simulink model "cubli_XYZ_extensive_simulations"  (R2016a)
(part 4 of 9)

  1/2).*t.*theta)).*(q02.*sin((1/2).*(1+(-1).*t).*theta)+q12.*sin((1/2).* ...
  t.*theta))+csc((1/2).*theta).^2.*(q03.*sin((1/2).*(1+(-1).*t).*theta)+ ...
  q13.*sin((1/2).*t.*theta)).*(q04.*sin((1/2).*(1+(-1).*t).*theta)+q14.* ...
  sin((1/2).*t.*theta)))+(-4).*(2.*((-1/2).*q02.*theta.*cos((1/2).*(1+(-1) ...
  .*t).*theta)+(1/2).*q12.*theta.*cos((1/2).*t.*theta)).*csc((1/2).*theta) ...
  .^2.*(q02.*sin((1/2).*(1+(-1).*t).*theta)+q12.*sin((1/2).*t.*theta))+2.* ...
  ((-1/2).*q03.*theta.*cos((1/2).*(1+(-1).*t).*theta)+(1/2).*q13.*theta.* ...
  cos((1/2).*t.*theta)).*csc((1/2).*theta).^2.*(q03.*sin((1/2).*(1+(-1).* ...
  t).*theta)+q13.*sin((1/2).*t.*theta))).*(1+(-2).*(csc((1/2).*theta).^2.* ...
  (q02.*sin((1/2).*(1+(-1).*t).*theta)+q12.*sin((1/2).*t.*theta)).^2+csc(( ...
  1/2).*theta).^2.*(q03.*sin((1/2).*(1+(-1).*t).*theta)+q13.*sin((1/2).* ...
  t.*theta)).^2))).*(4.*((-1).*csc((1/2).*theta).^2.*(q01.*sin((1/2).*(1+( ...
  -1).*t).*theta)+q11.*sin((1/2).*t.*theta)).*(q02.*sin((1/2).*(1+(-1).*t) ...
  .*theta)+q12.*sin((1/2).*t.*theta))+csc((1/2).*theta).^2.*(q03.*sin(( ...
  1/2).*(1+(-1).*t).*theta)+q13.*sin((1/2).*t.*theta)).*(q04.*sin((1/2).*( ...
  1+(-1).*t).*theta)+q14.*sin((1/2).*t.*theta))).^2+(1+(-2).*(csc((1/2).* ...
  theta).^2.*(q02.*sin((1/2).*(1+(-1).*t).*theta)+q12.*sin((1/2).*t.* ...
  theta)).^2+csc((1/2).*theta).^2.*(q03.*sin((1/2).*(1+(-1).*t).*theta)+ ...
  q13.*sin((1/2).*t.*theta)).^2)).^2).^(-1/2).*(4.*(csc((1/2).*theta).^2.* ...
  (q01.*sin((1/2).*(1+(-1).*t).*theta)+q11.*sin((1/2).*t.*theta)).*(q03.* ...
  sin((1/2).*(1+(-1).*t).*theta)+q13.*sin((1/2).*t.*theta))+csc((1/2).* ...
  theta).^2.*(q02.*sin((1/2).*(1+(-1).*t).*theta)+q12.*sin((1/2).*t.* ...
  theta)).*(q04.*sin((1/2).*(1+(-1).*t).*theta)+q14.*sin((1/2).*t.*theta)) ...
  ).^2+4.*((-1).*csc((1/2).*theta).^2.*(q01.*sin((1/2).*(1+(-1).*t).* ...
  theta)+q11.*sin((1/2).*t.*theta)).*(q02.*sin((1/2).*(1+(-1).*t).*theta)+ ...
  q12.*sin((1/2).*t.*theta))+csc((1/2).*theta).^2.*(q03.*sin((1/2).*(1+( ...
  -1).*t).*theta)+q13.*sin((1/2).*t.*theta)).*(q04.*sin((1/2).*(1+(-1).*t) ...
  .*theta)+q14.*sin((1/2).*t.*theta))).^2+(1+(-2).*(csc((1/2).*theta).^2.* ...
  (q02.*sin((1/2).*(1+(-1).*t).*theta)+q12.*sin((1/2).*t.*theta)).^2+csc(( ...
  1/2).*theta).^2.*(q03.*sin((1/2).*(1+(-1).*t).*theta)+q13.*sin((1/2).* ...
  t.*theta)).^2)).^2).^(-1/2)+(csc((1/2).*theta).^2.*(q02.*sin((1/2).*(1+( ...
  -1).*t).*theta)+q12.*sin((1/2).*t.*theta)).*(q03.*sin((1/2).*(1+(-1).*t) ...
  .*theta)+q13.*sin((1/2).*t.*theta))+(-1).*csc((1/2).*theta).^2.*(q01.* ...
  sin((1/2).*(1+(-1).*t).*theta)+q11.*sin((1/2).*t.*theta)).*(q04.*sin(( ...
  1/2).*(1+(-1).*t).*theta)+q14.*sin((1/2).*t.*theta))).*(8.*((-1).*(( ...
  -1/2).*q02.*theta.*cos((1/2).*(1+(-1).*t).*theta)+(1/2).*q12.*theta.* ...
  cos((1/2).*t.*theta)).*csc((1/2).*theta).^2.*(q01.*sin((1/2).*(1+(-1).* ...
  t).*theta)+q11.*sin((1/2).*t.*theta))+(-1).*((-1/2).*q01.*theta.*cos(( ...
  1/2).*(1+(-1).*t).*theta)+(1/2).*q11.*theta.*cos((1/2).*t.*theta)).*csc( ...
  (1/2).*theta).^2.*(q02.*sin((1/2).*(1+(-1).*t).*theta)+q12.*sin((1/2).* ...
  t.*theta))+((-1/2).*q04.*theta.*cos((1/2).*(1+(-1).*t).*theta)+(1/2).* ...
  q14.*theta.*cos((1/2).*t.*theta)).*csc((1/2).*theta).^2.*(q03.*sin((1/2) ...
  .*(1+(-1).*t).*theta)+q13.*sin((1/2).*t.*theta))+((-1/2).*q03.*theta.* ...
  cos((1/2).*(1+(-1).*t).*theta)+(1/2).*q13.*theta.*cos((1/2).*t.*theta)) ...
  .*csc((1/2).*theta).^2.*(q04.*sin((1/2).*(1+(-1).*t).*theta)+q14.*sin(( ...
  1/2).*t.*theta))).*((-1).*csc((1/2).*theta).^2.*(q01.*sin((1/2).*(1+(-1) ...
  .*t).*theta)+q11.*sin((1/2).*t.*theta)).*(q02.*sin((1/2).*(1+(-1).*t).* ...
  theta)+q12.*sin((1/2).*t.*theta))+csc((1/2).*theta).^2.*(q03.*sin((1/2) ...
  .*(1+(-1).*t).*theta)+q13.*sin((1/2).*t.*theta)).*(q04.*sin((1/2).*(1+( ...
  -1).*t).*theta)+q14.*sin((1/2).*t.*theta)))+(-4).*(2.*((-1/2).*q02.* ...
  theta.*cos((1/2).*(1+(-1).*t).*theta)+(1/2).*q12.*theta.*cos((1/2).*t.* ...
  theta)).*csc((1/2).*theta).^2.*(q02.*sin((1/2).*(1+(-1).*t).*theta)+ ...
  q12.*sin((1/2).*t.*theta))+2.*((-1/2).*q03.*theta.*cos((1/2).*(1+(-1).* ...
  t).*theta)+(1/2).*q13.*theta.*cos((1/2).*t.*theta)).*csc((1/2).*theta) ...
  .^2.*(q03.*sin((1/2).*(1+(-1).*t).*theta)+q13.*sin((1/2).*t.*theta))).*( ...
  1+(-2).*(csc((1/2).*theta).^2.*(q02.*sin((1/2).*(1+(-1).*t).*theta)+ ...
  q12.*sin((1/2).*t.*theta)).^2+csc((1/2).*theta).^2.*(q03.*sin((1/2).*(1+ ...
  (-1).*t).*theta)+q13.*sin((1/2).*t.*theta)).^2))).*(4.*((-1).*csc((1/2) ...
  .*theta).^2.*(q01.*sin((1/2).*(1+(-1).*t).*theta)+q11.*sin((1/2).*t.* ...
  theta)).*(q02.*sin((1/2).*(1+(-1).*t).*theta)+q12.*sin((1/2).*t.*theta)) ...
  +csc((1/2).*theta).^2.*(q03.*sin((1/2).*(1+(-1).*t).*theta)+q13.*sin(( ...
  1/2).*t.*theta)).*(q04.*sin((1/2).*(1+(-1).*t).*theta)+q14.*sin((1/2).* ...
  t.*theta))).^2+(1+(-2).*(csc((1/2).*theta).^2.*(q02.*sin((1/2).*(1+(-1) ...
  .*t).*theta)+q12.*sin((1/2).*t.*theta)).^2+csc((1/2).*theta).^2.*(q03.* ...
  sin((1/2).*(1+(-1).*t).*theta)+q13.*sin((1/2).*t.*theta)).^2)).^2).^( ...
  -3/2).*(4.*(csc((1/2).*theta).^2.*(q01.*sin((1/2).*(1+(-1).*t).*theta)+ ...
  q11.*sin((1/2).*t.*theta)).*(q03.*sin((1/2).*(1+(-1).*t).*theta)+q13.* ...
  sin((1/2).*t.*theta))+csc((1/2).*theta).^2.*(q02.*sin((1/2).*(1+(-1).*t) ...
  .*theta)+q12.*sin((1/2).*t.*theta)).*(q04.*sin((1/2).*(1+(-1).*t).* ...
  theta)+q14.*sin((1/2).*t.*theta))).^2+4.*((-1).*csc((1/2).*theta).^2.*( ...
  q01.*sin((1/2).*(1+(-1).*t).*theta)+q11.*sin((1/2).*t.*theta)).*(q02.* ...
  sin((1/2).*(1+(-1).*t).*theta)+q12.*sin((1/2).*t.*theta))+csc((1/2).* ...
  theta).^2.*(q03.*sin((1/2).*(1+(-1).*t).*theta)+q13.*sin((1/2).*t.* ...
  theta)).*(q04.*sin((1/2).*(1+(-1).*t).*theta)+q14.*sin((1/2).*t.*theta)) ...
  ).^2+(1+(-2).*(csc((1/2).*theta).^2.*(q02.*sin((1/2).*(1+(-1).*t).* ...
  theta)+q12.*sin((1/2).*t.*theta)).^2+csc((1/2).*theta).^2.*(q03.*sin(( ...
  1/2).*(1+(-1).*t).*theta)+q13.*sin((1/2).*t.*theta)).^2)).^2).^(1/2)+( ...
  -2).*((-1).*((-1/2).*q04.*theta.*cos((1/2).*(1+(-1).*t).*theta)+(1/2).* ...
  q14.*theta.*cos((1/2).*t.*theta)).*csc((1/2).*theta).^2.*(q01.*sin((1/2) ...
  .*(1+(-1).*t).*theta)+q11.*sin((1/2).*t.*theta))+((-1/2).*q03.*theta.* ...
  cos((1/2).*(1+(-1).*t).*theta)+(1/2).*q13.*theta.*cos((1/2).*t.*theta)) ...
  .*csc((1/2).*theta).^2.*(q02.*sin((1/2).*(1+(-1).*t).*theta)+q12.*sin(( ...
  1/2).*t.*theta))+((-1/2).*q02.*theta.*cos((1/2).*(1+(-1).*t).*theta)+( ...
  1/2).*q12.*theta.*cos((1/2).*t.*theta)).*csc((1/2).*theta).^2.*(q03.* ...
  sin((1/2).*(1+(-1).*t).*theta)+q13.*sin((1/2).*t.*theta))+(-1).*((-1/2) ...
  .*q01.*theta.*cos((1/2).*(1+(-1).*t).*theta)+(1/2).*q11.*theta.*cos(( ...
  1/2).*t.*theta)).*csc((1/2).*theta).^2.*(q04.*sin((1/2).*(1+(-1).*t).* ...
  theta)+q14.*sin((1/2).*t.*theta))).*(4.*((-1).*csc((1/2).*theta).^2.*( ...
  q01.*sin((1/2).*(1+(-1).*t).*theta)+q11.*sin((1/2).*t.*theta)).*(q02.* ...
  sin((1/2).*(1+(-1).*t).*theta)+q12.*sin((1/2).*t.*theta))+csc((1/2).* ...
  theta).^2.*(q03.*sin((1/2).*(1+(-1).*t).*theta)+q13.*sin((1/2).*t.* ...
  theta)).*(q04.*sin((1/2).*(1+(-1).*t).*theta)+q14.*sin((1/2).*t.*theta)) ...
  ).^2+(1+(-2).*(csc((1/2).*theta).^2.*(q02.*sin((1/2).*(1+(-1).*t).* ...
  theta)+q12.*sin((1/2).*t.*theta)).^2+csc((1/2).*theta).^2.*(q03.*sin(( ...
  1/2).*(1+(-1).*t).*theta)+q13.*sin((1/2).*t.*theta)).^2)).^2).^(-1/2).*( ...
  4.*(csc((1/2).*theta).^2.*(q01.*sin((1/2).*(1+(-1).*t).*theta)+q11.*sin( ...
  (1/2).*t.*theta)).*(q03.*sin((1/2).*(1+(-1).*t).*theta)+q13.*sin((1/2).* ...
  t.*theta))+csc((1/2).*theta).^2.*(q02.*sin((1/2).*(1+(-1).*t).*theta)+ ...
  q12.*sin((1/2).*t.*theta)).*(q04.*sin((1/2).*(1+(-1).*t).*theta)+q14.* ...
  sin((1/2).*t.*theta))).^2+4.*((-1).*csc((1/2).*theta).^2.*(q01.*sin(( ...
  1/2).*(1+(-1).*t).*theta)+q11.*sin((1/2).*t.*theta)).*(q02.*sin((1/2).*( ...
  1+(-1).*t).*theta)+q12.*sin((1/2).*t.*theta))+csc((1/2).*theta).^2.*( ...
  q03.*sin((1/2).*(1+(-1).*t).*theta)+q13.*sin((1/2).*t.*theta)).*(q04.* ...
  sin((1/2).*(1+(-1).*t).*theta)+q14.*sin((1/2).*t.*theta))).^2+(1+(-2).*( ...
  csc((1/2).*theta).^2.*(q02.*sin((1/2).*(1+(-1).*t).*theta)+q12.*sin(( ...
  1/2).*t.*theta)).^2+csc((1/2).*theta).^2.*(q03.*sin((1/2).*(1+(-1).*t).* ...
  theta)+q13.*sin((1/2).*t.*theta)).^2)).^2).^(1/2)).*(4.*(csc((1/2).* ...
  theta).^2.*(q02.*sin((1/2).*(1+(-1).*t).*theta)+q12.*sin((1/2).*t.* ...
  theta)).*(q03.*sin((1/2).*(1+(-1).*t).*theta)+q13.*sin((1/2).*t.*theta)) ...
  +(-1).*csc((1/2).*theta).^2.*(q01.*sin((1/2).*(1+(-1).*t).*theta)+q11.* ...
  sin((1/2).*t.*theta)).*(q04.*sin((1/2).*(1+(-1).*t).*theta)+q14.*sin(( ...
  1/2).*t.*theta))).^2.*(4.*((-1).*csc((1/2).*theta).^2.*(q01.*sin((1/2).* ...
  (1+(-1).*t).*theta)+q11.*sin((1/2).*t.*theta)).*(q02.*sin((1/2).*(1+(-1) ...
  .*t).*theta)+q12.*sin((1/2).*t.*theta))+csc((1/2).*theta).^2.*(q03.*sin( ...
  (1/2).*(1+(-1).*t).*theta)+q13.*sin((1/2).*t.*theta)).*(q04.*sin((1/2).* ...
  (1+(-1).*t).*theta)+q14.*sin((1/2).*t.*theta))).^2+(1+(-2).*(csc((1/2).* ...
  theta).^2.*(q02.*sin((1/2).*(1+(-1).*t).*theta)+q12.*sin((1/2).*t.* ...
  theta)).^2+csc((1/2).*theta).^2.*(q03.*sin((1/2).*(1+(-1).*t).*theta)+ ...
  q13.*sin((1/2).*t.*theta)).^2)).^2).^(-1).*(4.*(csc((1/2).*theta).^2.*( ...
  q01.*sin((1/2).*(1+(-1).*t).*theta)+q11.*sin((1/2).*t.*theta)).*(q03.* ...
  sin((1/2).*(1+(-1).*t).*theta)+q13.*sin((1/2).*t.*theta))+csc((1/2).* ...
  theta).^2.*(q02.*sin((1/2).*(1+(-1).*t).*theta)+q12.*sin((1/2).*t.* ...
  theta)).*(q04.*sin((1/2).*(1+(-1).*t).*theta)+q14.*sin((1/2).*t.*theta)) ...
  ).^2+4.*((-1).*csc((1/2).*theta).^2.*(q01.*sin((1/2).*(1+(-1).*t).* ...
  theta)+q11.*sin((1/2).*t.*theta)).*(q02.*sin((1/2).*(1+(-1).*t).*theta)+ ...
  q12.*sin((1/2).*t.*theta))+csc((1/2).*theta).^2.*(q03.*sin((1/2).*(1+( ...
  -1).*t).*theta)+q13.*sin((1/2).*t.*theta)).*(q04.*sin((1/2).*(1+(-1).*t) ...
  .*theta)+q14.*sin((1/2).*t.*theta))).^2+(1+(-2).*(csc((1/2).*theta).^2.* ...
  (q02.*sin((1/2).*(1+(-1).*t).*theta)+q12.*sin((1/2).*t.*theta)).^2+csc(( ...
  1/2).*theta).^2.*(q03.*sin((1/2).*(1+(-1).*t).*theta)+q13.*sin((1/2).* ...
  t.*theta)).^2)).^2)+(1+(-2).*(csc((1/2).*theta).^2.*(q03.*sin((1/2).*(1+ ...
  (-1).*t).*theta)+q13.*sin((1/2).*t.*theta)).^2+csc((1/2).*theta).^2.*( ...
  q04.*sin((1/2).*(1+(-1).*t).*theta)+q14.*sin((1/2).*t.*theta)).^2)).^2.* ...
  (4.*((-1).*csc((1/2).*theta).^2.*(q01.*sin((1/2).*(1+(-1).*t).*theta)+ ...
  q11.*sin((1/2).*t.*theta)).*(q02.*sin((1/2).*(1+(-1).*t).*theta)+q12.* ...
  sin((1/2).*t.*theta))+csc((1/2).*theta).^2.*(q03.*sin((1/2).*(1+(-1).*t) ...
  .*theta)+q13.*sin((1/2).*t.*theta)).*(q04.*sin((1/2).*(1+(-1).*t).* ...
  theta)+q14.*sin((1/2).*t.*theta))).^2+(1+(-2).*(csc((1/2).*theta).^2.*( ...
  q02.*sin((1/2).*(1+(-1).*t).*theta)+q12.*sin((1/2).*t.*theta)).^2+csc(( ...
  1/2).*theta).^2.*(q03.*sin((1/2).*(1+(-1).*t).*theta)+q13.*sin((1/2).* ...
  t.*theta)).^2)).^2).^(-1).*(4.*(csc((1/2).*theta).^2.*(q01.*sin((1/2).*( ...
  1+(-1).*t).*theta)+q11.*sin((1/2).*t.*theta)).*(q03.*sin((1/2).*(1+(-1) ...
  .*t).*theta)+q13.*sin((1/2).*t.*theta))+csc((1/2).*theta).^2.*(q02.*sin( ...
  (1/2).*(1+(-1).*t).*theta)+q12.*sin((1/2).*t.*theta)).*(q04.*sin((1/2).* ...
  (1+(-1).*t).*theta)+q14.*sin((1/2).*t.*theta))).^2+4.*((-1).*csc((1/2).* ...
  theta).^2.*(q01.*sin((1/2).*(1+(-1).*t).*theta)+q11.*sin((1/2).*t.* ...
  theta)).*(q02.*sin((1/2).*(1+(-1).*t).*theta)+q12.*sin((1/2).*t.*theta)) ...
  +csc((1/2).*theta).^2.*(q03.*sin((1/2).*(1+(-1).*t).*theta)+q13.*sin(( ...
  1/2).*t.*theta)).*(q04.*sin((1/2).*(1+(-1).*t).*theta)+q14.*sin((1/2).* ...
  t.*theta))).^2+(1+(-2).*(csc((1/2).*theta).^2.*(q02.*sin((1/2).*(1+(-1) ...
  .*t).*theta)+q12.*sin((1/2).*t.*theta)).^2+csc((1/2).*theta).^2.*(q03.* ...
  sin((1/2).*(1+(-1).*t).*theta)+q13.*sin((1/2).*t.*theta)).^2)).^2)).^( ...
  -1)+(-1/2).*(1+(-2).*(csc((1/2).*theta).^2.*(q03.*sin((1/2).*(1+(-1).*t) ...
  .*theta)+q13.*sin((1/2).*t.*theta)).^2+csc((1/2).*theta).^2.*(q04.*sin(( ...
  1/2).*(1+(-1).*t).*theta)+q14.*sin((1/2).*t.*theta)).^2)).*(8.*((-1).*(( ...
  -1/2).*q02.*theta.*cos((1/2).*(1+(-1).*t).*theta)+(1/2).*q12.*theta.* ...
  cos((1/2).*t.*theta)).*csc((1/2).*theta).^2.*(q01.*sin((1/2).*(1+(-1).* ...
  t).*theta)+q11.*sin((1/2).*t.*theta))+(-1).*((-1/2).*q01.*theta.*cos(( ...
  1/2).*(1+(-1).*t).*theta)+(1/2).*q11.*theta.*cos((1/2).*t.*theta)).*csc( ...
  (1/2).*theta).^2.*(q02.*sin((1/2).*(1+(-1).*t).*theta)+q12.*sin((1/2).* ...
  t.*theta))+((-1/2).*q04.*theta.*cos((1/2).*(1+(-1).*t).*theta)+(1/2).* ...
  q14.*theta.*cos((1/2).*t.*theta)).*csc((1/2).*theta).^2.*(q03.*sin((1/2) ...
  .*(1+(-1).*t).*theta)+q13.*sin((1/2).*t.*theta))+((-1/2).*q03.*theta.* ...
  cos((1/2).*(1+(-1).*t).*theta)+(1/2).*q13.*theta.*cos((1/2).*t.*theta)) ...
  .*csc((1/2).*theta).^2.*(q04.*sin((1/2).*(1+(-1).*t).*theta)+q14.*sin(( ...
  1/2).*t.*theta))).*((-1).*csc((1/2).*theta).^2.*(q01.*sin((1/2).*(1+(-1) ...
  .*t).*theta)+q11.*sin((1/2).*t.*theta)).*(q02.*sin((1/2).*(1+(-1).*t).* ...
  theta)+q12.*sin((1/2).*t.*theta))+csc((1/2).*theta).^2.*(q03.*sin((1/2) ...
  .*(1+(-1).*t).*theta)+q13.*sin((1/2).*t.*theta)).*(q04.*sin((1/2).*(1+( ...
  -1).*t).*theta)+q14.*sin((1/2).*t.*theta)))+(-4).*(2.*((-1/2).*q02.* ...
  theta.*cos((1/2).*(1+(-1).*t).*theta)+(1/2).*q12.*theta.*cos((1/2).*t.* ...
  theta)).*csc((1/2).*theta).^2.*(q02.*sin((1/2).*(1+(-1).*t).*theta)+ ...
  q12.*sin((1/2).*t.*theta))+2.*((-1/2).*q03.*theta.*cos((1/2).*(1+(-1).* ...
  t).*theta)+(1/2).*q13.*theta.*cos((1/2).*t.*theta)).*csc((1/2).*theta) ...
  .^2.*(q03.*sin((1/2).*(1+(-1).*t).*theta)+q13.*sin((1/2).*t.*theta))).*( ...
  1+(-2).*(csc((1/2).*theta).^2.*(q02.*sin((1/2).*(1+(-1).*t).*theta)+ ...
  q12.*sin((1/2).*t.*theta)).^2+csc((1/2).*theta).^2.*(q03.*sin((1/2).*(1+ ...
  (-1).*t).*theta)+q13.*sin((1/2).*t.*theta)).^2))).*(4.*((-1).*csc((1/2) ...
  .*theta).^2.*(q01.*sin((1/2).*(1+(-1).*t).*theta)+q11.*sin((1/2).*t.* ...
  theta)).*(q02.*sin((1/2).*(1+(-1).*t).*theta)+q12.*sin((1/2).*t.*theta)) ...
  +csc((1/2).*theta).^2.*(q03.*sin((1/2).*(1+(-1).*t).*theta)+q13.*sin(( ...
  1/2).*t.*theta)).*(q04.*sin((1/2).*(1+(-1).*t).*theta)+q14.*sin((1/2).* ...
  t.*theta))).^2+(1+(-2).*(csc((1/2).*theta).^2.*(q02.*sin((1/2).*(1+(-1) ...
  .*t).*theta)+q12.*sin((1/2).*t.*theta)).^2+csc((1/2).*theta).^2.*(q03.* ...
  sin((1/2).*(1+(-1).*t).*theta)+q13.*sin((1/2).*t.*theta)).^2)).^2).^( ...
  -3/2).*(4.*(csc((1/2).*theta).^2.*(q01.*sin((1/2).*(1+(-1).*t).*theta)+ ...
  q11.*sin((1/2).*t.*theta)).*(q03.*sin((1/2).*(1+(-1).*t).*theta)+q13.* ...
  sin((1/2).*t.*theta))+csc((1/2).*theta).^2.*(q02.*sin((1/2).*(1+(-1).*t) ...
  .*theta)+q12.*sin((1/2).*t.*theta)).*(q04.*sin((1/2).*(1+(-1).*t).* ...
  theta)+q14.*sin((1/2).*t.*theta))).^2+4.*((-1).*csc((1/2).*theta).^2.*( ...
  q01.*sin((1/2).*(1+(-1).*t).*theta)+q11.*sin((1/2).*t.*theta)).*(q02.* ...
  sin((1/2).*(1+(-1).*t).*theta)+q12.*sin((1/2).*t.*theta))+csc((1/2).* ...
  theta).^2.*(q03.*sin((1/2).*(1+(-1).*t).*theta)+q13.*sin((1/2).*t.* ...
  theta)).*(q04.*sin((1/2).*(1+(-1).*t).*theta)+q14.*sin((1/2).*t.*theta)) ...
  ).^2+(1+(-2).*(csc((1/2).*theta).^2.*(q02.*sin((1/2).*(1+(-1).*t).* ...
  theta)+q12.*sin((1/2).*t.*theta)).^2+csc((1/2).*theta).^2.*(q03.*sin(( ...
  1/2).*(1+(-1).*t).*theta)+q13.*sin((1/2).*t.*theta)).^2)).^2).^(1/2).*(( ...
  -1).*(csc((1/2).*theta).^2.*(q02.*sin((1/2).*(1+(-1).*t).*theta)+q12.* ...
  sin((1/2).*t.*theta)).*(q03.*sin((1/2).*(1+(-1).*t).*theta)+q13.*sin(( ...
  1/2).*t.*theta))+(-1).*csc((1/2).*theta).^2.*(q01.*sin((1/2).*(1+(-1).* ...
  t).*theta)+q11.*sin((1/2).*t.*theta)).*(q04.*sin((1/2).*(1+(-1).*t).* ...
  theta)+q14.*sin((1/2).*t.*theta))).*(8.*(((-1/2).*q03.*theta.*cos((1/2) ...
  .*(1+(-1).*t).*theta)+(1/2).*q13.*theta.*cos((1/2).*t.*theta)).*csc(( ...
  1/2).*theta).^2.*(q01.*sin((1/2).*(1+(-1).*t).*theta)+q11.*sin((1/2).* ...
  t.*theta))+((-1/2).*q04.*theta.*cos((1/2).*(1+(-1).*t).*theta)+(1/2).* ...
  q14.*theta.*cos((1/2).*t.*theta)).*csc((1/2).*theta).^2.*(q02.*sin((1/2) ...
  .*(1+(-1).*t).*theta)+q12.*sin((1/2).*t.*theta))+((-1/2).*q01.*theta.* ...
  cos((1/2).*(1+(-1).*t).*theta)+(1/2).*q11.*theta.*cos((1/2).*t.*theta)) ...
  .*csc((1/2).*theta).^2.*(q03.*sin((1/2).*(1+(-1).*t).*theta)+q13.*sin(( ...
  1/2).*t.*theta))+((-1/2).*q02.*theta.*cos((1/2).*(1+(-1).*t).*theta)+( ...
  1/2).*q12.*theta.*cos((1/2).*t.*theta)).*csc((1/2).*theta).^2.*(q04.* ...
  sin((1/2).*(1+(-1).*t).*theta)+q14.*sin((1/2).*t.*theta))).*(csc((1/2).* ...
  theta).^2.*(q01.*sin((1/2).*(1+(-1).*t).*theta)+q11.*sin((1/2).*t.* ...
  theta)).*(q03.*sin((1/2).*(1+(-1).*t).*theta)+q13.*sin((1/2).*t.*theta)) ...
  +csc((1/2).*theta).^2.*(q02.*sin((1/2).*(1+(-1).*t).*theta)+q12.*sin(( ...
  1/2).*t.*theta)).*(q04.*sin((1/2).*(1+(-1).*t).*theta)+q14.*sin((1/2).* ...
  t.*theta)))+8.*((-1).*((-1/2).*q02.*theta.*cos((1/2).*(1+(-1).*t).* ...
  theta)+(1/2).*q12.*theta.*cos((1/2).*t.*theta)).*csc((1/2).*theta).^2.*( ...
  q01.*sin((1/2).*(1+(-1).*t).*theta)+q11.*sin((1/2).*t.*theta))+(-1).*(( ...
  -1/2).*q01.*theta.*cos((1/2).*(1+(-1).*t).*theta)+(1/2).*q11.*theta.* ...
  cos((1/2).*t.*theta)).*csc((1/2).*theta).^2.*(q02.*sin((1/2).*(1+(-1).* ...
  t).*theta)+q12.*sin((1/2).*t.*theta))+((-1/2).*q04.*theta.*cos((1/2).*( ...
  1+(-1).*t).*theta)+(1/2).*q14.*theta.*cos((1/2).*t.*theta)).*csc((1/2).* ...
  theta).^2.*(q03.*sin((1/2).*(1+(-1).*t).*theta)+q13.*sin((1/2).*t.* ...
  theta))+((-1/2).*q03.*theta.*cos((1/2).*(1+(-1).*t).*theta)+(1/2).*q13.* ...
  theta.*cos((1/2).*t.*theta)).*csc((1/2).*theta).^2.*(q04.*sin((1/2).*(1+ ...
  (-1).*t).*theta)+q14.*sin((1/2).*t.*theta))).*((-1).*csc((1/2).*theta) ...
  .^2.*(q01.*sin((1/2).*(1+(-1).*t).*theta)+q11.*sin((1/2).*t.*theta)).*( ...
  q02.*sin((1/2).*(1+(-1).*t).*theta)+q12.*sin((1/2).*t.*theta))+csc((1/2) ...
  .*theta).^2.*(q03.*sin((1/2).*(1+(-1).*t).*theta)+q13.*sin((1/2).*t.* ...
  theta)).*(q04.*sin((1/2).*(1+(-1).*t).*theta)+q14.*sin((1/2).*t.*theta)) ...
  )+(-4).*(2.*((-1/2).*q02.*theta.*cos((1/2).*(1+(-1).*t).*theta)+(1/2).* ...
  q12.*theta.*cos((1/2).*t.*theta)).*csc((1/2).*theta).^2.*(q02.*sin((1/2) ...
  .*(1+(-1).*t).*theta)+q12.*sin((1/2).*t.*theta))+2.*((-1/2).*q03.* ...
  theta.*cos((1/2).*(1+(-1).*t).*theta)+(1/2).*q13.*theta.*cos((1/2).*t.* ...
  theta)).*csc((1/2).*theta).^2.*(q03.*sin((1/2).*(1+(-1).*t).*theta)+ ...
  q13.*sin((1/2).*t.*theta))).*(1+(-2).*(csc((1/2).*theta).^2.*(q02.*sin(( ...
  1/2).*(1+(-1).*t).*theta)+q12.*sin((1/2).*t.*theta)).^2+csc((1/2).* ...
  theta).^2.*(q03.*sin((1/2).*(1+(-1).*t).*theta)+q13.*sin((1/2).*t.* ...
  theta)).^2))).*(4.*((-1).*csc((1/2).*theta).^2.*(q01.*sin((1/2).*(1+(-1) ...
  .*t).*theta)+q11.*sin((1/2).*t.*theta)).*(q02.*sin((1/2).*(1+(-1).*t).* ...
  theta)+q12.*sin((1/2).*t.*theta))+csc((1/2).*theta).^2.*(q03.*sin((1/2) ...
  .*(1+(-1).*t).*theta)+q13.*sin((1/2).*t.*theta)).*(q04.*sin((1/2).*(1+( ...
  -1).*t).*theta)+q14.*sin((1/2).*t.*theta))).^2+(1+(-2).*(csc((1/2).* ...
  theta).^2.*(q02.*sin((1/2).*(1+(-1).*t).*theta)+q12.*sin((1/2).*t.* ...
  theta)).^2+csc((1/2).*theta).^2.*(q03.*sin((1/2).*(1+(-1).*t).*theta)+ ...
  q13.*sin((1/2).*t.*theta)).^2)).^2).^(-1/2).*(4.*(csc((1/2).*theta).^2.* ...
  (q01.*sin((1/2).*(1+(-1).*t).*theta)+q11.*sin((1/2).*t.*theta)).*(q03.* ...
  sin((1/2).*(1+(-1).*t).*theta)+q13.*sin((1/2).*t.*theta))+csc((1/2).* ...
  theta).^2.*(q02.*sin((1/2).*(1+(-1).*t).*theta)+q12.*sin((1/2).*t.* ...
  theta)).*(q04.*sin((1/2).*(1+(-1).*t).*theta)+q14.*sin((1/2).*t.*theta)) ...
  ).^2+4.*((-1).*csc((1/2).*theta).^2.*(q01.*sin((1/2).*(1+(-1).*t).* ...
  theta)+q11.*sin((1/2).*t.*theta)).*(q02.*sin((1/2).*(1+(-1).*t).*theta)+ ...
  q12.*sin((1/2).*t.*theta))+csc((1/2).*theta).^2.*(q03.*sin((1/2).*(1+( ...
  -1).*t).*theta)+q13.*sin((1/2).*t.*theta)).*(q04.*sin((1/2).*(1+(-1).*t) ...
  .*theta)+q14.*sin((1/2).*t.*theta))).^2+(1+(-2).*(csc((1/2).*theta).^2.* ...
  (q02.*sin((1/2).*(1+(-1).*t).*theta)+q12.*sin((1/2).*t.*theta)).^2+csc(( ...
  1/2).*theta).^2.*(q03.*sin((1/2).*(1+(-1).*t).*theta)+q13.*sin((1/2).* ...
  t.*theta)).^2)).^2).^(-1/2)+(csc((1/2).*theta).^2.*(q02.*sin((1/2).*(1+( ...
  -1).*t).*theta)+q12.*sin((1/2).*t.*theta)).*(q03.*sin((1/2).*(1+(-1).*t) ...
  .*theta)+q13.*sin((1/2).*t.*theta))+(-1).*csc((1/2).*theta).^2.*(q01.* ...
  sin((1/2).*(1+(-1).*t).*theta)+q11.*sin((1/2).*t.*theta)).*(q04.*sin(( ...
  1/2).*(1+(-1).*t).*theta)+q14.*sin((1/2).*t.*theta))).*(8.*((-1).*(( ...
  -1/2).*q02.*theta.*cos((1/2).*(1+(-1).*t).*theta)+(1/2).*q12.*theta.* ...
  cos((1/2).*t.*theta)).*csc((1/2).*theta).^2.*(q01.*sin((1/2).*(1+(-1).* ...
  t).*theta)+q11.*sin((1/2).*t.*theta))+(-1).*((-1/2).*q01.*theta.*cos(( ...
  1/2).*(1+(-1).*t).*theta)+(1/2).*q11.*theta.*cos((1/2).*t.*theta)).*csc( ...
  (1/2).*theta).^2.*(q02.*sin((1/2).*(1+(-1).*t).*theta)+q12.*sin((1/2).* ...
  t.*theta))+((-1/2).*q04.*theta.*cos((1/2).*(1+(-1).*t).*theta)+(1/2).* ...
  q14.*theta.*cos((1/2).*t.*theta)).*csc((1/2).*theta).^2.*(q03.*sin((1/2) ...
  .*(1+(-1).*t).*theta)+q13.*sin((1/2).*t.*theta))+((-1/2).*q03.*theta.* ...
  cos((1/2).*(1+(-1).*t).*theta)+(1/2).*q13.*theta.*cos((1/2).*t.*theta)) ...
  .*csc((1/2).*theta).^2.*(q04.*sin((1/2).*(1+(-1).*t).*theta)+q14.*sin(( ...
  1/2).*t.*theta))).*((-1).*csc((1/2).*theta).^2.*(q01.*sin((1/2).*(1+(-1) ...
  .*t).*theta)+q11.*sin((1/2).*t.*theta)).*(q02.*sin((1/2).*(1+(-1).*t).* ...
  theta)+q12.*sin((1/2).*t.*theta))+csc((1/2).*theta).^2.*(q03.*sin((1/2) ...
  .*(1+(-1).*t).*theta)+q13.*sin((1/2).*t.*theta)).*(q04.*sin((1/2).*(1+( ...
  -1).*t).*theta)+q14.*sin((1/2).*t.*theta)))+(-4).*(2.*((-1/2).*q02.* ...
  theta.*cos((1/2).*(1+(-1).*t).*theta)+(1/2).*q12.*theta.*cos((1/2).*t.* ...
  theta)).*csc((1/2).*theta).^2.*(q02.*sin((1/2).*(1+(-1).*t).*theta)+ ...
  q12.*sin((1/2).*t.*theta))+2.*((-1/2).*q03.*theta.*cos((1/2).*(1+(-1).* ...
  t).*theta)+(1/2).*q13.*theta.*cos((1/2).*t.*theta)).*csc((1/2).*theta) ...
  .^2.*(q03.*sin((1/2).*(1+(-1).*t).*theta)+q13.*sin((1/2).*t.*theta))).*( ...
  1+(-2).*(csc((1/2).*theta).^2.*(q02.*sin((1/2).*(1+(-1).*t).*theta)+ ...
  q12.*sin((1/2).*t.*theta)).^2+csc((1/2).*theta).^2.*(q03.*sin((1/2).*(1+ ...
  (-1).*t).*theta)+q13.*sin((1/2).*t.*theta)).^2))).*(4.*((-1).*csc((1/2) ...
  .*theta).^2.*(q01.*sin((1/2).*(1+(-1).*t).*theta)+q11.*sin((1/2).*t.* ...
  theta)).*(q02.*sin((1/2).*(1+(-1).*t).*theta)+q12.*sin((1/2).*t.*theta)) ...
  +csc((1/2).*theta).^2.*(q03.*sin((1/2).*(1+(-1).*t).*theta)+q13.*sin(( ...
  1/2).*t.*theta)).*(q04.*sin((1/2).*(1+(-1).*t).*theta)+q14.*sin((1/2).* ...
  t.*theta))).^2+(1+(-2).*(csc((1/2).*theta).^2.*(q02.*sin((1/2).*(1+(-1) ...
  .*t).*theta)+q12.*sin((1/2).*t.*theta)).^2+csc((1/2).*theta).^2.*(q03.* ...
  sin((1/2).*(1+(-1).*t).*theta)+q13.*sin((1/2).*t.*theta)).^2)).^2).^( ...
  -3/2).*(4.*(csc((1/2).*theta).^2.*(q01.*sin((1/2).*(1+(-1).*t).*theta)+ ...
  q11.*sin((1/2).*t.*theta)).*(q03.*sin((1/2).*(1+(-1).*t).*theta)+q13.* ...
  sin((1/2).*t.*theta))+csc((1/2).*theta).^2.*(q02.*sin((1/2).*(1+(-1).*t) ...
  .*theta)+q12.*sin((1/2).*t.*theta)).*(q04.*sin((1/2).*(1+(-1).*t).* ...
  theta)+q14.*sin((1/2).*t.*theta))).^2+4.*((-1).*csc((1/2).*theta).^2.*( ...
  q01.*sin((1/2).*(1+(-1).*t).*theta)+q11.*sin((1/2).*t.*theta)).*(q02.* ...
  sin((1/2).*(1+(-1).*t).*theta)+q12.*sin((1/2).*t.*theta))+csc((1/2).* ...
  theta).^2.*(q03.*sin((1/2).*(1+(-1).*t).*theta)+q13.*sin((1/2).*t.* ...
  theta)).*(q04.*sin((1/2).*(1+(-1).*t).*theta)+q14.*sin((1/2).*t.*theta)) ...
  ).^2+(1+(-2).*(csc((1/2).*theta).^2.*(q02.*sin((1/2).*(1+(-1).*t).* ...
  theta)+q12.*sin((1/2).*t.*theta)).^2+csc((1/2).*theta).^2.*(q03.*sin(( ...
  1/2).*(1+(-1).*t).*theta)+q13.*sin((1/2).*t.*theta)).^2)).^2).^(1/2)+( ...
  -2).*((-1).*((-1/2).*q04.*theta.*cos((1/2).*(1+(-1).*t).*theta)+(1/2).* ...
  q14.*theta.*cos((1/2).*t.*theta)).*csc((1/2).*theta).^2.*(q01.*sin((1/2) ...
  .*(1+(-1).*t).*theta)+q11.*sin((1/2).*t.*theta))+((-1/2).*q03.*theta.* ...
  cos((1/2).*(1+(-1).*t).*theta)+(1/2).*q13.*theta.*cos((1/2).*t.*theta)) ...
  .*csc((1/2).*theta).^2.*(q02.*sin((1/2).*(1+(-1).*t).*theta)+q12.*sin(( ...
  1/2).*t.*theta))+((-1/2).*q02.*theta.*cos((1/2).*(1+(-1).*t).*theta)+( ...
  1/2).*q12.*theta.*cos((1/2).*t.*theta)).*csc((1/2).*theta).^2.*(q03.* ...
  sin((1/2).*(1+(-1).*t).*theta)+q13.*sin((1/2).*t.*theta))+(-1).*((-1/2) ...
  .*q01.*theta.*cos((1/2).*(1+(-1).*t).*theta)+(1/2).*q11.*theta.*cos(( ...
  1/2).*t.*theta)).*csc((1/2).*theta).^2.*(q04.*sin((1/2).*(1+(-1).*t).* ...
  theta)+q14.*sin((1/2).*t.*theta))).*(4.*((-1).*csc((1/2).*theta).^2.*( ...
  q01.*sin((1/2).*(1+(-1).*t).*theta)+q11.*sin((1/2).*t.*theta)).*(q02.* ...
  sin((1/2).*(1+(-1).*t).*theta)+q12.*sin((1/2).*t.*theta))+csc((1/2).* ...
  theta).^2.*(q03.*sin((1/2).*(1+(-1).*t).*theta)+q13.*sin((1/2).*t.* ...
  theta)).*(q04.*sin((1/2).*(1+(-1).*t).*theta)+q14.*sin((1/2).*t.*theta)) ...
  ).^2+(1+(-2).*(csc((1/2).*theta).^2.*(q02.*sin((1/2).*(1+(-1).*t).* ...
  theta)+q12.*sin((1/2).*t.*theta)).^2+csc((1/2).*theta).^2.*(q03.*sin(( ...
  1/2).*(1+(-1).*t).*theta)+q13.*sin((1/2).*t.*theta)).^2)).^2).^(-1/2).*( ...
  4.*(csc((1/2).*theta).^2.*(q01.*sin((1/2).*(1+(-1).*t).*theta)+q11.*sin( ...
  (1/2).*t.*theta)).*(q03.*sin((1/2).*(1+(-1).*t).*theta)+q13.*sin((1/2).* ...
  t.*theta))+csc((1/2).*theta).^2.*(q02.*sin((1/2).*(1+(-1).*t).*theta)+ ...
  q12.*sin((1/2).*t.*theta)).*(q04.*sin((1/2).*(1+(-1).*t).*theta)+q14.* ...
  sin((1/2).*t.*theta))).^2+4.*((-1).*csc((1/2).*theta).^2.*(q01.*sin(( ...
  1/2).*(1+(-1).*t).*theta)+q11.*sin((1/2).*t.*theta)).*(q02.*sin((1/2).*( ...
  1+(-1).*t).*theta)+q12.*sin((1/2).*t.*theta))+csc((1/2).*theta).^2.*( ...
  q03.*sin((1/2).*(1+(-1).*t).*theta)+q13.*sin((1/2).*t.*theta)).*(q04.* ...
  sin((1/2).*(1+(-1).*t).*theta)+q14.*sin((1/2).*t.*theta))).^2+(1+(-2).*( ...
  csc((1/2).*theta).^2.*(q02.*sin((1/2).*(1+(-1).*t).*theta)+q12.*sin(( ...
  1/2).*t.*theta)).^2+csc((1/2).*theta).^2.*(q03.*sin((1/2).*(1+(-1).*t).* ...
  theta)+q13.*sin((1/2).*t.*theta)).^2)).^2).^(1/2)).*(4.*(csc((1/2).* ...
  theta).^2.*(q02.*sin((1/2).*(1+(-1).*t).*theta)+q12.*sin((1/2).*t.* ...
  theta)).*(q03.*sin((1/2).*(1+(-1).*t).*theta)+q13.*sin((1/2).*t.*theta)) ...
  +(-1).*csc((1/2).*theta).^2.*(q01.*sin((1/2).*(1+(-1).*t).*theta)+q11.* ...
  sin((1/2).*t.*theta)).*(q04.*sin((1/2).*(1+(-1).*t).*theta)+q14.*sin(( ...
  1/2).*t.*theta))).^2.*(4.*((-1).*csc((1/2).*theta).^2.*(q01.*sin((1/2).* ...
  (1+(-1).*t).*theta)+q11.*sin((1/2).*t.*theta)).*(q02.*sin((1/2).*(1+(-1) ...
  .*t).*theta)+q12.*sin((1/2).*t.*theta))+csc((1/2).*theta).^2.*(q03.*sin( ...
  (1/2).*(1+(-1).*t).*theta)+q13.*sin((1/2).*t.*theta)).*(q04.*sin((1/2).* ...
  (1+(-1).*t).*theta)+q14.*sin((1/2).*t.*theta))).^2+(1+(-2).*(csc((1/2).* ...
  theta).^2.*(q02.*sin((1/2).*(1+(-1).*t).*theta)+q12.*sin((1/2).*t.* ...
  theta)).^2+csc((1/2).*theta).^2.*(q03.*sin((1/2).*(1+(-1).*t).*theta)+ ...
  q13.*sin((1/2).*t.*theta)).^2)).^2).^(-1).*(4.*(csc((1/2).*theta).^2.*( ...
  q01.*sin((1/2).*(1+(-1).*t).*theta)+q11.*sin((1/2).*t.*theta)).*(q03.* ...
  sin((1/2).*(1+(-1).*t).*theta)+q13.*sin((1/2).*t.*theta))+csc((1/2).* ...
  theta).^2.*(q02.*sin((1/2).*(1+(-1).*t).*theta)+q12.*sin((1/2).*t.* ...
  theta)).*(q04.*sin((1/2).*(1+(-1).*t).*theta)+q14.*sin((1/2).*t.*theta)) ...
  ).^2+4.*((-1).*csc((1/2).*theta).^2.*(q01.*sin((1/2).*(1+(-1).*t).* ...
  theta)+q11.*sin((1/2).*t.*theta)).*(q02.*sin((1/2).*(1+(-1).*t).*theta)+ ...
  q12.*sin((1/2).*t.*theta))+csc((1/2).*theta).^2.*(q03.*sin((1/2).*(1+( ...
  -1).*t).*theta)+q13.*sin((1/2).*t.*theta)).*(q04.*sin((1/2).*(1+(-1).*t) ...
  .*theta)+q14.*sin((1/2).*t.*theta))).^2+(1+(-2).*(csc((1/2).*theta).^2.* ...
  (q02.*sin((1/2).*(1+(-1).*t).*theta)+q12.*sin((1/2).*t.*theta)).^2+csc(( ...
  1/2).*theta).^2.*(q03.*sin((1/2).*(1+(-1).*t).*theta)+q13.*sin((1/2).* ...
  t.*theta)).^2)).^2)+(1+(-2).*(csc((1/2).*theta).^2.*(q03.*sin((1/2).*(1+ ...
  (-1).*t).*theta)+q13.*sin((1/2).*t.*theta)).^2+csc((1/2).*theta).^2.*( ...
  q04.*sin((1/2).*(1+(-1).*t).*theta)+q14.*sin((1/2).*t.*theta)).^2)).^2.* ...
  (4.*((-1).*csc((1/2).*theta).^2.*(q01.*sin((1/2).*(1+(-1).*t).*theta)+ ...
  q11.*sin((1/2).*t.*theta)).*(q02.*sin((1/2).*(1+(-1).*t).*theta)+q12.* ...
  sin((1/2).*t.*theta))+csc((1/2).*theta).^2.*(q03.*sin((1/2).*(1+(-1).*t) ...
  .*theta)+q13.*sin((1/2).*t.*theta)).*(q04.*sin((1/2).*(1+(-1).*t).* ...
  theta)+q14.*sin((1/2).*t.*theta))).^2+(1+(-2).*(csc((1/2).*theta).^2.*( ...
  q02.*sin((1/2).*(1+(-1).*t).*theta)+q12.*sin((1/2).*t.*theta)).^2+csc(( ...
  1/2).*theta).^2.*(q03.*sin((1/2).*(1+(-1).*t).*theta)+q13.*sin((1/2).* ...
  t.*theta)).^2)).^2).^(-1).*(4.*(csc((1/2).*theta).^2.*(q01.*sin((1/2).*( ...
  1+(-1).*t).*theta)+q11.*sin((1/2).*t.*theta)).*(q03.*sin((1/2).*(1+(-1) ...
  .*t).*theta)+q13.*sin((1/2).*t.*theta))+csc((1/2).*theta).^2.*(q02.*sin( ...
  (1/2).*(1+(-1).*t).*theta)+q12.*sin((1/2).*t.*theta)).*(q04.*sin((1/2).* ...
  (1+(-1).*t).*theta)+q14.*sin((1/2).*t.*theta))).^2+4.*((-1).*csc((1/2).* ...
  theta).^2.*(q01.*sin((1/2).*(1+(-1).*t).*theta)+q11.*sin((1/2).*t.* ...
  theta)).*(q02.*sin((1/2).*(1+(-1).*t).*theta)+q12.*sin((1/2).*t.*theta)) ...
  +csc((1/2).*theta).^2.*(q03.*sin((1/2).*(1+(-1).*t).*theta)+q13.*sin(( ...
  1/2).*t.*theta)).*(q04.*sin((1/2).*(1+(-1).*t).*theta)+q14.*sin((1/2).* ...
  t.*theta))).^2+(1+(-2).*(csc((1/2).*theta).^2.*(q02.*sin((1/2).*(1+(-1) ...
  .*t).*theta)+q12.*sin((1/2).*t.*theta)).^2+csc((1/2).*theta).^2.*(q03.* ...
  sin((1/2).*(1+(-1).*t).*theta)+q13.*sin((1/2).*t.*theta)).^2)).^2)).^( ...
  -1)+(-2).*(2.*((-1/2).*q03.*theta.*cos((1/2).*(1+(-1).*t).*theta)+(1/2) ...
  .*q13.*theta.*cos((1/2).*t.*theta)).*csc((1/2).*theta).^2.*(q03.*sin(( ...
  1/2).*(1+(-1).*t).*theta)+q13.*sin((1/2).*t.*theta))+2.*((-1/2).*q04.* ...
  theta.*cos((1/2).*(1+(-1).*t).*theta)+(1/2).*q14.*theta.*cos((1/2).*t.* ...
  theta)).*csc((1/2).*theta).^2.*(q04.*sin((1/2).*(1+(-1).*t).*theta)+ ...
  q14.*sin((1/2).*t.*theta))).*(4.*((-1).*csc((1/2).*theta).^2.*(q01.*sin( ...
  (1/2).*(1+(-1).*t).*theta)+q11.*sin((1/2).*t.*theta)).*(q02.*sin((1/2).* ...
  (1+(-1).*t).*theta)+q12.*sin((1/2).*t.*theta))+csc((1/2).*theta).^2.*( ...
  q03.*sin((1/2).*(1+(-1).*t).*theta)+q13.*sin((1/2).*t.*theta)).*(q04.* ...
  sin((1/2).*(1+(-1).*t).*theta)+q14.*sin((1/2).*t.*theta))).^2+(1+(-2).*( ...
  csc((1/2).*theta).^2.*(q02.*sin((1/2).*(1+(-1).*t).*theta)+q12.*sin(( ...
  1/2).*t.*theta)).^2+csc((1/2).*theta).^2.*(q03.*sin((1/2).*(1+(-1).*t).* ...
  theta)+q13.*sin((1/2).*t.*theta)).^2)).^2).^(-1/2).*(4.*(csc((1/2).* ...
  theta).^2.*(q01.*sin((1/2).*(1+(-1).*t).*theta)+q11.*sin((1/2).*t.* ...
  theta)).*(q03.*sin((1/2).*(1+(-1).*t).*theta)+q13.*sin((1/2).*t.*theta)) ...
  +csc((1/2).*theta).^2.*(q02.*sin((1/2).*(1+(-1).*t).*theta)+q12.*sin(( ...
  1/2).*t.*theta)).*(q04.*sin((1/2).*(1+(-1).*t).*theta)+q14.*sin((1/2).* ...
  t.*theta))).^2+4.*((-1).*csc((1/2).*theta).^2.*(q01.*sin((1/2).*(1+(-1) ...
  .*t).*theta)+q11.*sin((1/2).*t.*theta)).*(q02.*sin((1/2).*(1+(-1).*t).* ...
  theta)+q12.*sin((1/2).*t.*theta))+csc((1/2).*theta).^2.*(q03.*sin((1/2) ...
  .*(1+(-1).*t).*theta)+q13.*sin((1/2).*t.*theta)).*(q04.*sin((1/2).*(1+( ...
  -1).*t).*theta)+q14.*sin((1/2).*t.*theta))).^2+(1+(-2).*(csc((1/2).* ...
  theta).^2.*(q02.*sin((1/2).*(1+(-1).*t).*theta)+q12.*sin((1/2).*t.* ...
  theta)).^2+csc((1/2).*theta).^2.*(q03.*sin((1/2).*(1+(-1).*t).*theta)+ ...
  q13.*sin((1/2).*t.*theta)).^2)).^2).^(1/2).*((-1).*(csc((1/2).*theta) ...
  .^2.*(q02.*sin((1/2).*(1+(-1).*t).*theta)+q12.*sin((1/2).*t.*theta)).*( ...
  q03.*sin((1/2).*(1+(-1).*t).*theta)+q13.*sin((1/2).*t.*theta))+(-1).* ...
  csc((1/2).*theta).^2.*(q01.*sin((1/2).*(1+(-1).*t).*theta)+q11.*sin(( ...
  1/2).*t.*theta)).*(q04.*sin((1/2).*(1+(-1).*t).*theta)+q14.*sin((1/2).* ...
  t.*theta))).*(8.*(((-1/2).*q03.*theta.*cos((1/2).*(1+(-1).*t).*theta)+( ...
  1/2).*q13.*theta.*cos((1/2).*t.*theta)).*csc((1/2).*theta).^2.*(q01.* ...
  sin((1/2).*(1+(-1).*t).*theta)+q11.*sin((1/2).*t.*theta))+((-1/2).*q04.* ...
  theta.*cos((1/2).*(1+(-1).*t).*theta)+(1/2).*q14.*theta.*cos((1/2).*t.* ...
  theta)).*csc((1/2).*theta).^2.*(q02.*sin((1/2).*(1+(-1).*t).*theta)+ ...
  q12.*sin((1/2).*t.*theta))+((-1/2).*q01.*theta.*cos((1/2).*(1+(-1).*t).* ...
  theta)+(1/2).*q11.*theta.*cos((1/2).*t.*theta)).*csc((1/2).*theta).^2.*( ...
  q03.*sin((1/2).*(1+(-1).*t).*theta)+q13.*sin((1/2).*t.*theta))+((-1/2).* ...
  q02.*theta.*cos((1/2).*(1+(-1).*t).*theta)+(1/2).*q12.*theta.*cos((1/2) ...
  .*t.*theta)).*csc((1/2).*theta).^2.*(q04.*sin((1/2).*(1+(-1).*t).*theta) ...
  +q14.*sin((1/2).*t.*theta))).*(csc((1/2).*theta).^2.*(q01.*sin((1/2).*( ...
  1+(-1).*t).*theta)+q11.*sin((1/2).*t.*theta)).*(q03.*sin((1/2).*(1+(-1) ...
  .*t).*theta)+q13.*sin((1/2).*t.*theta))+csc((1/2).*theta).^2.*(q02.*sin( ...
  (1/2).*(1+(-1).*t).*theta)+q12.*sin((1/2).*t.*theta)).*(q04.*sin((1/2).* ...
  (1+(-1).*t).*theta)+q14.*sin((1/2).*t.*theta)))+8.*((-1).*((-1/2).*q02.* ...
  theta.*cos((1/2).*(1+(-1).*t).*theta)+(1/2).*q12.*theta.*cos((1/2).*t.* ...
  theta)).*csc((1/2).*theta).^2.*(q01.*sin((1/2).*(1+(-1).*t).*theta)+ ...
  q11.*sin((1/2).*t.*theta))+(-1).*((-1/2).*q01.*theta.*cos((1/2).*(1+(-1) ...
  .*t).*theta)+(1/2).*q11.*theta.*cos((1/2).*t.*theta)).*csc((1/2).*theta) ...
  .^2.*(q02.*sin((1/2).*(1+(-1).*t).*theta)+q12.*sin((1/2).*t.*theta))+(( ...
  -1/2).*q04.*theta.*cos((1/2).*(1+(-1).*t).*theta)+(1/2).*q14.*theta.* ...
  cos((1/2).*t.*theta)).*csc((1/2).*theta).^2.*(q03.*sin((1/2).*(1+(-1).* ...
  t).*theta)+q13.*sin((1/2).*t.*theta))+((-1/2).*q03.*theta.*cos((1/2).*( ...
  1+(-1).*t).*theta)+(1/2).*q13.*theta.*cos((1/2).*t.*theta)).*csc((1/2).* ...
  theta).^2.*(q04.*sin((1/2).*(1+(-1).*t).*theta)+q14.*sin((1/2).*t.* ...
  theta))).*((-1).*csc((1/2).*theta).^2.*(q01.*sin((1/2).*(1+(-1).*t).* ...
  theta)+q11.*sin((1/2).*t.*theta)).*(q02.*sin((1/2).*(1+(-1).*t).*theta)+ ...
  q12.*sin((1/2).*t.*theta))+csc((1/2).*theta).^2.*(q03.*sin((1/2).*(1+( ...
  -1).*t).*theta)+q13.*sin((1/2).*t.*theta)).*(q04.*sin((1/2).*(1+(-1).*t) ...
  .*theta)+q14.*sin((1/2).*t.*theta)))+(-4).*(2.*((-1/2).*q02.*theta.*cos( ...
  (1/2).*(1+(-1).*t).*theta)+(1/2).*q12.*theta.*cos((1/2).*t.*theta)).* ...
  csc((1/2).*theta).^2.*(q02.*sin((1/2).*(1+(-1).*t).*theta)+q12.*sin(( ...
  1/2).*t.*theta))+2.*((-1/2).*q03.*theta.*cos((1/2).*(1+(-1).*t).*theta)+ ...
  (1/2).*q13.*theta.*cos((1/2).*t.*theta)).*csc((1/2).*theta).^2.*(q03.* ...
  sin((1/2).*(1+(-1).*t).*theta)+q13.*sin((1/2).*t.*theta))).*(1+(-2).*( ...
  csc((1/2).*theta).^2.*(q02.*sin((1/2).*(1+(-1).*t).*theta)+q12.*sin(( ...
  1/2).*t.*theta)).^2+csc((1/2).*theta).^2.*(q03.*sin((1/2).*(1+(-1).*t).* ...
  theta)+q13.*sin((1/2).*t.*theta)).^2))).*(4.*((-1).*csc((1/2).*theta) ...
  .^2.*(q01.*sin((1/2).*(1+(-1).*t).*theta)+q11.*sin((1/2).*t.*theta)).*( ...
  q02.*sin((1/2).*(1+(-1).*t).*theta)+q12.*sin((1/2).*t.*theta))+csc((1/2) ...
  .*theta).^2.*(q03.*sin((1/2).*(1+(-1).*t).*theta)+q13.*sin((1/2).*t.* ...
  theta)).*(q04.*sin((1/2).*(1+(-1).*t).*theta)+q14.*sin((1/2).*t.*theta)) ...
  ).^2+(1+(-2).*(csc((1/2).*theta).^2.*(q02.*sin((1/2).*(1+(-1).*t).* ...
  theta)+q12.*sin((1/2).*t.*theta)).^2+csc((1/2).*theta).^2.*(q03.*sin(( ...
  1/2).*(1+(-1).*t).*theta)+q13.*sin((1/2).*t.*theta)).^2)).^2).^(-1/2).*( ...
  4.*(csc((1/2).*theta).^2.*(q01.*sin((1/2).*(1+(-1).*t).*theta)+q11.*sin( ...
  (1/2).*t.*theta)).*(q03.*sin((1/2).*(1+(-1).*t).*theta)+q13.*sin((1/2).* ...
  t.*theta))+csc((1/2).*theta).^2.*(q02.*sin((1/2).*(1+(-1).*t).*theta)+ ...
  q12.*sin((1/2).*t.*theta)).*(q04.*sin((1/2).*(1+(-1).*t).*theta)+q14.* ...
  sin((1/2).*t.*theta))).^2+4.*((-1).*csc((1/2).*theta).^2.*(q01.*sin(( ...
  1/2).*(1+(-1).*t).*theta)+q11.*sin((1/2).*t.*theta)).*(q02.*sin((1/2).*( ...
  1+(-1).*t).*theta)+q12.*sin((1/2).*t.*theta))+csc((1/2).*theta).^2.*( ...
  q03.*sin((1/2).*(1+(-1).*t).*theta)+q13.*sin((1/2).*t.*theta)).*(q04.* ...
  sin((1/2).*(1+(-1).*t).*theta)+q14.*sin((1/2).*t.*theta))).^2+(1+(-2).*( ...
  csc((1/2).*theta).^2.*(q02.*sin((1/2).*(1+(-1).*t).*theta)+q12.*sin(( ...
  1/2).*t.*theta)).^2+csc((1/2).*theta).^2.*(q03.*sin((1/2).*(1+(-1).*t).* ...
  theta)+q13.*sin((1/2).*t.*theta)).^2)).^2).^(-1/2)+(csc((1/2).*theta) ...
  .^2.*(q02.*sin((1/2).*(1+(-1).*t).*theta)+q12.*sin((1/2).*t.*theta)).*( ...
  q03.*sin((1/2).*(1+(-1).*t).*theta)+q13.*sin((1/2).*t.*theta))+(-1).* ...
  csc((1/2).*theta).^2.*(q01.*sin((1/2).*(1+(-1).*t).*theta)+q11.*sin(( ...
  1/2).*t.*theta)).*(q04.*sin((1/2).*(1+(-1).*t).*theta)+q14.*sin((1/2).* ...
  t.*theta))).*(8.*((-1).*((-1/2).*q02.*theta.*cos((1/2).*(1+(-1).*t).* ...
  theta)+(1/2).*q12.*theta.*cos((1/2).*t.*theta)).*csc((1/2).*theta).^2.*( ...
  q01.*sin((1/2).*(1+(-1).*t).*theta)+q11.*sin((1/2).*t.*theta))+(-1).*(( ...
  -1/2).*q01.*theta.*cos((1/2).*(1+(-1).*t).*theta)+(1/2).*q11.*theta.* ...
  cos((1/2).*t.*theta)).*csc((1/2).*theta).^2.*(q02.*sin((1/2).*(1+(-1).* ...
  t).*theta)+q12.*sin((1/2).*t.*theta))+((-1/2).*q04.*theta.*cos((1/2).*( ...
  1+(-1).*t).*theta)+(1/2).*q14.*theta.*cos((1/2).*t.*theta)).*csc((1/2).* ...
  theta).^2.*(q03.*sin((1/2).*(1+(-1).*t).*theta)+q13.*sin((1/2).*t.* ...
  theta))+((-1/2).*q03.*theta.*cos((1/2).*(1+(-1).*t).*theta)+(1/2).*q13.* ...
  theta.*cos((1/2).*t.*theta)).*csc((1/2).*theta).^2.*(q04.*sin((1/2).*(1+ ...
  (-1).*t).*theta)+q14.*sin((1/2).*t.*theta))).*((-1).*csc((1/2).*theta) ...
  .^2.*(q01.*sin((1/2).*(1+(-1).*t).*theta)+q11.*sin((1/2).*t.*theta)).*( ...
  q02.*sin((1/2).*(1+(-1).*t).*theta)+q12.*sin((1/2).*t.*theta))+csc((1/2) ...
  .*theta).^2.*(q03.*sin((1/2).*(1+(-1).*t).*theta)+q13.*sin((1/2).*t.* ...
  theta)).*(q04.*sin((1/2).*(1+(-1).*t).*theta)+q14.*sin((1/2).*t.*theta)) ...
  )+(-4).*(2.*((-1/2).*q02.*theta.*cos((1/2).*(1+(-1).*t).*theta)+(1/2).* ...
  q12.*theta.*cos((1/2).*t.*theta)).*csc((1/2).*theta).^2.*(q02.*sin((1/2) ...
  .*(1+(-1).*t).*theta)+q12.*sin((1/2).*t.*theta))+2.*((-1/2).*q03.* ...
  theta.*cos((1/2).*(1+(-1).*t).*theta)+(1/2).*q13.*theta.*cos((1/2).*t.* ...
  theta)).*csc((1/2).*theta).^2.*(q03.*sin((1/2).*(1+(-1).*t).*theta)+ ...
  q13.*sin((1/2).*t.*theta))).*(1+(-2).*(csc((1/2).*theta).^2.*(q02.*sin(( ...
  1/2).*(1+(-1).*t).*theta)+q12.*sin((1/2).*t.*theta)).^2+csc((1/2).* ...
  theta).^2.*(q03.*sin((1/2).*(1+(-1).*t).*theta)+q13.*sin((1/2).*t.* ...
  theta)).^2))).*(4.*((-1).*csc((1/2).*theta).^2.*(q01.*sin((1/2).*(1+(-1) ...
  .*t).*theta)+q11.*sin((1/2).*t.*theta)).*(q02.*sin((1/2).*(1+(-1).*t).* ...
  theta)+q12.*sin((1/2).*t.*theta))+csc((1/2).*theta).^2.*(q03.*sin((1/2) ...
  .*(1+(-1).*t).*theta)+q13.*sin((1/2).*t.*theta)).*(q04.*sin((1/2).*(1+( ...
  -1).*t).*theta)+q14.*sin((1/2).*t.*theta))).^2+(1+(-2).*(csc((1/2).* ...
  theta).^2.*(q02.*sin((1/2).*(1+(-1).*t).*theta)+q12.*sin((1/2).*t.* ...
  theta)).^2+csc((1/2).*theta).^2.*(q03.*sin((1/2).*(1+(-1).*t).*theta)+ ...
  q13.*sin((1/2).*t.*theta)).^2)).^2).^(-3/2).*(4.*(csc((1/2).*theta).^2.* ...
  (q01.*sin((1/2).*(1+(-1).*t).*theta)+q11.*sin((1/2).*t.*theta)).*(q03.* ...
  sin((1/2).*(1+(-1).*t).*theta)+q13.*sin((1/2).*t.*theta))+csc((1/2).* ...
  theta).^2.*(q02.*sin((1/2).*(1+(-1).*t).*theta)+q12.*sin((1/2).*t.* ...
  theta)).*(q04.*sin((1/2).*(1+(-1).*t).*theta)+q14.*sin((1/2).*t.*theta)) ...
  ).^2+4.*((-1).*csc((1/2).*theta).^2.*(q01.*sin((1/2).*(1+(-1).*t).* ...
  theta)+q11.*sin((1/2).*t.*theta)).*(q02.*sin((1/2).*(1+(-1).*t).*theta)+ ...
  q12.*sin((1/2).*t.*theta))+csc((1/2).*theta).^2.*(q03.*sin((1/2).*(1+( ...
  -1).*t).*theta)+q13.*sin((1/2).*t.*theta)).*(q04.*sin((1/2).*(1+(-1).*t) ...
  .*theta)+q14.*sin((1/2).*t.*theta))).^2+(1+(-2).*(csc((1/2).*theta).^2.* ...
  (q02.*sin((1/2).*(1+(-1).*t).*theta)+q12.*sin((1/2).*t.*theta)).^2+csc(( ...
  1/2).*theta).^2.*(q03.*sin((1/2).*(1+(-1).*t).*theta)+q13.*sin((1/2).* ...
  t.*theta)).^2)).^2).^(1/2)+(-2).*((-1).*((-1/2).*q04.*theta.*cos((1/2).* ...
  (1+(-1).*t).*theta)+(1/2).*q14.*theta.*cos((1/2).*t.*theta)).*csc((1/2) ...
  .*theta).^2.*(q01.*sin((1/2).*(1+(-1).*t).*theta)+q11.*sin((1/2).*t.* ...
  theta))+((-1/2).*q03.*theta.*cos((1/2).*(1+(-1).*t).*theta)+(1/2).*q13.* ...
  theta.*cos((1/2).*t.*theta)).*csc((1/2).*theta).^2.*(q02.*sin((1/2).*(1+ ...
  (-1).*t).*theta)+q12.*sin((1/2).*t.*theta))+((-1/2).*q02.*theta.*cos(( ...
  1/2).*(1+(-1).*t).*theta)+(1/2).*q12.*theta.*cos((1/2).*t.*theta)).*csc( ...
  (1/2).*theta).^2.*(q03.*sin((1/2).*(1+(-1).*t).*theta)+q13.*sin((1/2).* ...
  t.*theta))+(-1).*((-1/2).*q01.*theta.*cos((1/2).*(1+(-1).*t).*theta)+( ...
  1/2).*q11.*theta.*cos((1/2).*t.*theta)).*csc((1/2).*theta).^2.*(q04.* ...
  sin((1/2).*(1+(-1).*t).*theta)+q14.*sin((1/2).*t.*theta))).*(4.*((-1).* ...
  csc((1/2).*theta).^2.*(q01.*sin((1/2).*(1+(-1).*t).*theta)+q11.*sin(( ...
  1/2).*t.*theta)).*(q02.*sin((1/2).*(1+(-1).*t).*theta)+q12.*sin((1/2).* ...
  t.*theta))+csc((1/2).*theta).^2.*(q03.*sin((1/2).*(1+(-1).*t).*theta)+ ...
  q13.*sin((1/2).*t.*theta)).*(q04.*sin((1/2).*(1+(-1).*t).*theta)+q14.* ...
  sin((1/2).*t.*theta))).^2+(1+(-2).*(csc((1/2).*theta).^2.*(q02.*sin(( ...
  1/2).*(1+(-1).*t).*theta)+q12.*sin((1/2).*t.*theta)).^2+csc((1/2).* ...
  theta).^2.*(q03.*sin((1/2).*(1+(-1).*t).*theta)+q13.*sin((1/2).*t.* ...
  theta)).^2)).^2).^(-1/2).*(4.*(csc((1/2).*theta).^2.*(q01.*sin((1/2).*( ...
  1+(-1).*t).*theta)+q11.*sin((1/2).*t.*theta)).*(q03.*sin((1/2).*(1+(-1) ...
  .*t).*theta)+q13.*sin((1/2).*t.*theta))+csc((1/2).*theta).^2.*(q02.*sin( ...
  (1/2).*(1+(-1).*t).*theta)+q12.*sin((1/2).*t.*theta)).*(q04.*sin((1/2).* ...
  (1+(-1).*t).*theta)+q14.*sin((1/2).*t.*theta))).^2+4.*((-1).*csc((1/2).* ...
  theta).^2.*(q01.*sin((1/2).*(1+(-1).*t).*theta)+q11.*sin((1/2).*t.* ...
  theta)).*(q02.*sin((1/2).*(1+(-1).*t).*theta)+q12.*sin((1/2).*t.*theta)) ...
  +csc((1/2).*theta).^2.*(q03.*sin((1/2).*(1+(-1).*t).*theta)+q13.*sin(( ...
  1/2).*t.*theta)).*(q04.*sin((1/2).*(1+(-1).*t).*theta)+q14.*sin((1/2).* ...
  t.*theta))).^2+(1+(-2).*(csc((1/2).*theta).^2.*(q02.*sin((1/2).*(1+(-1) ...
  .*t).*theta)+q12.*sin((1/2).*t.*theta)).^2+csc((1/2).*theta).^2.*(q03.* ...
  sin((1/2).*(1+(-1).*t).*theta)+q13.*sin((1/2).*t.*theta)).^2)).^2).^( ...
  1/2)).*(4.*(csc((1/2).*theta).^2.*(q02.*sin((1/2).*(1+(-1).*t).*theta)+ ...
  q12.*sin((1/2).*t.*theta)).*(q03.*sin((1/2).*(1+(-1).*t).*theta)+q13.* ...
  sin((1/2).*t.*theta))+(-1).*csc((1/2).*theta).^2.*(q01.*sin((1/2).*(1+( ...
  -1).*t).*theta)+q11.*sin((1/2).*t.*theta)).*(q04.*sin((1/2).*(1+(-1).*t) ...
  .*theta)+q14.*sin((1/2).*t.*theta))).^2.*(4.*((-1).*csc((1/2).*theta) ...
  .^2.*(q01.*sin((1/2).*(1+(-1).*t).*theta)+q11.*sin((1/2).*t.*theta)).*( ...
  q02.*sin((1/2).*(1+(-1).*t).*theta)+q12.*sin((1/2).*t.*theta))+csc((1/2) ...
  .*theta).^2.*(q03.*sin((1/2).*(1+(-1).*t).*theta)+q13.*sin((1/2).*t.* ...
  theta)).*(q04.*sin((1/2).*(1+(-1).*t).*theta)+q14.*sin((1/2).*t.*theta)) ...
  ).^2+(1+(-2).*(csc((1/2).*theta).^2.*(q02.*sin((1/2).*(1+(-1).*t).* ...
  theta)+q12.*sin((1/2).*t.*theta)).^2+csc((1/2).*theta).^2.*(q03.*sin(( ...
  1/2).*(1+(-1).*t).*theta)+q13.*sin((1/2).*t.*theta)).^2)).^2).^(-1).*( ...
  4.*(csc((1/2).*theta).^2.*(q01.*sin((1/2).*(1+(-1).*t).*theta)+q11.*sin( ...
  (1/2).*t.*theta)).*(q03.*sin((1/2).*(1+(-1).*t).*theta)+q13.*sin((1/2).* ...
  t.*theta))+csc((1/2).*theta).^2.*(q02.*sin((1/2).*(1+(-1).*t).*theta)+ ...
  q12.*sin((1/2).*t.*theta)).*(q04.*sin((1/2).*(1+(-1).*t).*theta)+q14.* ...
  sin((1/2).*t.*theta))).^2+4.*((-1).*csc((1/2).*theta).^2.*(q01.*sin(( ...
  1/2).*(1+(-1).*t).*theta)+q11.*sin((1/2).*t.*theta)).*(q02.*sin((1/2).*( ...
  1+(-1).*t).*theta)+q12.*sin((1/2).*t.*theta))+csc((1/2).*theta).^2.*( ...
  q03.*sin((1/2).*(1+(-1).*t).*theta)+q13.*sin((1/2).*t.*theta)).*(q04.* ...
  sin((1/2).*(1+(-1).*t).*theta)+q14.*sin((1/2).*t.*theta))).^2+(1+(-2).*( ...
  csc((1/2).*theta).^2.*(q02.*sin((1/2).*(1+(-1).*t).*theta)+q12.*sin(( ...
  1/2).*t.*theta)).^2+csc((1/2).*theta).^2.*(q03.*sin((1/2).*(1+(-1).*t).* ...
  theta)+q13.*sin((1/2).*t.*theta)).^2)).^2)+(1+(-2).*(csc((1/2).*theta) ...
  .^2.*(q03.*sin((1/2).*(1+(-1).*t).*theta)+q13.*sin((1/2).*t.*theta)).^2+ ...
  csc((1/2).*theta).^2.*(q04.*sin((1/2).*(1+(-1).*t).*theta)+q14.*sin(( ...
  1/2).*t.*theta)).^2)).^2.*(4.*((-1).*csc((1/2).*theta).^2.*(q01.*sin(( ...
  1/2).*(1+(-1).*t).*theta)+q11.*sin((1/2).*t.*theta)).*(q02.*sin((1/2).*( ...
  1+(-1).*t).*theta)+q12.*sin((1/2).*t.*theta))+csc((1/2).*theta).^2.*( ...
  q03.*sin((1/2).*(1+(-1).*t).*theta)+q13.*sin((1/2).*t.*theta)).*(q04.* ...
  sin((1/2).*(1+(-1).*t).*theta)+q14.*sin((1/2).*t.*theta))).^2+(1+(-2).*( ...
  csc((1/2).*theta).^2.*(q02.*sin((1/2).*(1+(-1).*t).*theta)+q12.*sin(( ...
  1/2).*t.*theta)).^2+csc((1/2).*theta).^2.*(q03.*sin((1/2).*(1+(-1).*t).* ...
  theta)+q13.*sin((1/2).*t.*theta)).^2)).^2).^(-1).*(4.*(csc((1/2).*theta) ...
  .^2.*(q01.*sin((1/2).*(1+(-1).*t).*theta)+q11.*sin((1/2).*t.*theta)).*( ...
  q03.*sin((1/2).*(1+(-1).*t).*theta)+q13.*sin((1/2).*t.*theta))+csc((1/2) ...
  .*theta).^2.*(q02.*sin((1/2).*(1+(-1).*t).*theta)+q12.*sin((1/2).*t.* ...
  theta)).*(q04.*sin((1/2).*(1+(-1).*t).*theta)+q14.*sin((1/2).*t.*theta)) ...
  ).^2+4.*((-1).*csc((1/2).*theta).^2.*(q01.*sin((1/2).*(1+(-1).*t).* ...
  theta)+q11.*sin((1/2).*t.*theta)).*(q02.*sin((1/2).*(1+(-1).*t).*theta)+ ...
  q12.*sin((1/2).*t.*theta))+csc((1/2).*theta).^2.*(q03.*sin((1/2).*(1+( ...
  -1).*t).*theta)+q13.*sin((1/2).*t.*theta)).*(q04.*sin((1/2).*(1+(-1).*t) ...
  .*theta)+q14.*sin((1/2).*t.*theta))).^2+(1+(-2).*(csc((1/2).*theta).^2.* ...
  (q02.*sin((1/2).*(1+(-1).*t).*theta)+q12.*sin((1/2).*t.*theta)).^2+csc(( ...
  1/2).*theta).^2.*(q03.*sin((1/2).*(1+(-1).*t).*theta)+q13.*sin((1/2).* ...
  t.*theta)).^2)).^2)).^(-1)+(csc((1/2).*theta).^2.*(q02.*sin((1/2).*(1+( ...
  -1).*t).*theta)+q12.*sin((1/2).*t.*theta)).*(q03.*sin((1/2).*(1+(-1).*t) ...
  .*theta)+q13.*sin((1/2).*t.*theta))+(-1).*csc((1/2).*theta).^2.*(q01.* ...
  sin((1/2).*(1+(-1).*t).*theta)+q11.*sin((1/2).*t.*theta)).*(q04.*sin(( ...
  1/2).*(1+(-1).*t).*theta)+q14.*sin((1/2).*t.*theta))).*(8.*(((-1/2).* ...
  q03.*theta.*cos((1/2).*(1+(-1).*t).*theta)+(1/2).*q13.*theta.*cos((1/2) ...
  .*t.*theta)).*csc((1/2).*theta).^2.*(q01.*sin((1/2).*(1+(-1).*t).*theta) ...
  +q11.*sin((1/2).*t.*theta))+((-1/2).*q04.*theta.*cos((1/2).*(1+(-1).*t) ...
  .*theta)+(1/2).*q14.*theta.*cos((1/2).*t.*theta)).*csc((1/2).*theta) ...
  .^2.*(q02.*sin((1/2).*(1+(-1).*t).*theta)+q12.*sin((1/2).*t.*theta))+(( ...
  -1/2).*q01.*theta.*cos((1/2).*(1+(-1).*t).*theta)+(1/2).*q11.*theta.* ...
  cos((1/2).*t.*theta)).*csc((1/2).*theta).^2.*(q03.*sin((1/2).*(1+(-1).* ...
  t).*theta)+q13.*sin((1/2).*t.*theta))+((-1/2).*q02.*theta.*cos((1/2).*( ...
  1+(-1).*t).*theta)+(1/2).*q12.*theta.*cos((1/2).*t.*theta)).*csc((1/2).* ...
  theta).^2.*(q04.*sin((1/2).*(1+(-1).*t).*theta)+q14.*sin((1/2).*t.* ...
  theta))).*(csc((1/2).*theta).^2.*(q01.*sin((1/2).*(1+(-1).*t).*theta)+ ...
  q11.*sin((1/2).*t.*theta)).*(q03.*sin((1/2).*(1+(-1).*t).*theta)+q13.* ...
  sin((1/2).*t.*theta))+csc((1/2).*theta).^2.*(q02.*sin((1/2).*(1+(-1).*t) ...
  .*theta)+q12.*sin((1/2).*t.*theta)).*(q04.*sin((1/2).*(1+(-1).*t).* ...
  theta)+q14.*sin((1/2).*t.*theta)))+8.*((-1).*((-1/2).*q02.*theta.*cos(( ...
  1/2).*(1+(-1).*t).*theta)+(1/2).*q12.*theta.*cos((1/2).*t.*theta)).*csc( ...
  (1/2).*theta).^2.*(q01.*sin((1/2).*(1+(-1).*t).*theta)+q11.*sin((1/2).* ...
  t.*theta))+(-1).*((-1/2).*q01.*theta.*cos((1/2).*(1+(-1).*t).*theta)+( ...
  1/2).*q11.*theta.*cos((1/2).*t.*theta)).*csc((1/2).*theta).^2.*(q02.* ...
  sin((1/2).*(1+(-1).*t).*theta)+q12.*sin((1/2).*t.*theta))+((-1/2).*q04.* ...
  theta.*cos((1/2).*(1+(-1).*t).*theta)+(1/2).*q14.*theta.*cos((1/2).*t.* ...
  theta)).*csc((1/2).*theta).^2.*(q03.*sin((1/2).*(1+(-1).*t).*theta)+ ...
  q13.*sin((1/2).*t.*theta))+((-1/2).*q03.*theta.*cos((1/2).*(1+(-1).*t).* ...
  theta)+(1/2).*q13.*theta.*cos((1/2).*t.*theta)).*csc((1/2).*theta).^2.*( ...
  q04.*sin((1/2).*(1+(-1).*t).*theta)+q14.*sin((1/2).*t.*theta))).*((-1).* ...
  csc((1/2).*theta).^2.*(q01.*sin((1/2).*(1+(-1).*t).*theta)+q11.*sin(( ...
  1/2).*t.*theta)).*(q02.*sin((1/2).*(1+(-1).*t).*theta)+q12.*sin((1/2).* ...
  t.*theta))+csc((1/2).*theta).^2.*(q03.*sin((1/2).*(1+(-1).*t).*theta)+ ...
  q13.*sin((1/2).*t.*theta)).*(q04.*sin((1/2).*(1+(-1).*t).*theta)+q14.* ...
  sin((1/2).*t.*theta)))+(-4).*(2.*((-1/2).*q02.*theta.*cos((1/2).*(1+(-1) ...
  .*t).*theta)+(1/2).*q12.*theta.*cos((1/2).*t.*theta)).*csc((1/2).*theta) ...
  .^2.*(q02.*sin((1/2).*(1+(-1).*t).*theta)+q12.*sin((1/2).*t.*theta))+2.* ...
  ((-1/2).*q03.*theta.*cos((1/2).*(1+(-1).*t).*theta)+(1/2).*q13.*theta.* ...
  cos((1/2).*t.*theta)).*csc((1/2).*theta).^2.*(q03.*sin((1/2).*(1+(-1).* ...
  t).*theta)+q13.*sin((1/2).*t.*theta))).*(1+(-2).*(csc((1/2).*theta).^2.* ...
  (q02.*sin((1/2).*(1+(-1).*t).*theta)+q12.*sin((1/2).*t.*theta)).^2+csc(( ...
  1/2).*theta).^2.*(q03.*sin((1/2).*(1+(-1).*t).*theta)+q13.*sin((1/2).* ...
  t.*theta)).^2))).*(4.*((-1).*csc((1/2).*theta).^2.*(q01.*sin((1/2).*(1+( ...
  -1).*t).*theta)+q11.*sin((1/2).*t.*theta)).*(q02.*sin((1/2).*(1+(-1).*t) ...
  .*theta)+q12.*sin((1/2).*t.*theta))+csc((1/2).*theta).^2.*(q03.*sin(( ...
  1/2).*(1+(-1).*t).*theta)+q13.*sin((1/2).*t.*theta)).*(q04.*sin((1/2).*( ...
  1+(-1).*t).*theta)+q14.*sin((1/2).*t.*theta))).^2+(1+(-2).*(csc((1/2).* ...
  theta).^2.*(q02.*sin((1/2).*(1+(-1).*t).*theta)+q12.*sin((1/2).*t.* ...
  theta)).^2+csc((1/2).*theta).^2.*(q03.*sin((1/2).*(1+(-1).*t).*theta)+ ...
  q13.*sin((1/2).*t.*theta)).^2)).^2).^(-1/2).*(4.*(csc((1/2).*theta).^2.* ...
  (q01.*sin((1/2).*(1+(-1).*t).*theta)+q11.*sin((1/2).*t.*theta)).*(q03.* ...
  sin((1/2).*(1+(-1).*t).*theta)+q13.*sin((1/2).*t.*theta))+csc((1/2).* ...
  theta).^2.*(q02.*sin((1/2).*(1+(-1).*t).*theta)+q12.*sin((1/2).*t.* ...
  theta)).*(q04.*sin((1/2).*(1+(-1).*t).*theta)+q14.*sin((1/2).*t.*theta)) ...
  ).^2+4.*((-1).*csc((1/2).*theta).^2.*(q01.*sin((1/2).*(1+(-1).*t).* ...
  theta)+q11.*sin((1/2).*t.*theta)).*(q02.*sin((1/2).*(1+(-1).*t).*theta)+ ...
  q12.*sin((1/2).*t.*theta))+csc((1/2).*theta).^2.*(q03.*sin((1/2).*(1+( ...
  -1).*t).*theta)+q13.*sin((1/2).*t.*theta)).*(q04.*sin((1/2).*(1+(-1).*t) ...
  .*theta)+q14.*sin((1/2).*t.*theta))).^2+(1+(-2).*(csc((1/2).*theta).^2.* ...
  (q02.*sin((1/2).*(1+(-1).*t).*theta)+q12.*sin((1/2).*t.*theta)).^2+csc(( ...
  1/2).*theta).^2.*(q03.*sin((1/2).*(1+(-1).*t).*theta)+q13.*sin((1/2).* ...
  t.*theta)).^2)).^2).^(-1/2).*((1/2).*(1+(-2).*(csc((1/2).*theta).^2.*( ...
  q03.*sin((1/2).*(1+(-1).*t).*theta)+q13.*sin((1/2).*t.*theta)).^2+csc(( ...
  1/2).*theta).^2.*(q04.*sin((1/2).*(1+(-1).*t).*theta)+q14.*sin((1/2).* ...
  t.*theta)).^2)).*(8.*(((-1/2).*q03.*theta.*cos((1/2).*(1+(-1).*t).* ...
  theta)+(1/2).*q13.*theta.*cos((1/2).*t.*theta)).*csc((1/2).*theta).^2.*( ...
  q01.*sin((1/2).*(1+(-1).*t).*theta)+q11.*sin((1/2).*t.*theta))+((-1/2).* ...
  q04.*theta.*cos((1/2).*(1+(-1).*t).*theta)+(1/2).*q14.*theta.*cos((1/2) ...
  .*t.*theta)).*csc((1/2).*theta).^2.*(q02.*sin((1/2).*(1+(-1).*t).*theta) ...
  +q12.*sin((1/2).*t.*theta))+((-1/2).*q01.*theta.*cos((1/2).*(1+(-1).*t) ...
  .*theta)+(1/2).*q11.*theta.*cos((1/2).*t.*theta)).*csc((1/2).*theta) ...
  .^2.*(q03.*sin((1/2).*(1+(-1).*t).*theta)+q13.*sin((1/2).*t.*theta))+(( ...
  -1/2).*q02.*theta.*cos((1/2).*(1+(-1).*t).*theta)+(1/2).*q12.*theta.* ...
  cos((1/2).*t.*theta)).*csc((1/2).*theta).^2.*(q04.*sin((1/2).*(1+(-1).* ...
  t).*theta)+q14.*sin((1/2).*t.*theta))).*(csc((1/2).*theta).^2.*(q01.* ...
  sin((1/2).*(1+(-1).*t).*theta)+q11.*sin((1/2).*t.*theta)).*(q03.*sin(( ...
  1/2).*(1+(-1).*t).*theta)+q13.*sin((1/2).*t.*theta))+csc((1/2).*theta) ...
  .^2.*(q02.*sin((1/2).*(1+(-1).*t).*theta)+q12.*sin((1/2).*t.*theta)).*( ...
  q04.*sin((1/2).*(1+(-1).*t).*theta)+q14.*sin((1/2).*t.*theta)))+8.*((-1) ...
  .*((-1/2).*q02.*theta.*cos((1/2).*(1+(-1).*t).*theta)+(1/2).*q12.* ...
  theta.*cos((1/2).*t.*theta)).*csc((1/2).*theta).^2.*(q01.*sin((1/2).*(1+ ...
  (-1).*t).*theta)+q11.*sin((1/2).*t.*theta))+(-1).*((-1/2).*q01.*theta.* ...
  cos((1/2).*(1+(-1).*t).*theta)+(1/2).*q11.*theta.*cos((1/2).*t.*theta)) ...
  .*csc((1/2).*theta).^2.*(q02.*sin((1/2).*(1+(-1).*t).*theta)+q12.*sin(( ...
  1/2).*t.*theta))+((-1/2).*q04.*theta.*cos((1/2).*(1+(-1).*t).*theta)+( ...
  1/2).*q14.*theta.*cos((1/2).*t.*theta)).*csc((1/2).*theta).^2.*(q03.* ...
  sin((1/2).*(1+(-1).*t).*theta)+q13.*sin((1/2).*t.*theta))+((-1/2).*q03.* ...
  theta.*cos((1/2).*(1+(-1).*t).*theta)+(1/2).*q13.*theta.*cos((1/2).*t.* ...
  theta)).*csc((1/2).*theta).^2.*(q04.*sin((1/2).*(1+(-1).*t).*theta)+ ...
  q14.*sin((1/2).*t.*theta))).*((-1).*csc((1/2).*theta).^2.*(q01.*sin(( ...
  1/2).*(1+(-1).*t).*theta)+q11.*sin((1/2).*t.*theta)).*(q02.*sin((1/2).*( ...
  1+(-1).*t).*theta)+q12.*sin((1/2).*t.*theta))+csc((1/2).*theta).^2.*( ...
  q03.*sin((1/2).*(1+(-1).*t).*theta)+q13.*sin((1/2).*t.*theta)).*(q04.* ...
  sin((1/2).*(1+(-1).*t).*theta)+q14.*sin((1/2).*t.*theta)))+(-4).*(2.*(( ...
  -1/2).*q02.*theta.*cos((1/2).*(1+(-1).*t).*theta)+(1/2).*q12.*theta.* ...
  cos((1/2).*t.*theta)).*csc((1/2).*theta).^2.*(q02.*sin((1/2).*(1+(-1).* ...
  t).*theta)+q12.*sin((1/2).*t.*theta))+2.*((-1/2).*q03.*theta.*cos((1/2) ...
  .*(1+(-1).*t).*theta)+(1/2).*q13.*theta.*cos((1/2).*t.*theta)).*csc(( ...
  1/2).*theta).^2.*(q03.*sin((1/2).*(1+(-1).*t).*theta)+q13.*sin((1/2).* ...
  t.*theta))).*(1+(-2).*(csc((1/2).*theta).^2.*(q02.*sin((1/2).*(1+(-1).* ...
  t).*theta)+q12.*sin((1/2).*t.*theta)).^2+csc((1/2).*theta).^2.*(q03.* ...
  sin((1/2).*(1+(-1).*t).*theta)+q13.*sin((1/2).*t.*theta)).^2))).*(4.*(( ...
  -1).*csc((1/2).*theta).^2.*(q01.*sin((1/2).*(1+(-1).*t).*theta)+q11.* ...
  sin((1/2).*t.*theta)).*(q02.*sin((1/2).*(1+(-1).*t).*theta)+q12.*sin(( ...
  1/2).*t.*theta))+csc((1/2).*theta).^2.*(q03.*sin((1/2).*(1+(-1).*t).* ...
  theta)+q13.*sin((1/2).*t.*theta)).*(q04.*sin((1/2).*(1+(-1).*t).*theta)+ ...
  q14.*sin((1/2).*t.*theta))).^2+(1+(-2).*(csc((1/2).*theta).^2.*(q02.* ...
  sin((1/2).*(1+(-1).*t).*theta)+q12.*sin((1/2).*t.*theta)).^2+csc((1/2).* ...
  theta).^2.*(q03.*sin((1/2).*(1+(-1).*t).*theta)+q13.*sin((1/2).*t.* ...
  theta)).^2)).^2).^(-1/2).*(4.*(csc((1/2).*theta).^2.*(q01.*sin((1/2).*( ...
  1+(-1).*t).*theta)+q11.*sin((1/2).*t.*theta)).*(q03.*sin((1/2).*(1+(-1) ...
  .*t).*theta)+q13.*sin((1/2).*t.*theta))+csc((1/2).*theta).^2.*(q02.*sin( ...
  (1/2).*(1+(-1).*t).*theta)+q12.*sin((1/2).*t.*theta)).*(q04.*sin((1/2).* ...
  (1+(-1).*t).*theta)+q14.*sin((1/2).*t.*theta))).^2+4.*((-1).*csc((1/2).* ...
  theta).^2.*(q01.*sin((1/2).*(1+(-1).*t).*theta)+q11.*sin((1/2).*t.* ...
  theta)).*(q02.*sin((1/2).*(1+(-1).*t).*theta)+q12.*sin((1/2).*t.*theta)) ...
  +csc((1/2).*theta).^2.*(q03.*sin((1/2).*(1+(-1).*t).*theta)+q13.*sin(( ...
  1/2).*t.*theta)).*(q04.*sin((1/2).*(1+(-1).*t).*theta)+q14.*sin((1/2).* ...
  t.*theta))).^2+(1+(-2).*(csc((1/2).*theta).^2.*(q02.*sin((1/2).*(1+(-1) ...
  .*t).*theta)+q12.*sin((1/2).*t.*theta)).^2+csc((1/2).*theta).^2.*(q03.* ...
  sin((1/2).*(1+(-1).*t).*theta)+q13.*sin((1/2).*t.*theta)).^2)).^2).^( ...
  -1/2)+(-1/2).*(1+(-2).*(csc((1/2).*theta).^2.*(q03.*sin((1/2).*(1+(-1).* ...
  t).*theta)+q13.*sin((1/2).*t.*theta)).^2+csc((1/2).*theta).^2.*(q04.* ...
  sin((1/2).*(1+(-1).*t).*theta)+q14.*sin((1/2).*t.*theta)).^2)).*(8.*(( ...
  -1).*((-1/2).*q02.*theta.*cos((1/2).*(1+(-1).*t).*theta)+(1/2).*q12.* ...
  theta.*cos((1/2).*t.*theta)).*csc((1/2).*theta).^2.*(q01.*sin((1/2).*(1+ ...
  (-1).*t).*theta)+q11.*sin((1/2).*t.*theta))+(-1).*((-1/2).*q01.*theta.* ...
  cos((1/2).*(1+(-1).*t).*theta)+(1/2).*q11.*theta.*cos((1/2).*t.*theta)) ...
  .*csc((1/2).*theta).^2.*(q02.*sin((1/2).*(1+(-1).*t).*theta)+q12.*sin(( ...
  1/2).*t.*theta))+((-1/2).*q04.*theta.*cos((1/2).*(1+(-1).*t).*theta)+( ...
  1/2).*q14.*theta.*cos((1/2).*t.*theta)).*csc((1/2).*theta).^2.*(q03.* ...
  sin((1/2).*(1+(-1).*t).*theta)+q13.*sin((1/2).*t.*theta))+((-1/2).*q03.* ...
  theta.*cos((1/2).*(1+(-1).*t).*theta)+(1/2).*q13.*theta.*cos((1/2).*t.* ...
  theta)).*csc((1/2).*theta).^2.*(q04.*sin((1/2).*(1+(-1).*t).*theta)+ ...
  q14.*sin((1/2).*t.*theta))).*((-1).*csc((1/2).*theta).^2.*(q01.*sin(( ...
  1/2).*(1+(-1).*t).*theta)+q11.*sin((1/2).*t.*theta)).*(q02.*sin((1/2).*( ...
  1+(-1).*t).*theta)+q12.*sin((1/2).*t.*theta))+csc((1/2).*theta).^2.*( ...
  q03.*sin((1/2).*(1+(-1).*t).*theta)+q13.*sin((1/2).*t.*theta)).*(q04.* ...
  sin((1/2).*(1+(-1).*t).*theta)+q14.*sin((1/2).*t.*theta)))+(-4).*(2.*(( ...
  -1/2).*q02.*theta.*cos((1/2).*(1+(-1).*t).*theta)+(1/2).*q12.*theta.* ...
  cos((1/2).*t.*theta)).*csc((1/2).*theta).^2.*(q02.*sin((1/2).*(1+(-1).* ...
  t).*theta)+q12.*sin((1/2).*t.*theta))+2.*((-1/2).*q03.*theta.*cos((1/2) ...
  .*(1+(-1).*t).*theta)+(1/2).*q13.*theta.*cos((1/2).*t.*theta)).*csc(( ...
  1/2).*theta).^2.*(q03.*sin((1/2).*(1+(-1).*t).*theta)+q13.*sin((1/2).* ...
  t.*theta))).*(1+(-2).*(csc((1/2).*theta).^2.*(q02.*sin((1/2).*(1+(-1).* ...
  t).*theta)+q12.*sin((1/2).*t.*theta)).^2+csc((1/2).*theta).^2.*(q03.* ...
  sin((1/2).*(1+(-1).*t).*theta)+q13.*sin((1/2).*t.*theta)).^2))).*(4.*(( ...
  -1).*csc((1/2).*theta).^2.*(q01.*sin((1/2).*(1+(-1).*t).*theta)+q11.* ...
  sin((1/2).*t.*theta)).*(q02.*sin((1/2).*(1+(-1).*t).*theta)+q12.*sin(( ...
  1/2).*t.*theta))+csc((1/2).*theta).^2.*(q03.*sin((1/2).*(1+(-1).*t).* ...
  theta)+q13.*sin((1/2).*t.*theta)).*(q04.*sin((1/2).*(1+(-1).*t).*theta)+ ...
  q14.*sin((1/2).*t.*theta))).^2+(1+(-2).*(csc((1/2).*theta).^2.*(q02.* ...
  sin((1/2).*(1+(-1).*t).*theta)+q12.*sin((1/2).*t.*theta)).^2+csc((1/2).* ...
  theta).^2.*(q03.*sin((1/2).*(1+(-1).*t).*theta)+q13.*sin((1/2).*t.* ...
  theta)).^2)).^2).^(-3/2).*(4.*(csc((1/2).*theta).^2.*(q01.*sin((1/2).*( ...
  1+(-1).*t).*theta)+q11.*sin((1/2).*t.*theta)).*(q03.*sin((1/2).*(1+(-1) ...
  .*t).*theta)+q13.*sin((1/2).*t.*theta))+csc((1/2).*theta).^2.*(q02.*sin( ...
  (1/2).*(1+(-1).*t).*theta)+q12.*sin((1/2).*t.*theta)).*(q04.*sin((1/2).* ...
  (1+(-1).*t).*theta)+q14.*sin((1/2).*t.*theta))).^2+4.*((-1).*csc((1/2).* ...
  theta).^2.*(q01.*sin((1/2).*(1+(-1).*t).*theta)+q11.*sin((1/2).*t.* ...
  theta)).*(q02.*sin((1/2).*(1+(-1).*t).*theta)+q12.*sin((1/2).*t.*theta)) ...
  +csc((1/2).*theta).^2.*(q03.*sin((1/2).*(1+(-1).*t).*theta)+q13.*sin(( ...
  1/2).*t.*theta)).*(q04.*sin((1/2).*(1+(-1).*t).*theta)+q14.*sin((1/2).* ...
  t.*theta))).^2+(1+(-2).*(csc((1/2).*theta).^2.*(q02.*sin((1/2).*(1+(-1) ...
  .*t).*theta)+q12.*sin((1/2).*t.*theta)).^2+csc((1/2).*theta).^2.*(q03.* ...
  sin((1/2).*(1+(-1).*t).*theta)+q13.*sin((1/2).*t.*theta)).^2)).^2).^( ...
  1/2)+(-2).*(2.*((-1/2).*q03.*theta.*cos((1/2).*(1+(-1).*t).*theta)+(1/2) ...
  .*q13.*theta.*cos((1/2).*t.*theta)).*csc((1/2).*theta).^2.*(q03.*sin(( ...
  1/2).*(1+(-1).*t).*theta)+q13.*sin((1/2).*t.*theta))+2.*((-1/2).*q04.* ...
  theta.*cos((1/2).*(1+(-1).*t).*theta)+(1/2).*q14.*theta.*cos((1/2).*t.* ...
  theta)).*csc((1/2).*theta).^2.*(q04.*sin((1/2).*(1+(-1).*t).*theta)+ ...
  q14.*sin((1/2).*t.*theta))).*(4.*((-1).*csc((1/2).*theta).^2.*(q01.*sin( ...
  (1/2).*(1+(-1).*t).*theta)+q11.*sin((1/2).*t.*theta)).*(q02.*sin((1/2).* ...
  (1+(-1).*t).*theta)+q12.*sin((1/2).*t.*theta))+csc((1/2).*theta).^2.*( ...
  q03.*sin((1/2).*(1+(-1).*t).*theta)+q13.*sin((1/2).*t.*theta)).*(q04.* ...
  sin((1/2).*(1+(-1).*t).*theta)+q14.*sin((1/2).*t.*theta))).^2+(1+(-2).*( ...
  csc((1/2).*theta).^2.*(q02.*sin((1/2).*(1+(-1).*t).*theta)+q12.*sin(( ...
  1/2).*t.*theta)).^2+csc((1/2).*theta).^2.*(q03.*sin((1/2).*(1+(-1).*t).* ...
  theta)+q13.*sin((1/2).*t.*theta)).^2)).^2).^(-1/2).*(4.*(csc((1/2).* ...
  theta).^2.*(q01.*sin((1/2).*(1+(-1).*t).*theta)+q11.*sin((1/2).*t.* ...
  theta)).*(q03.*sin((1/2).*(1+(-1).*t).*theta)+q13.*sin((1/2).*t.*theta)) ...
  +csc((1/2).*theta).^2.*(q02.*sin((1/2).*(1+(-1).*t).*theta)+q12.*sin(( ...
  1/2).*t.*theta)).*(q04.*sin((1/2).*(1+(-1).*t).*theta)+q14.*sin((1/2).* ...
  t.*theta))).^2+4.*((-1).*csc((1/2).*theta).^2.*(q01.*sin((1/2).*(1+(-1) ...
  .*t).*theta)+q11.*sin((1/2).*t.*theta)).*(q02.*sin((1/2).*(1+(-1).*t).* ...
  theta)+q12.*sin((1/2).*t.*theta))+csc((1/2).*theta).^2.*(q03.*sin((1/2) ...
  .*(1+(-1).*t).*theta)+q13.*sin((1/2).*t.*theta)).*(q04.*sin((1/2).*(1+( ...
  -1).*t).*theta)+q14.*sin((1/2).*t.*theta))).^2+(1+(-2).*(csc((1/2).* ...
  theta).^2.*(q02.*sin((1/2).*(1+(-1).*t).*theta)+q12.*sin((1/2).*t.* ...
  theta)).^2+csc((1/2).*theta).^2.*(q03.*sin((1/2).*(1+(-1).*t).*theta)+ ...
  q13.*sin((1/2).*t.*theta)).^2)).^2).^(1/2)).*(4.*(csc((1/2).*theta).^2.* ...
  (q02.*sin((1/2).*(1+(-1).*t).*theta)+q12.*sin((1/2).*t.*theta)).*(q03.* ...
  sin((1/2).*(1+(-1).*t).*theta)+q13.*sin((1/2).*t.*theta))+(-1).*csc(( ...
  1/2).*theta).^2.*(q01.*sin((1/2).*(1+(-1).*t).*theta)+q11.*sin((1/2).* ...
  t.*theta)).*(q04.*sin((1/2).*(1+(-1).*t).*theta)+q14.*sin((1/2).*t.* ...
  theta))).^2.*(4.*((-1).*csc((1/2).*theta).^2.*(q01.*sin((1/2).*(1+(-1).* ...
  t).*theta)+q11.*sin((1/2).*t.*theta)).*(q02.*sin((1/2).*(1+(-1).*t).* ...
  theta)+q12.*sin((1/2).*t.*theta))+csc((1/2).*theta).^2.*(q03.*sin((1/2) ...
  .*(1+(-1).*t).*theta)+q13.*sin((1/2).*t.*theta)).*(q04.*sin((1/2).*(1+( ...
  -1).*t).*theta)+q14.*sin((1/2).*t.*theta))).^2+(1+(-2).*(csc((1/2).* ...
  theta).^2.*(q02.*sin((1/2).*(1+(-1).*t).*theta)+q12.*sin((1/2).*t.* ...
  theta)).^2+csc((1/2).*theta).^2.*(q03.*sin((1/2).*(1+(-1).*t).*theta)+ ...
  q13.*sin((1/2).*t.*theta)).^2)).^2).^(-1).*(4.*(csc((1/2).*theta).^2.*( ...
  q01.*sin((1/2).*(1+(-1).*t).*theta)+q11.*sin((1/2).*t.*theta)).*(q03.* ...
  sin((1/2).*(1+(-1).*t).*theta)+q13.*sin((1/2).*t.*theta))+csc((1/2).* ...
  theta).^2.*(q02.*sin((1/2).*(1+(-1).*t).*theta)+q12.*sin((1/2).*t.* ...
  theta)).*(q04.*sin((1/2).*(1+(-1).*t).*theta)+q14.*sin((1/2).*t.*theta)) ...
  ).^2+4.*((-1).*csc((1/2).*theta).^2.*(q01.*sin((1/2).*(1+(-1).*t).* ...
  theta)+q11.*sin((1/2).*t.*theta)).*(q02.*sin((1/2).*(1+(-1).*t).*theta)+ ...
  q12.*sin((1/2).*t.*theta))+csc((1/2).*theta).^2.*(q03.*sin((1/2).*(1+( ...
  -1).*t).*theta)+q13.*sin((1/2).*t.*theta)).*(q04.*sin((1/2).*(1+(-1).*t) ...
  .*theta)+q14.*sin((1/2).*t.*theta))).^2+(1+(-2).*(csc((1/2).*theta).^2.* ...
  (q02.*sin((1/2).*(1+(-1).*t).*theta)+q12.*sin((1/2).*t.*theta)).^2+csc(( ...
  1/2).*theta).^2.*(q03.*sin((1/2).*(1+(-1).*t).*theta)+q13.*sin((1/2).* ...
  t.*theta)).^2)).^2)+(1+(-2).*(csc((1/2).*theta).^2.*(q03.*sin((1/2).*(1+ ...
  (-1).*t).*theta)+q13.*sin((1/2).*t.*theta)).^2+csc((1/2).*theta).^2.*( ...
  q04.*sin((1/2).*(1+(-1).*t).*theta)+q14.*sin((1/2).*t.*theta)).^2)).^2.* ...
  (4.*((-1).*csc((1/2).*theta).^2.*(q01.*sin((1/2).*(1+(-1).*t).*theta)+ ...
  q11.*sin((1/2).*t.*theta)).*(q02.*sin((1/2).*(1+(-1).*t).*theta)+q12.* ...
  sin((1/2).*t.*theta))+csc((1/2).*theta).^2.*(q03.*sin((1/2).*(1+(-1).*t) ...
  .*theta)+q13.*sin((1/2).*t.*theta)).*(q04.*sin((1/2).*(1+(-1).*t).* ...
  theta)+q14.*sin((1/2).*t.*theta))).^2+(1+(-2).*(csc((1/2).*theta).^2.*( ...
  q02.*sin((1/2).*(1+(-1).*t).*theta)+q12.*sin((1/2).*t.*theta)).^2+csc(( ...
  1/2).*theta).^2.*(q03.*sin((1/2).*(1+(-1).*t).*theta)+q13.*sin((1/2).* ...
  t.*theta)).^2)).^2).^(-1).*(4.*(csc((1/2).*theta).^2.*(q01.*sin((1/2).*( ...
  1+(-1).*t).*theta)+q11.*sin((1/2).*t.*theta)).*(q03.*sin((1/2).*(1+(-1) ...
  .*t).*theta)+q13.*sin((1/2).*t.*theta))+csc((1/2).*theta).^2.*(q02.*sin( ...
  (1/2).*(1+(-1).*t).*theta)+q12.*sin((1/2).*t.*theta)).*(q04.*sin((1/2).* ...
  (1+(-1).*t).*theta)+q14.*sin((1/2).*t.*theta))).^2+4.*((-1).*csc((1/2).* ...
  theta).^2.*(q01.*sin((1/2).*(1+(-1).*t).*theta)+q11.*sin((1/2).*t.* ...
  theta)).*(q02.*sin((1/2).*(1+(-1).*t).*theta)+q12.*sin((1/2).*t.*theta)) ...
  +csc((1/2).*theta).^2.*(q03.*sin((1/2).*(1+(-1).*t).*theta)+q13.*sin(( ...
  1/2).*t.*theta)).*(q04.*sin((1/2).*(1+(-1).*t).*theta)+q14.*sin((1/2).* ...
  t.*theta))).^2+(1+(-2).*(csc((1/2).*theta).^2.*(q02.*sin((1/2).*(1+(-1) ...
  .*t).*theta)+q12.*sin((1/2).*t.*theta)).^2+csc((1/2).*theta).^2.*(q03.* ...
  sin((1/2).*(1+(-1).*t).*theta)+q13.*sin((1/2).*t.*theta)).^2)).^2)).^( ...
  -1)+(-1).*(csc((1/2).*theta).^2.*(q02.*sin((1/2).*(1+(-1).*t).*theta)+ ...
  q12.*sin((1/2).*t.*theta)).*(q03.*sin((1/2).*(1+(-1).*t).*theta)+q13.* ...
  sin((1/2).*t.*theta))+(-1).*csc((1/2).*theta).^2.*(q01.*sin((1/2).*(1+( ...
  -1).*t).*theta)+q11.*sin((1/2).*t.*theta)).*(q04.*sin((1/2).*(1+(-1).*t) ...
  .*theta)+q14.*sin((1/2).*t.*theta))).*(8.*((-1).*((-1/2).*q02.*theta.* ...
  cos((1/2).*(1+(-1).*t).*theta)+(1/2).*q12.*theta.*cos((1/2).*t.*theta)) ...
  .*csc((1/2).*theta).^2.*(q01.*sin((1/2).*(1+(-1).*t).*theta)+q11.*sin(( ...
  1/2).*t.*theta))+(-1).*((-1/2).*q01.*theta.*cos((1/2).*(1+(-1).*t).* ...
  theta)+(1/2).*q11.*theta.*cos((1/2).*t.*theta)).*csc((1/2).*theta).^2.*( ...
  q02.*sin((1/2).*(1+(-1).*t).*theta)+q12.*sin((1/2).*t.*theta))+((-1/2).* ...
  q04.*theta.*cos((1/2).*(1+(-1).*t).*theta)+(1/2).*q14.*theta.*cos((1/2) ...
  .*t.*theta)).*csc((1/2).*theta).^2.*(q03.*sin((1/2).*(1+(-1).*t).*theta) ...
  +q13.*sin((1/2).*t.*theta))+((-1/2).*q03.*theta.*cos((1/2).*(1+(-1).*t) ...
  .*theta)+(1/2).*q13.*theta.*cos((1/2).*t.*theta)).*csc((1/2).*theta) ...
  .^2.*(q04.*sin((1/2).*(1+(-1).*t).*theta)+q14.*sin((1/2).*t.*theta))).*( ...
  (-1).*csc((1/2).*theta).^2.*(q01.*sin((1/2).*(1+(-1).*t).*theta)+q11.* ...
  sin((1/2).*t.*theta)).*(q02.*sin((1/2).*(1+(-1).*t).*theta)+q12.*sin(( ...
  1/2).*t.*theta))+csc((1/2).*theta).^2.*(q03.*sin((1/2).*(1+(-1).*t).* ...
  theta)+q13.*sin((1/2).*t.*theta)).*(q04.*sin((1/2).*(1+(-1).*t).*theta)+ ...
  q14.*sin((1/2).*t.*theta)))+(-4).*(2.*((-1/2).*q02.*theta.*cos((1/2).*( ...
  1+(-1).*t).*theta)+(1/2).*q12.*theta.*cos((1/2).*t.*theta)).*csc((1/2).* ...
  theta).^2.*(q02.*sin((1/2).*(1+(-1).*t).*theta)+q12.*sin((1/2).*t.* ...
  theta))+2.*((-1/2).*q03.*theta.*cos((1/2).*(1+(-1).*t).*theta)+(1/2).* ...
  q13.*theta.*cos((1/2).*t.*theta)).*csc((1/2).*theta).^2.*(q03.*sin((1/2) ...
  .*(1+(-1).*t).*theta)+q13.*sin((1/2).*t.*theta))).*(1+(-2).*(csc((1/2).* ...
  theta).^2.*(q02.*sin((1/2).*(1+(-1).*t).*theta)+q12.*sin((1/2).*t.* ...
  theta)).^2+csc((1/2).*theta).^2.*(q03.*sin((1/2).*(1+(-1).*t).*theta)+ ...
  q13.*sin((1/2).*t.*theta)).^2))).*(4.*((-1).*csc((1/2).*theta).^2.*( ...
  q01.*sin((1/2).*(1+(-1).*t).*theta)+q11.*sin((1/2).*t.*theta)).*(q02.* ...
  sin((1/2).*(1+(-1).*t).*theta)+q12.*sin((1/2).*t.*theta))+csc((1/2).* ...
  theta).^2.*(q03.*sin((1/2).*(1+(-1).*t).*theta)+q13.*sin((1/2).*t.* ...
  theta)).*(q04.*sin((1/2).*(1+(-1).*t).*theta)+q14.*sin((1/2).*t.*theta)) ...
  ).^2+(1+(-2).*(csc((1/2).*theta).^2.*(q02.*sin((1/2).*(1+(-1).*t).* ...
  theta)+q12.*sin((1/2).*t.*theta)).^2+csc((1/2).*theta).^2.*(q03.*sin(( ...
  1/2).*(1+(-1).*t).*theta)+q13.*sin((1/2).*t.*theta)).^2)).^2).^(-3/2).*( ...
  4.*(csc((1/2).*theta).^2.*(q01.*sin((1/2).*(1+(-1).*t).*theta)+q11.*sin( ...
  (1/2).*t.*theta)).*(q03.*sin((1/2).*(1+(-1).*t).*theta)+q13.*sin((1/2).* ...
  t.*theta))+csc((1/2).*theta).^2.*(q02.*sin((1/2).*(1+(-1).*t).*theta)+ ...
  q12.*sin((1/2).*t.*theta)).*(q04.*sin((1/2).*(1+(-1).*t).*theta)+q14.* ...
  sin((1/2).*t.*theta))).^2+4.*((-1).*csc((1/2).*theta).^2.*(q01.*sin(( ...
  1/2).*(1+(-1).*t).*theta)+q11.*sin((1/2).*t.*theta)).*(q02.*sin((1/2).*( ...
  1+(-1).*t).*theta)+q12.*sin((1/2).*t.*theta))+csc((1/2).*theta).^2.*( ...
  q03.*sin((1/2).*(1+(-1).*t).*theta)+q13.*sin((1/2).*t.*theta)).*(q04.* ...
  sin((1/2).*(1+(-1).*t).*theta)+q14.*sin((1/2).*t.*theta))).^2+(1+(-2).*( ...
  csc((1/2).*theta).^2.*(q02.*sin((1/2).*(1+(-1).*t).*theta)+q12.*sin(( ...
  1/2).*t.*theta)).^2+csc((1/2).*theta).^2.*(q03.*sin((1/2).*(1+(-1).*t).* ...
  theta)+q13.*sin((1/2).*t.*theta)).^2)).^2).^(1/2).*((1/2).*(1+(-2).*( ...
  csc((1/2).*theta).^2.*(q03.*sin((1/2).*(1+(-1).*t).*theta)+q13.*sin(( ...
  1/2).*t.*theta)).^2+csc((1/2).*theta).^2.*(q04.*sin((1/2).*(1+(-1).*t).* ...
  theta)+q14.*sin((1/2).*t.*theta)).^2)).*(8.*(((-1/2).*q03.*theta.*cos(( ...
  1/2).*(1+(-1).*t).*theta)+(1/2).*q13.*theta.*cos((1/2).*t.*theta)).*csc( ...
  (1/2).*theta).^2.*(q01.*sin((1/2).*(1+(-1).*t).*theta)+q11.*sin((1/2).* ...
  t.*theta))+((-1/2).*q04.*theta.*cos((1/2).*(1+(-1).*t).*theta)+(1/2).* ...
  q14.*theta.*cos((1/2).*t.*theta)).*csc((1/2).*theta).^2.*(q02.*sin((1/2) ...
  .*(1+(-1).*t).*theta)+q12.*sin((1/2).*t.*theta))+((-1/2).*q01.*theta.* ...
  cos((1/2).*(1+(-1).*t).*theta)+(1/2).*q11.*theta.*cos((1/2).*t.*theta)) ...
  .*csc((1/2).*theta).^2.*(q03.*sin((1/2).*(1+(-1).*t).*theta)+q13.*sin(( ...
  1/2).*t.*theta))+((-1/2).*q02.*theta.*cos((1/2).*(1+(-1).*t).*theta)+( ...
  1/2).*q12.*theta.*cos((1/2).*t.*theta)).*csc((1/2).*theta).^2.*(q04.* ...
  sin((1/2).*(1+(-1).*t).*theta)+q14.*sin((1/2).*t.*theta))).*(csc((1/2).* ...
  theta).^2.*(q01.*sin((1/2).*(1+(-1).*t).*theta)+q11.*sin((1/2).*t.* ...
  theta)).*(q03.*sin((1/2).*(1+(-1).*t).*theta)+q13.*sin((1/2).*t.*theta)) ...
  +csc((1/2).*theta).^2.*(q02.*sin((1/2).*(1+(-1).*t).*theta)+q12.*sin(( ...
  1/2).*t.*theta)).*(q04.*sin((1/2).*(1+(-1).*t).*theta)+q14.*sin((1/2).* ...
  t.*theta)))+8.*((-1).*((-1/2).*q02.*theta.*cos((1/2).*(1+(-1).*t).* ...
  theta)+(1/2).*q12.*theta.*cos((1/2).*t.*theta)).*csc((1/2).*theta).^2.*( ...
  q01.*sin((1/2).*(1+(-1).*t).*theta)+q11.*sin((1/2).*t.*theta))+(-1).*(( ...
  -1/2).*q01.*theta.*cos((1/2).*(1+(-1).*t).*theta)+(1/2).*q11.*theta.* ...
  cos((1/2).*t.*theta)).*csc((1/2).*theta).^2.*(q02.*sin((1/2).*(1+(-1).* ...
  t).*theta)+q12.*sin((1/2).*t.*theta))+((-1/2).*q04.*theta.*cos((1/2).*( ...
  1+(-1).*t).*theta)+(1/2).*q14.*theta.*cos((1/2).*t.*theta)).*csc((1/2).* ...
  theta).^2.*(q03.*sin((1/2).*(1+(-1).*t).*theta)+q13.*sin((1/2).*t.* ...
  theta))+((-1/2).*q03.*theta.*cos((1/2).*(1+(-1).*t).*theta)+(1/2).*q13.* ...
  theta.*cos((1/2).*t.*theta)).*csc((1/2).*theta).^2.*(q04.*sin((1/2).*(1+ ...
  (-1).*t).*theta)+q14.*sin((1/2).*t.*theta))).*((-1).*csc((1/2).*theta) ...
  .^2.*(q01.*sin((1/2).*(1+(-1).*t).*theta)+q11.*sin((1/2).*t.*theta)).*( ...
  q02.*sin((1/2).*(1+(-1).*t).*theta)+q12.*sin((1/2).*t.*theta))+csc((1/2) ...
  .*theta).^2.*(q03.*sin((1/2).*(1+(-1).*t).*theta)+q13.*sin((1/2).*t.* ...
  theta)).*(q04.*sin((1/2).*(1+(-1).*t).*theta)+q14.*sin((1/2).*t.*theta)) ...
  )+(-4).*(2.*((-1/2).*q02.*theta.*cos((1/2).*(1+(-1).*t).*theta)+(1/2).* ...
  q12.*theta.*cos((1/2).*t.*theta)).*csc((1/2).*theta).^2.*(q02.*sin((1/2) ...
  .*(1+(-1).*t).*theta)+q12.*sin((1/2).*t.*theta))+2.*((-1/2).*q03.* ...
  theta.*cos((1/2).*(1+(-1).*t).*theta)+(1/2).*q13.*theta.*cos((1/2).*t.* ...
  theta)).*csc((1/2).*theta).^2.*(q03.*sin((1/2).*(1+(-1).*t).*theta)+ ...
  q13.*sin((1/2).*t.*theta))).*(1+(-2).*(csc((1/2).*theta).^2.*(q02.*sin(( ...
  1/2).*(1+(-1).*t).*theta)+q12.*sin((1/2).*t.*theta)).^2+csc((1/2).* ...
  theta).^2.*(q03.*sin((1/2).*(1+(-1).*t).*theta)+q13.*sin((1/2).*t.* ...
  theta)).^2))).*(4.*((-1).*csc((1/2).*theta).^2.*(q01.*sin((1/2).*(1+(-1) ...
  .*t).*theta)+q11.*sin((1/2).*t.*theta)).*(q02.*sin((1/2).*(1+(-1).*t).* ...
  theta)+q12.*sin((1/2).*t.*theta))+csc((1/2).*theta).^2.*(q03.*sin((1/2) ...
  .*(1+(-1).*t).*theta)+q13.*sin((1/2).*t.*theta)).*(q04.*sin((1/2).*(1+( ...
  -1).*t).*theta)+q14.*sin((1/2).*t.*theta))).^2+(1+(-2).*(csc((1/2).* ...
  theta).^2.*(q02.*sin((1/2).*(1+(-1).*t).*theta)+q12.*sin((1/2).*t.* ...
  theta)).^2+csc((1/2).*theta).^2.*(q03.*sin((1/2).*(1+(-1).*t).*theta)+ ...
  q13.*sin((1/2).*t.*theta)).^2)).^2).^(-1/2).*(4.*(csc((1/2).*theta).^2.* ...
  (q01.*sin((1/2).*(1+(-1).*t).*theta)+q11.*sin((1/2).*t.*theta)).*(q03.* ...
  sin((1/2).*(1+(-1).*t).*theta)+q13.*sin((1/2).*t.*theta))+csc((1/2).* ...
  theta).^2.*(q02.*sin((1/2).*(1+(-1).*t).*theta)+q12.*sin((1/2).*t.* ...
  theta)).*(q04.*sin((1/2).*(1+(-1).*t).*theta)+q14.*sin((1/2).*t.*theta)) ...
  ).^2+4.*((-1).*csc((1/2).*theta).^2.*(q01.*sin((1/2).*(1+(-1).*t).* ...
  theta)+q11.*sin((1/2).*t.*theta)).*(q02.*sin((1/2).*(1+(-1).*t).*theta)+ ...
  q12.*sin((1/2).*t.*theta))+csc((1/2).*theta).^2.*(q03.*sin((1/2).*(1+( ...
  -1).*t).*theta)+q13.*sin((1/2).*t.*theta)).*(q04.*sin((1/2).*(1+(-1).*t) ...
  .*theta)+q14.*sin((1/2).*t.*theta))).^2+(1+(-2).*(csc((1/2).*theta).^2.* ...
  (q02.*sin((1/2).*(1+(-1).*t).*theta)+q12.*sin((1/2).*t.*theta)).^2+csc(( ...
  1/2).*theta).^2.*(q03.*sin((1/2).*(1+(-1).*t).*theta)+q13.*sin((1/2).* ...
  t.*theta)).^2)).^2).^(-1/2)+(-1/2).*(1+(-2).*(csc((1/2).*theta).^2.*( ...
  q03.*sin((1/2).*(1+(-1).*t).*theta)+q13.*sin((1/2).*t.*theta)).^2+csc(( ...
  1/2).*theta).^2.*(q04.*sin((1/2).*(1+(-1).*t).*theta)+q14.*sin((1/2).* ...
  t.*theta)).^2)).*(8.*((-1).*((-1/2).*q02.*theta.*cos((1/2).*(1+(-1).*t) ...
  .*theta)+(1/2).*q12.*theta.*cos((1/2).*t.*theta)).*csc((1/2).*theta) ...
  .^2.*(q01.*sin((1/2).*(1+(-1).*t).*theta)+q11.*sin((1/2).*t.*theta))+( ...
  -1).*((-1/2).*q01.*theta.*cos((1/2).*(1+(-1).*t).*theta)+(1/2).*q11.* ...
  theta.*cos((1/2).*t.*theta)).*csc((1/2).*theta).^2.*(q02.*sin((1/2).*(1+ ...
  (-1).*t).*theta)+q12.*sin((1/2).*t.*theta))+((-1/2).*q04.*theta.*cos(( ...
  1/2).*(1+(-1).*t).*theta)+(1/2).*q14.*theta.*cos((1/2).*t.*theta)).*csc( ...
  (1/2).*theta).^2.*(q03.*sin((1/2).*(1+(-1).*t).*theta)+q13.*sin((1/2).* ...
  t.*theta))+((-1/2).*q03.*theta.*cos((1/2).*(1+(-1).*t).*theta)+(1/2).* ...
  q13.*theta.*cos((1/2).*t.*theta)).*csc((1/2).*theta).^2.*(q04.*sin((1/2) ...
  .*(1+(-1).*t).*theta)+q14.*sin((1/2).*t.*theta))).*((-1).*csc((1/2).* ...
  theta).^2.*(q01.*sin((1/2).*(1+(-1).*t).*theta)+q11.*sin((1/2).*t.* ...
  theta)).*(q02.*sin((1/2).*(1+(-1).*t).*theta)+q12.*sin((1/2).*t.*theta)) ...
  +csc((1/2).*theta).^2.*(q03.*sin((1/2).*(1+(-1).*t).*theta)+q13.*sin(( ...
  1/2).*t.*theta)).*(q04.*sin((1/2).*(1+(-1).*t).*theta)+q14.*sin((1/2).* ...
  t.*theta)))+(-4).*(2.*((-1/2).*q02.*theta.*cos((1/2).*(1+(-1).*t).* ...
  theta)+(1/2).*q12.*theta.*cos((1/2).*t.*theta)).*csc((1/2).*theta).^2.*( ...
  q02.*sin((1/2).*(1+(-1).*t).*theta)+q12.*sin((1/2).*t.*theta))+2.*(( ...
  -1/2).*q03.*theta.*cos((1/2).*(1+(-1).*t).*theta)+(1/2).*q13.*theta.* ...
  cos((1/2).*t.*theta)).*csc((1/2).*theta).^2.*(q03.*sin((1/2).*(1+(-1).* ...
  t).*theta)+q13.*sin((1/2).*t.*theta))).*(1+(-2).*(csc((1/2).*theta).^2.* ...
  (q02.*sin((1/2).*(1+(-1).*t).*theta)+q12.*sin((1/2).*t.*theta)).^2+csc(( ...
  1/2).*theta).^2.*(q03.*sin((1/2).*(1+(-1).*t).*theta)+q13.*sin((1/2).* ...
  t.*theta)).^2))).*(4.*((-1).*csc((1/2).*theta).^2.*(q01.*sin((1/2).*(1+( ...
  -1).*t).*theta)+q11.*sin((1/2).*t.*theta)).*(q02.*sin((1/2).*(1+(-1).*t) ...
  .*theta)+q12.*sin((1/2).*t.*theta))+csc((1/2).*theta).^2.*(q03.*sin(( ...
  1/2).*(1+(-1).*t).*theta)+q13.*sin((1/2).*t.*theta)).*(q04.*sin((1/2).*( ...
  1+(-1).*t).*theta)+q14.*sin((1/2).*t.*theta))).^2+(1+(-2).*(csc((1/2).* ...
  theta).^2.*(q02.*sin((1/2).*(1+(-1).*t).*theta)+q12.*sin((1/2).*t.* ...
  theta)).^2+csc((1/2).*theta).^2.*(q03.*sin((1/2).*(1+(-1).*t).*theta)+ ...
  q13.*sin((1/2).*t.*theta)).^2)).^2).^(-3/2).*(4.*(csc((1/2).*theta).^2.* ...
  (q01.*sin((1/2).*(1+(-1).*t).*theta)+q11.*sin((1/2).*t.*theta)).*(q03.* ...
  sin((1/2).*(1+(-1).*t).*theta)+q13.*sin((1/2).*t.*theta))+csc((1/2).* ...
  theta).^2.*(q02.*sin((1/2).*(1+(-1).*t).*theta)+q12.*sin((1/2).*t.* ...
  theta)).*(q04.*sin((1/2).*(1+(-1).*t).*theta)+q14.*sin((1/2).*t.*theta)) ...
  ).^2+4.*((-1).*csc((1/2).*theta).^2.*(q01.*sin((1/2).*(1+(-1).*t).* ...
  theta)+q11.*sin((1/2).*t.*theta)).*(q02.*sin((1/2).*(1+(-1).*t).*theta)+ ...
  q12.*sin((1/2).*t.*theta))+csc((1/2).*theta).^2.*(q03.*sin((1/2).*(1+( ...
  -1).*t).*theta)+q13.*sin((1/2).*t.*theta)).*(q04.*sin((1/2).*(1+(-1).*t) ...
  .*theta)+q14.*sin((1/2).*t.*theta))).^2+(1+(-2).*(csc((1/2).*theta).^2.* ...
  (q02.*sin((1/2).*(1+(-1).*t).*theta)+q12.*sin((1/2).*t.*theta)).^2+csc(( ...
  1/2).*theta).^2.*(q03.*sin((1/2).*(1+(-1).*t).*theta)+q13.*sin((1/2).* ...
  t.*theta)).^2)).^2).^(1/2)+(-2).*(2.*((-1/2).*q03.*theta.*cos((1/2).*(1+ ...
  (-1).*t).*theta)+(1/2).*q13.*theta.*cos((1/2).*t.*theta)).*csc((1/2).* ...
  theta).^2.*(q03.*sin((1/2).*(1+(-1).*t).*theta)+q13.*sin((1/2).*t.* ...
  theta))+2.*((-1/2).*q04.*theta.*cos((1/2).*(1+(-1).*t).*theta)+(1/2).* ...
  q14.*theta.*cos((1/2).*t.*theta)).*csc((1/2).*theta).^2.*(q04.*sin((1/2) ...
  .*(1+(-1).*t).*theta)+q14.*sin((1/2).*t.*theta))).*(4.*((-1).*csc((1/2) ...
  .*theta).^2.*(q01.*sin((1/2).*(1+(-1).*t).*theta)+q11.*sin((1/2).*t.* ...
  theta)).*(q02.*sin((1/2).*(1+(-1).*t).*theta)+q12.*sin((1/2).*t.*theta)) ...
  +csc((1/2).*theta).^2.*(q03.*sin((1/2).*(1+(-1).*t).*theta)+q13.*sin(( ...
  1/2).*t.*theta)).*(q04.*sin((1/2).*(1+(-1).*t).*theta)+q14.*sin((1/2).* ...
  t.*theta))).^2+(1+(-2).*(csc((1/2).*theta).^2.*(q02.*sin((1/2).*(1+(-1) ...
  .*t).*theta)+q12.*sin((1/2).*t.*theta)).^2+csc((1/2).*theta).^2.*(q03.* ...
  sin((1/2).*(1+(-1).*t).*theta)+q13.*sin((1/2).*t.*theta)).^2)).^2).^( ...
  -1/2).*(4.*(csc((1/2).*theta).^2.*(q01.*sin((1/2).*(1+(-1).*t).*theta)+ ...
  q11.*sin((1/2).*t.*theta)).*(q03.*sin((1/2).*(1+(-1).*t).*theta)+q13.* ...
  sin((1/2).*t.*theta))+csc((1/2).*theta).^2.*(q02.*sin((1/2).*(1+(-1).*t) ...
  .*theta)+q12.*sin((1/2).*t.*theta)).*(q04.*sin((1/2).*(1+(-1).*t).* ...
  theta)+q14.*sin((1/2).*t.*theta))).^2+4.*((-1).*csc((1/2).*theta).^2.*( ...
  q01.*sin((1/2).*(1+(-1).*t).*theta)+q11.*sin((1/2).*t.*theta)).*(q02.* ...
  sin((1/2).*(1+(-1).*t).*theta)+q12.*sin((1/2).*t.*theta))+csc((1/2).* ...
  theta).^2.*(q03.*sin((1/2).*(1+(-1).*t).*theta)+q13.*sin((1/2).*t.* ...
  theta)).*(q04.*sin((1/2).*(1+(-1).*t).*theta)+q14.*sin((1/2).*t.*theta)) ...
  ).^2+(1+(-2).*(csc((1/2).*theta).^2.*(q02.*sin((1/2).*(1+(-1).*t).* ...
  theta)+q12.*sin((1/2).*t.*theta)).^2+csc((1/2).*theta).^2.*(q03.*sin(( ...
  1/2).*(1+(-1).*t).*theta)+q13.*sin((1/2).*t.*theta)).^2)).^2).^(1/2)).*( ...
  4.*(csc((1/2).*theta).^2.*(q02.*sin((1/2).*(1+(-1).*t).*theta)+q12.*sin( ...
  (1/2).*t.*theta)).*(q03.*sin((1/2).*(1+(-1).*t).*theta)+q13.*sin((1/2).* ...
  t.*theta))+(-1).*csc((1/2).*theta).^2.*(q01.*sin((1/2).*(1+(-1).*t).* ...
  theta)+q11.*sin((1/2).*t.*theta)).*(q04.*sin((1/2).*(1+(-1).*t).*theta)+ ...
  q14.*sin((1/2).*t.*theta))).^2.*(4.*((-1).*csc((1/2).*theta).^2.*(q01.* ...
  sin((1/2).*(1+(-1).*t).*theta)+q11.*sin((1/2).*t.*theta)).*(q02.*sin(( ...
  1/2).*(1+(-1).*t).*theta)+q12.*sin((1/2).*t.*theta))+csc((1/2).*theta) ...
  .^2.*(q03.*sin((1/2).*(1+(-1).*t).*theta)+q13.*sin((1/2).*t.*theta)).*( ...
  q04.*sin((1/2).*(1+(-1).*t).*theta)+q14.*sin((1/2).*t.*theta))).^2+(1+( ...
  -2).*(csc((1/2).*theta).^2.*(q02.*sin((1/2).*(1+(-1).*t).*theta)+q12.* ...
  sin((1/2).*t.*theta)).^2+csc((1/2).*theta).^2.*(q03.*sin((1/2).*(1+(-1) ...
  .*t).*theta)+q13.*sin((1/2).*t.*theta)).^2)).^2).^(-1).*(4.*(csc((1/2).* ...
  theta).^2.*(q01.*sin((1/2).*(1+(-1).*t).*theta)+q11.*sin((1/2).*t.* ...
  theta)).*(q03.*sin((1/2).*(1+(-1).*t).*theta)+q13.*sin((1/2).*t.*theta)) ...
  +csc((1/2).*theta).^2.*(q02.*sin((1/2).*(1+(-1).*t).*theta)+q12.*sin(( ...
  1/2).*t.*theta)).*(q04.*sin((1/2).*(1+(-1).*t).*theta)+q14.*sin((1/2).* ...
  t.*theta))).^2+4.*((-1).*csc((1/2).*theta).^2.*(q01.*sin((1/2).*(1+(-1) ...
  .*t).*theta)+q11.*sin((1/2).*t.*theta)).*(q02.*sin((1/2).*(1+(-1).*t).* ...
  theta)+q12.*sin((1/2).*t.*theta))+csc((1/2).*theta).^2.*(q03.*sin((1/2) ...
  .*(1+(-1).*t).*theta)+q13.*sin((1/2).*t.*theta)).*(q04.*sin((1/2).*(1+( ...
  -1).*t).*theta)+q14.*sin((1/2).*t.*theta))).^2+(1+(-2).*(csc((1/2).* ...
  theta).^2.*(q02.*sin((1/2).*(1+(-1).*t).*theta)+q12.*sin((1/2).*t.* ...
  theta)).^2+csc((1/2).*theta).^2.*(q03.*sin((1/2).*(1+(-1).*t).*theta)+ ...
  q13.*sin((1/2).*t.*theta)).^2)).^2)+(1+(-2).*(csc((1/2).*theta).^2.*( ...
  q03.*sin((1/2).*(1+(-1).*t).*theta)+q13.*sin((1/2).*t.*theta)).^2+csc(( ...
  1/2).*theta).^2.*(q04.*sin((1/2).*(1+(-1).*t).*theta)+q14.*sin((1/2).* ...
  t.*theta)).^2)).^2.*(4.*((-1).*csc((1/2).*theta).^2.*(q01.*sin((1/2).*( ...
  1+(-1).*t).*theta)+q11.*sin((1/2).*t.*theta)).*(q02.*sin((1/2).*(1+(-1) ...
  .*t).*theta)+q12.*sin((1/2).*t.*theta))+csc((1/2).*theta).^2.*(q03.*sin( ...
  (1/2).*(1+(-1).*t).*theta)+q13.*sin((1/2).*t.*theta)).*(q04.*sin((1/2).* ...
  (1+(-1).*t).*theta)+q14.*sin((1/2).*t.*theta))).^2+(1+(-2).*(csc((1/2).* ...
  theta).^2.*(q02.*sin((1/2).*(1+(-1).*t).*theta)+q12.*sin((1/2).*t.* ...
  theta)).^2+csc((1/2).*theta).^2.*(q03.*sin((1/2).*(1+(-1).*t).*theta)+ ...
  q13.*sin((1/2).*t.*theta)).^2)).^2).^(-1).*(4.*(csc((1/2).*theta).^2.*( ...
  q01.*sin((1/2).*(1+(-1).*t).*theta)+q11.*sin((1/2).*t.*theta)).*(q03.* ...
  sin((1/2).*(1+(-1).*t).*theta)+q13.*sin((1/2).*t.*theta))+csc((1/2).* ...
  theta).^2.*(q02.*sin((1/2).*(1+(-1).*t).*theta)+q12.*sin((1/2).*t.* ...
  theta)).*(q04.*sin((1/2).*(1+(-1).*t).*theta)+q14.*sin((1/2).*t.*theta)) ...
  ).^2+4.*((-1).*csc((1/2).*theta).^2.*(q01.*sin((1/2).*(1+(-1).*t).* ...
  theta)+q11.*sin((1/2).*t.*theta)).*(q02.*sin((1/2).*(1+(-1).*t).*theta)+ ...
  q12.*sin((1/2).*t.*theta))+csc((1/2).*theta).^2.*(q03.*sin((1/2).*(1+( ...
  -1).*t).*theta)+q13.*sin((1/2).*t.*theta)).*(q04.*sin((1/2).*(1+(-1).*t) ...
  .*theta)+q14.*sin((1/2).*t.*theta))).^2+(1+(-2).*(csc((1/2).*theta).^2.* ...
  (q02.*sin((1/2).*(1+(-1).*t).*theta)+q12.*sin((1/2).*t.*theta)).^2+csc(( ...
  1/2).*theta).^2.*(q03.*sin((1/2).*(1+(-1).*t).*theta)+q13.*sin((1/2).* ...
  t.*theta)).^2)).^2)).^(-1)+2.*((-1).*((-1/2).*q04.*theta.*cos((1/2).*(1+ ...
  (-1).*t).*theta)+(1/2).*q14.*theta.*cos((1/2).*t.*theta)).*csc((1/2).* ...
  theta).^2.*(q01.*sin((1/2).*(1+(-1).*t).*theta)+q11.*sin((1/2).*t.* ...
  theta))+((-1/2).*q03.*theta.*cos((1/2).*(1+(-1).*t).*theta)+(1/2).*q13.* ...
  theta.*cos((1/2).*t.*theta)).*csc((1/2).*theta).^2.*(q02.*sin((1/2).*(1+ ...
  (-1).*t).*theta)+q12.*sin((1/2).*t.*theta))+((-1/2).*q02.*theta.*cos(( ...
  1/2).*(1+(-1).*t).*theta)+(1/2).*q12.*theta.*cos((1/2).*t.*theta)).*csc( ...
  (1/2).*theta).^2.*(q03.*sin((1/2).*(1+(-1).*t).*theta)+q13.*sin((1/2).* ...
  t.*theta))+(-1).*((-1/2).*q01.*theta.*cos((1/2).*(1+(-1).*t).*theta)+( ...
  1/2).*q11.*theta.*cos((1/2).*t.*theta)).*csc((1/2).*theta).^2.*(q04.* ...
  sin((1/2).*(1+(-1).*t).*theta)+q14.*sin((1/2).*t.*theta))).*(4.*((-1).* ...
  csc((1/2).*theta).^2.*(q01.*sin((1/2).*(1+(-1).*t).*theta)+q11.*sin(( ...
  1/2).*t.*theta)).*(q02.*sin((1/2).*(1+(-1).*t).*theta)+q12.*sin((1/2).* ...
  t.*theta))+csc((1/2).*theta).^2.*(q03.*sin((1/2).*(1+(-1).*t).*theta)+ ...
  q13.*sin((1/2).*t.*theta)).*(q04.*sin((1/2).*(1+(-1).*t).*theta)+q14.* ...
  sin((1/2).*t.*theta))).^2+(1+(-2).*(csc((1/2).*theta).^2.*(q02.*sin(( ...
  1/2).*(1+(-1).*t).*theta)+q12.*sin((1/2).*t.*theta)).^2+csc((1/2).* ...
  theta).^2.*(q03.*sin((1/2).*(1+(-1).*t).*theta)+q13.*sin((1/2).*t.* ...
  theta)).^2)).^2).^(-1/2).*(4.*(csc((1/2).*theta).^2.*(q01.*sin((1/2).*( ...
  1+(-1).*t).*theta)+q11.*sin((1/2).*t.*theta)).*(q03.*sin((1/2).*(1+(-1) ...
  .*t).*theta)+q13.*sin((1/2).*t.*theta))+csc((1/2).*theta).^2.*(q02.*sin( ...
  (1/2).*(1+(-1).*t).*theta)+q12.*sin((1/2).*t.*theta)).*(q04.*sin((1/2).* ...
  (1+(-1).*t).*theta)+q14.*sin((1/2).*t.*theta))).^2+4.*((-1).*csc((1/2).* ...
  theta).^2.*(q01.*sin((1/2).*(1+(-1).*t).*theta)+q11.*sin((1/2).*t.* ...
  theta)).*(q02.*sin((1/2).*(1+(-1).*t).*theta)+q12.*sin((1/2).*t.*theta)) ...
  +csc((1/2).*theta).^2.*(q03.*sin((1/2).*(1+(-1).*t).*theta)+q13.*sin(( ...
  1/2).*t.*theta)).*(q04.*sin((1/2).*(1+(-1).*t).*theta)+q14.*sin((1/2).* ...
  t.*theta))).^2+(1+(-2).*(csc((1/2).*theta).^2.*(q02.*sin((1/2).*(1+(-1) ...
  .*t).*theta)+q12.*sin((1/2).*t.*theta)).^2+csc((1/2).*theta).^2.*(q03.* ...
  sin((1/2).*(1+(-1).*t).*theta)+q13.*sin((1/2).*t.*theta)).^2)).^2).^( ...
  1/2).*((1/2).*(1+(-2).*(csc((1/2).*theta).^2.*(q03.*sin((1/2).*(1+(-1).* ...
  t).*theta)+q13.*sin((1/2).*t.*theta)).^2+csc((1/2).*theta).^2.*(q04.* ...
  sin((1/2).*(1+(-1).*t).*theta)+q14.*sin((1/2).*t.*theta)).^2)).*(8.*((( ...
  -1/2).*q03.*theta.*cos((1/2).*(1+(-1).*t).*theta)+(1/2).*q13.*theta.* ...
  cos((1/2).*t.*theta)).*csc((1/2).*theta).^2.*(q01.*sin((1/2).*(1+(-1).* ...
  t).*theta)+q11.*sin((1/2).*t.*theta))+((-1/2).*q04.*theta.*cos((1/2).*( ...
  1+(-1).*t).*theta)+(1/2).*q14.*theta.*cos((1/2).*t.*theta)).*csc((1/2).* ...
  theta).^2.*(q02.*sin((1/2).*(1+(-1).*t).*theta)+q12.*sin((1/2).*t.* ...
  theta))+((-1/2).*q01.*theta.*cos((1/2).*(1+(-1).*t).*theta)+(1/2).*q11.* ...
  theta.*cos((1/2).*t.*theta)).*csc((1/2).*theta).^2.*(q03.*sin((1/2).*(1+ ...
  (-1).*t).*theta)+q13.*sin((1/2).*t.*theta))+((-1/2).*q02.*theta.*cos(( ...
  1/2).*(1+(-1).*t).*theta)+(1/2).*q12.*theta.*cos((1/2).*t.*theta)).*csc( ...
  (1/2).*theta).^2.*(q04.*sin((1/2).*(1+(-1).*t).*theta)+q14.*sin((1/2).* ...
  t.*theta))).*(csc((1/2).*theta).^2.*(q01.*sin((1/2).*(1+(-1).*t).*theta) ...
  +q11.*sin((1/2).*t.*theta)).*(q03.*sin((1/2).*(1+(-1).*t).*theta)+q13.* ...
  sin((1/2).*t.*theta))+csc((1/2).*theta).^2.*(q02.*sin((1/2).*(1+(-1).*t) ...
  .*theta)+q12.*sin((1/2).*t.*theta)).*(q04.*sin((1/2).*(1+(-1).*t).* ...
  theta)+q14.*sin((1/2).*t.*theta)))+8.*((-1).*((-1/2).*q02.*theta.*cos(( ...
  1/2).*(1+(-1).*t).*theta)+(1/2).*q12.*theta.*cos((1/2).*t.*theta)).*csc( ...
  (1/2).*theta).^2.*(q01.*sin((1/2).*(1+(-1).*t).*theta)+q11.*sin((1/2).* ...
  t.*theta))+(-1).*((-1/2).*q01.*theta.*cos((1/2).*(1+(-1).*t).*theta)+( ...
  1/2).*q11.*theta.*cos((1/2).*t.*theta)).*csc((1/2).*theta).^2.*(q02.* ...
  sin((1/2).*(1+(-1).*t).*theta)+q12.*sin((1/2).*t.*theta))+((-1/2).*q04.* ...
  theta.*cos((1/2).*(1+(-1).*t).*theta)+(1/2).*q14.*theta.*cos((1/2).*t.* ...
  theta)).*csc((1/2).*theta).^2.*(q03.*sin((1/2).*(1+(-1).*t).*theta)+ ...
  q13.*sin((1/2).*t.*theta))+((-1/2).*q03.*theta.*cos((1/2).*(1+(-1).*t).* ...
  theta)+(1/2).*q13.*theta.*cos((1/2).*t.*theta)).*csc((1/2).*theta).^2.*( ...
  q04.*sin((1/2).*(1+(-1).*t).*theta)+q14.*sin((1/2).*t.*theta))).*((-1).* ...
  csc((1/2).*theta).^2.*(q01.*sin((1/2).*(1+(-1).*t).*theta)+q11.*sin(( ...
  1/2).*t.*theta)).*(q02.*sin((1/2).*(1+(-1).*t).*theta)+q12.*sin((1/2).* ...
  t.*theta))+csc((1/2).*theta).^2.*(q03.*sin((1/2).*(1+(-1).*t).*theta)+ ...
  q13.*sin((1/2).*t.*theta)).*(q04.*sin((1/2).*(1+(-1).*t).*theta)+q14.* ...
  sin((1/2).*t.*theta)))+(-4).*(2.*((-1/2).*q02.*theta.*cos((1/2).*(1+(-1) ...
  .*t).*theta)+(1/2).*q12.*theta.*cos((1/2).*t.*theta)).*csc((1/2).*theta) ...
  .^2.*(q02.*sin((1/2).*(1+(-1).*t).*theta)+q12.*sin((1/2).*t.*theta))+2.* ...
  ((-1/2).*q03.*theta.*cos((1/2).*(1+(-1).*t).*theta)+(1/2).*q13.*theta.* ...
  cos((1/2).*t.*theta)).*csc((1/2).*theta).^2.*(q03.*sin((1/2).*(1+(-1).* ...
  t).*theta)+q13.*sin((1/2).*t.*theta))).*(1+(-2).*(csc((1/2).*theta).^2.* ...
  (q02.*sin((1/2).*(1+(-1).*t).*theta)+q12.*sin((1/2).*t.*theta)).^2+csc(( ...
  1/2).*theta).^2.*(q03.*sin((1/2).*(1+(-1).*t).*theta)+q13.*sin((1/2).* ...
  t.*theta)).^2))).*(4.*((-1).*csc((1/2).*theta).^2.*(q01.*sin((1/2).*(1+( ...
  -1).*t).*theta)+q11.*sin((1/2).*t.*theta)).*(q02.*sin((1/2).*(1+(-1).*t) ...
  .*theta)+q12.*sin((1/2).*t.*theta))+csc((1/2).*theta).^2.*(q03.*sin(( ...
  1/2).*(1+(-1).*t).*theta)+q13.*sin((1/2).*t.*theta)).*(q04.*sin((1/2).*( ...
  1+(-1).*t).*theta)+q14.*sin((1/2).*t.*theta))).^2+(1+(-2).*(csc((1/2).* ...
  theta).^2.*(q02.*sin((1/2).*(1+(-1).*t).*theta)+q12.*sin((1/2).*t.* ...
  theta)).^2+csc((1/2).*theta).^2.*(q03.*sin((1/2).*(1+(-1).*t).*theta)+ ...
  q13.*sin((1/2).*t.*theta)).^2)).^2).^(-1/2).*(4.*(csc((1/2).*theta).^2.* ...
  (q01.*sin((1/2).*(1+(-1).*t).*theta)+q11.*sin((1/2).*t.*theta)).*(q03.* ...
  sin((1/2).*(1+(-1).*t).*theta)+q13.*sin((1/2).*t.*theta))+csc((1/2).* ...
  theta).^2.*(q02.*sin((1/2).*(1+(-1).*t).*theta)+q12.*sin((1/2).*t.* ...
  theta)).*(q04.*sin((1/2).*(1+(-1).*t).*theta)+q14.*sin((1/2).*t.*theta)) ...
  ).^2+4.*((-1).*csc((1/2).*theta).^2.*(q01.*sin((1/2).*(1+(-1).*t).* ...
  theta)+q11.*sin((1/2).*t.*theta)).*(q02.*sin((1/2).*(1+(-1).*t).*theta)+ ...
  q12.*sin((1/2).*t.*theta))+csc((1/2).*theta).^2.*(q03.*sin((1/2).*(1+( ...
  -1).*t).*theta)+q13.*sin((1/2).*t.*theta)).*(q04.*sin((1/2).*(1+(-1).*t) ...
  .*theta)+q14.*sin((1/2).*t.*theta))).^2+(1+(-2).*(csc((1/2).*theta).^2.* ...
  (q02.*sin((1/2).*(1+(-1).*t).*theta)+q12.*sin((1/2).*t.*theta)).^2+csc(( ...
  1/2).*theta).^2.*(q03.*sin((1/2).*(1+(-1).*t).*theta)+q13.*sin((1/2).* ...
  t.*theta)).^2)).^2).^(-1/2)+(-1/2).*(1+(-2).*(csc((1/2).*theta).^2.*( ...
  q03.*sin((1/2).*(1+(-1).*t).*theta)+q13.*sin((1/2).*t.*theta)).^2+csc(( ...
  1/2).*theta).^2.*(q04.*sin((1/2).*(1+(-1).*t).*theta)+q14.*sin((1/2).* ...
  t.*theta)).^2)).*(8.*((-1).*((-1/2).*q02.*theta.*cos((1/2).*(1+(-1).*t) ...
  .*theta)+(1/2).*q12.*theta.*cos((1/2).*t.*theta)).*csc((1/2).*theta) ...
  .^2.*(q01.*sin((1/2).*(1+(-1).*t).*theta)+q11.*sin((1/2).*t.*theta))+( ...
  -1).*((-1/2).*q01.*theta.*cos((1/2).*(1+(-1).*t).*theta)+(1/2).*q11.* ...
  theta.*cos((1/2).*t.*theta)).*csc((1/2).*theta).^2.*(q02.*sin((1/2).*(1+ ...
  (-1).*t).*theta)+q12.*sin((1/2).*t.*theta))+((-1/2).*q04.*theta.*cos(( ...
  1/2).*(1+(-1).*t).*theta)+(1/2).*q14.*theta.*cos((1/2).*t.*theta)).*csc( ...
  (1/2).*theta).^2.*(q03.*sin((1/2).*(1+(-1).*t).*theta)+q13.*sin((1/2).* ...
  t.*theta))+((-1/2).*q03.*theta.*cos((1/2).*(1+(-1).*t).*theta)+(1/2).* ...
  q13.*theta.*cos((1/2).*t.*theta)).*csc((1/2).*theta).^2.*(q04.*sin((1/2) ...
  .*(1+(-1).*t).*theta)+q14.*sin((1/2).*t.*theta))).*((-1).*csc((1/2).* ...
  theta).^2.*(q01.*sin((1/2).*(1+(-1).*t).*theta)+q11.*sin((1/2).*t.* ...
  theta)).*(q02.*sin((1/2).*(1+(-1).*t).*theta)+q12.*sin((1/2).*t.*theta)) ...
  +csc((1/2).*theta).^2.*(q03.*sin((1/2).*(1+(-1).*t).*theta)+q13.*sin(( ...
  1/2).*t.*theta)).*(q04.*sin((1/2).*(1+(-1).*t).*theta)+q14.*sin((1/2).* ...
  t.*theta)))+(-4).*(2.*((-1/2).*q02.*theta.*cos((1/2).*(1+(-1).*t).* ...
  theta)+(1/2).*q12.*theta.*cos((1/2).*t.*theta)).*csc((1/2).*theta).^2.*( ...
  q02.*sin((1/2).*(1+(-1).*t).*theta)+q12.*sin((1/2).*t.*theta))+2.*(( ...
  -1/2).*q03.*theta.*cos((1/2).*(1+(-1).*t).*theta)+(1/2).*q13.*theta.* ...
  cos((1/2).*t.*theta)).*csc((1/2).*theta).^2.*(q03.*sin((1/2).*(1+(-1).* ...
  t).*theta)+q13.*sin((1/2).*t.*theta))).*(1+(-2).*(csc((1/2).*theta).^2.* ...
  (q02.*sin((1/2).*(1+(-1).*t).*theta)+q12.*sin((1/2).*t.*theta)).^2+csc(( ...
  1/2).*theta).^2.*(q03.*sin((1/2).*(1+(-1).*t).*theta)+q13.*sin((1/2).* ...
  t.*theta)).^2))).*(4.*((-1).*csc((1/2).*theta).^2.*(q01.*sin((1/2).*(1+( ...
  -1).*t).*theta)+q11.*sin((1/2).*t.*theta)).*(q02.*sin((1/2).*(1+(-1).*t) ...
  .*theta)+q12.*sin((1/2).*t.*theta))+csc((1/2).*theta).^2.*(q03.*sin(( ...
  1/2).*(1+(-1).*t).*theta)+q13.*sin((1/2).*t.*theta)).*(q04.*sin((1/2).*( ...
  1+(-1).*t).*theta)+q14.*sin((1/2).*t.*theta))).^2+(1+(-2).*(csc((1/2).* ...
  theta).^2.*(q02.*sin((1/2).*(1+(-1).*t).*theta)+q12.*sin((1/2).*t.* ...
  theta)).^2+csc((1/2).*theta).^2.*(q03.*sin((1/2).*(1+(-1).*t).*theta)+ ...
  q13.*sin((1/2).*t.*theta)).^2)).^2).^(-3/2).*(4.*(csc((1/2).*theta).^2.* ...
  (q01.*sin((1/2).*(1+(-1).*t).*theta)+q11.*sin((1/2).*t.*theta)).*(q03.* ...
  sin((1/2).*(1+(-1).*t).*theta)+q13.*sin((1/2).*t.*theta))+csc((1/2).* ...
  theta).^2.*(q02.*sin((1/2).*(1+(-1).*t).*theta)+q12.*sin((1/2).*t.* ...
  theta)).*(q04.*sin((1/2).*(1+(-1).*t).*theta)+q14.*sin((1/2).*t.*theta)) ...
  ).^2+4.*((-1).*csc((1/2).*theta).^2.*(q01.*sin((1/2).*(1+(-1).*t).* ...
  theta)+q11.*sin((1/2).*t.*theta)).*(q02.*sin((1/2).*(1+(-1).*t).*theta)+ ...
  q12.*sin((1/2).*t.*theta))+csc((1/2).*theta).^2.*(q03.*sin((1/2).*(1+( ...
  -1).*t).*theta)+q13.*sin((1/2).*t.*theta)).*(q04.*sin((1/2).*(1+(-1).*t) ...
  .*theta)+q14.*sin((1/2).*t.*theta))).^2+(1+(-2).*(csc((1/2).*theta).^2.* ...
  (q02.*sin((1/2).*(1+(-1).*t).*theta)+q12.*sin((1/2).*t.*theta)).^2+csc(( ...
  1/2).*theta).^2.*(q03.*sin((1/2).*(1+(-1).*t).*theta)+q13.*sin((1/2).* ...
  t.*theta)).^2)).^2).^(1/2)+(-2).*(2.*((-1/2).*q03.*theta.*cos((1/2).*(1+ ...
  (-1).*t).*theta)+(1/2).*q13.*theta.*cos((1/2).*t.*theta)).*csc((1/2).* ...
  theta).^2.*(q03.*sin((1/2).*(1+(-1).*t).*theta)+q13.*sin((1/2).*t.* ...
  theta))+2.*((-1/2).*q04.*theta.*cos((1/2).*(1+(-1).*t).*theta)+(1/2).* ...
  q14.*theta.*cos((1/2).*t.*theta)).*csc((1/2).*theta).^2.*(q04.*sin((1/2) ...
  .*(1+(-1).*t).*theta)+q14.*sin((1/2).*t.*theta))).*(4.*((-1).*csc((1/2) ...
  .*theta).^2.*(q01.*sin((1/2).*(1+(-1).*t).*theta)+q11.*sin((1/2).*t.* ...
  theta)).*(q02.*sin((1/2).*(1+(-1).*t).*theta)+q12.*sin((1/2).*t.*theta)) ...
  +csc((1/2).*theta).^2.*(q03.*sin((1/2).*(1+(-1).*t).*theta)+q13.*sin(( ...
  1/2).*t.*theta)).*(q04.*sin((1/2).*(1+(-1).*t).*theta)+q14.*sin((1/2).* ...
  t.*theta))).^2+(1+(-2).*(csc((1/2).*theta).^2.*(q02.*sin((1/2).*(1+(-1) ...
  .*t).*theta)+q12.*sin((1/2).*t.*theta)).^2+csc((1/2).*theta).^2.*(q03.* ...
  sin((1/2).*(1+(-1).*t).*theta)+q13.*sin((1/2).*t.*theta)).^2)).^2).^( ...
  -1/2).*(4.*(csc((1/2).*theta).^2.*(q01.*sin((1/2).*(1+(-1).*t).*theta)+ ...
  q11.*sin((1/2).*t.*theta)).*(q03.*sin((1/2).*(1+(-1).*t).*theta)+q13.* ...
  sin((1/2).*t.*theta))+csc((1/2).*theta).^2.*(q02.*sin((1/2).*(1+(-1).*t) ...
  .*theta)+q12.*sin((1/2).*t.*theta)).*(q04.*sin((1/2).*(1+(-1).*t).* ...
  theta)+q14.*sin((1/2).*t.*theta))).^2+4.*((-1).*csc((1/2).*theta).^2.*( ...
  q01.*sin((1/2).*(1+(-1).*t).*theta)+q11.*sin((1/2).*t.*theta)).*(q02.* ...
  sin((1/2).*(1+(-1).*t).*theta)+q12.*sin((1/2).*t.*theta))+csc((1/2).* ...
  theta).^2.*(q03.*sin((1/2).*(1+(-1).*t).*theta)+q13.*sin((1/2).*t.* ...
  theta)).*(q04.*sin((1/2).*(1+(-1).*t).*theta)+q14.*sin((1/2).*t.*theta)) ...
  ).^2+(1+(-2).*(csc((1/2).*theta).^2.*(q02.*sin((1/2).*(1+(-1).*t).* ...
  theta)+q12.*sin((1/2).*t.*theta)).^2+csc((1/2).*theta).^2.*(q03.*sin(( ...
  1/2).*(1+(-1).*t).*theta)+q13.*sin((1/2).*t.*theta)).^2)).^2).^(1/2)).*( ...
  4.*(csc((1/2).*theta).^2.*(q02.*sin((1/2).*(1+(-1).*t).*theta)+q12.*sin( ...
  (1/2).*t.*theta)).*(q03.*sin((1/2).*(1+(-1).*t).*theta)+q13.*sin((1/2).* ...
  t.*theta))+(-1).*csc((1/2).*theta).^2.*(q01.*sin((1/2).*(1+(-1).*t).* ...
  theta)+q11.*sin((1/2).*t.*theta)).*(q04.*sin((1/2).*(1+(-1).*t).*theta)+ ...
  q14.*sin((1/2).*t.*theta))).^2.*(4.*((-1).*csc((1/2).*theta).^2.*(q01.* ...
  sin((1/2).*(1+(-1).*t).*theta)+q11.*sin((1/2).*t.*theta)).*(q02.*sin(( ...
  1/2).*(1+(-1).*t).*theta)+q12.*sin((1/2).*t.*theta))+csc((1/2).*theta) ...
  .^2.*(q03.*sin((1/2).*(1+(-1).*t).*theta)+q13.*sin((1/2).*t.*theta)).*( ...
  q04.*sin((1/2).*(1+(-1).*t).*theta)+q14.*sin((1/2).*t.*theta))).^2+(1+( ...
  -2).*(csc((1/2).*theta).^2.*(q02.*sin((1/2).*(1+(-1).*t).*theta)+q12.* ...
  sin((1/2).*t.*theta)).^2+csc((1/2).*theta).^2.*(q03.*sin((1/2).*(1+(-1) ...
  .*t).*theta)+q13.*sin((1/2).*t.*theta)).^2)).^2).^(-1).*(4.*(csc((1/2).* ...
  theta).^2.*(q01.*sin((1/2).*(1+(-1).*t).*theta)+q11.*sin((1/2).*t.* ...
  theta)).*(q03.*sin((1/2).*(1+(-1).*t).*theta)+q13.*sin((1/2).*t.*theta)) ...
  +csc((1/2).*theta).^2.*(q02.*sin((1/2).*(1+(-1).*t).*theta)+q12.*sin(( ...
  1/2).*t.*theta)).*(q04.*sin((1/2).*(1+(-1).*t).*theta)+q14.*sin((1/2).* ...
  t.*theta))).^2+4.*((-1).*csc((1/2).*theta).^2.*(q01.*sin((1/2).*(1+(-1) ...
  .*t).*theta)+q11.*sin((1/2).*t.*theta)).*(q02.*sin((1/2).*(1+(-1).*t).* ...
  theta)+q12.*sin((1/2).*t.*theta))+csc((1/2).*theta).^2.*(q03.*sin((1/2) ...
  .*(1+(-1).*t).*theta)+q13.*sin((1/2).*t.*theta)).*(q04.*sin((1/2).*(1+( ...
  -1).*t).*theta)+q14.*sin((1/2).*t.*theta))).^2+(1+(-2).*(csc((1/2).* ...
  theta).^2.*(q02.*sin((1/2).*(1+(-1).*t).*theta)+q12.*sin((1/2).*t.* ...
  theta)).^2+csc((1/2).*theta).^2.*(q03.*sin((1/2).*(1+(-1).*t).*theta)+ ...
  q13.*sin((1/2).*t.*theta)).^2)).^2)+(1+(-2).*(csc((1/2).*theta).^2.*( ...
  q03.*sin((1/2).*(1+(-1).*t).*theta)+q13.*sin((1/2).*t.*theta)).^2+csc(( ...
  1/2).*theta).^2.*(q04.*sin((1/2).*(1+(-1).*t).*theta)+q14.*sin((1/2).* ...
  t.*theta)).^2)).^2.*(4.*((-1).*csc((1/2).*theta).^2.*(q01.*sin((1/2).*( ...
  1+(-1).*t).*theta)+q11.*sin((1/2).*t.*theta)).*(q02.*sin((1/2).*(1+(-1) ...
  .*t).*theta)+q12.*sin((1/2).*t.*theta))+csc((1/2).*theta).^2.*(q03.*sin( ...
  (1/2).*(1+(-1).*t).*theta)+q13.*sin((1/2).*t.*theta)).*(q04.*sin((1/2).* ...
  (1+(-1).*t).*theta)+q14.*sin((1/2).*t.*theta))).^2+(1+(-2).*(csc((1/2).* ...
  theta).^2.*(q02.*sin((1/2).*(1+(-1).*t).*theta)+q12.*sin((1/2).*t.* ...
  theta)).^2+csc((1/2).*theta).^2.*(q03.*sin((1/2).*(1+(-1).*t).*theta)+ ...
  q13.*sin((1/2).*t.*theta)).^2)).^2).^(-1).*(4.*(csc((1/2).*theta).^2.*( ...
  q01.*sin((1/2).*(1+(-1).*t).*theta)+q11.*sin((1/2).*t.*theta)).*(q03.* ...
  sin((1/2).*(1+(-1).*t).*theta)+q13.*sin((1/2).*t.*theta))+csc((1/2).* ...
  theta).^2.*(q02.*sin((1/2).*(1+(-1).*t).*theta)+q12.*sin((1/2).*t.* ...
  theta)).*(q04.*sin((1/2).*(1+(-1).*t).*theta)+q14.*sin((1/2).*t.*theta)) ...
  ).^2+4.*((-1).*csc((1/2).*theta).^2.*(q01.*sin((1/2).*(1+(-1).*t).* ...
  theta)+q11.*sin((1/2).*t.*theta)).*(q02.*sin((1/2).*(1+(-1).*t).*theta)+ ...
  q12.*sin((1/2).*t.*theta))+csc((1/2).*theta).^2.*(q03.*sin((1/2).*(1+( ...
  -1).*t).*theta)+q13.*sin((1/2).*t.*theta)).*(q04.*sin((1/2).*(1+(-1).*t) ...
  .*theta)+q14.*sin((1/2).*t.*theta))).^2+(1+(-2).*(csc((1/2).*theta).^2.* ...
  (q02.*sin((1/2).*(1+(-1).*t).*theta)+q12.*sin((1/2).*t.*theta)).^2+csc(( ...
  1/2).*theta).^2.*(q03.*sin((1/2).*(1+(-1).*t).*theta)+q13.*sin((1/2).* ...
  t.*theta)).^2)).^2)).^(-1)+(1+(-2).*(csc((1/2).*theta).^2.*(q03.*sin(( ...
  1/2).*(1+(-1).*t).*theta)+q13.*sin((1/2).*t.*theta)).^2+csc((1/2).* ...
  theta).^2.*(q04.*sin((1/2).*(1+(-1).*t).*theta)+q14.*sin((1/2).*t.* ...
  theta)).^2)).*(4.*((-1).*csc((1/2).*theta).^2.*(q01.*sin((1/2).*(1+(-1) ...
  .*t).*theta)+q11.*sin((1/2).*t.*theta)).*(q02.*sin((1/2).*(1+(-1).*t).* ...
  theta)+q12.*sin((1/2).*t.*theta))+csc((1/2).*theta).^2.*(q03.*sin((1/2) ...
  .*(1+(-1).*t).*theta)+q13.*sin((1/2).*t.*theta)).*(q04.*sin((1/2).*(1+( ...
  -1).*t).*theta)+q14.*sin((1/2).*t.*theta))).^2+(1+(-2).*(csc((1/2).* ...
  theta).^2.*(q02.*sin((1/2).*(1+(-1).*t).*theta)+q12.*sin((1/2).*t.* ...
  theta)).^2+csc((1/2).*theta).^2.*(q03.*sin((1/2).*(1+(-1).*t).*theta)+ ...
  q13.*sin((1/2).*t.*theta)).^2)).^2).^(-1/2).*(4.*(csc((1/2).*theta).^2.* ...
  (q01.*sin((1/2).*(1+(-1).*t).*theta)+q11.*sin((1/2).*t.*theta)).*(q03.* ...
  sin((1/2).*(1+(-1).*t).*theta)+q13.*sin((1/2).*t.*theta))+csc((1/2).* ...
  theta).^2.*(q02.*sin((1/2).*(1+(-1).*t).*theta)+q12.*sin((1/2).*t.* ...
  theta)).*(q04.*sin((1/2).*(1+(-1).*t).*theta)+q14.*sin((1/2).*t.*theta)) ...
  ).^2+4.*((-1).*csc((1/2).*theta).^2.*(q01.*sin((1/2).*(1+(-1).*t).* ...
  theta)+q11.*sin((1/2).*t.*theta)).*(q02.*sin((1/2).*(1+(-1).*t).*theta)+ ...
  q12.*sin((1/2).*t.*theta))+csc((1/2).*theta).^2.*(q03.*sin((1/2).*(1+( ...
  -1).*t).*theta)+q13.*sin((1/2).*t.*theta)).*(q04.*sin((1/2).*(1+(-1).*t) ...
  .*theta)+q14.*sin((1/2).*t.*theta))).^2+(1+(-2).*(csc((1/2).*theta).^2.* ...
  (q02.*sin((1/2).*(1+(-1).*t).*theta)+q12.*sin((1/2).*t.*theta)).^2+csc(( ...
  1/2).*theta).^2.*(q03.*sin((1/2).*(1+(-1).*t).*theta)+q13.*sin((1/2).* ...
  t.*theta)).^2)).^2).^(1/2).*((1/2).*(csc((1/2).*theta).^2.*(q02.*sin(( ...
  1/2).*(1+(-1).*t).*theta)+q12.*sin((1/2).*t.*theta)).*(q03.*sin((1/2).*( ...
  1+(-1).*t).*theta)+q13.*sin((1/2).*t.*theta))+(-1).*csc((1/2).*theta) ...
  .^2.*(q01.*sin((1/2).*(1+(-1).*t).*theta)+q11.*sin((1/2).*t.*theta)).*( ...
  q04.*sin((1/2).*(1+(-1).*t).*theta)+q14.*sin((1/2).*t.*theta))).*(8.*((( ...
  -1/2).*q03.*theta.*cos((1/2).*(1+(-1).*t).*theta)+(1/2).*q13.*theta.* ...
  cos((1/2).*t.*theta)).*csc((1/2).*theta).^2.*(q01.*sin((1/2).*(1+(-1).* ...
  t).*theta)+q11.*sin((1/2).*t.*theta))+((-1/2).*q04.*theta.*cos((1/2).*( ...
  1+(-1).*t).*theta)+(1/2).*q14.*theta.*cos((1/2).*t.*theta)).*csc((1/2).* ...
  theta).^2.*(q02.*sin((1/2).*(1+(-1).*t).*theta)+q12.*sin((1/2).*t.* ...
  theta))+((-1/2).*q01.*theta.*cos((1/2).*(1+(-1).*t).*theta)+(1/2).*q11.* ...
  theta.*cos((1/2).*t.*theta)).*csc((1/2).*theta).^2.*(q03.*sin((1/2).*(1+ ...
  (-1).*t).*theta)+q13.*sin((1/2).*t.*theta))+((-1/2).*q02.*theta.*cos(( ...
  1/2).*(1+(-1).*t).*theta)+(1/2).*q12.*theta.*cos((1/2).*t.*theta)).*csc( ...
  (1/2).*theta).^2.*(q04.*sin((1/2).*(1+(-1).*t).*theta)+q14.*sin((1/2).* ...
  t.*theta))).*(csc((1/2).*theta).^2.*(q01.*sin((1/2).*(1+(-1).*t).*theta) ...
  +q11.*sin((1/2).*t.*theta)).*(q03.*sin((1/2).*(1+(-1).*t).*theta)+q13.* ...
  sin((1/2).*t.*theta))+csc((1/2).*theta).^2.*(q02.*sin((1/2).*(1+(-1).*t) ...
  .*theta)+q12.*sin((1/2).*t.*theta)).*(q04.*sin((1/2).*(1+(-1).*t).* ...
  theta)+q14.*sin((1/2).*t.*theta)))+8.*((-1).*((-1/2).*q02.*theta.*cos(( ...
  1/2).*(1+(-1).*t).*theta)+(1/2).*q12.*theta.*cos((1/2).*t.*theta)).*csc( ...
  (1/2).*theta).^2.*(q01.*sin((1/2).*(1+(-1).*t).*theta)+q11.*sin((1/2).* ...
  t.*theta))+(-1).*((-1/2).*q01.*theta.*cos((1/2).*(1+(-1).*t).*theta)+( ...
  1/2).*q11.*theta.*cos((1/2).*t.*theta)).*csc((1/2).*theta).^2.*(q02.* ...
  sin((1/2).*(1+(-1).*t).*theta)+q12.*sin((1/2).*t.*theta))+((-1/2).*q04.* ...
  theta.*cos((1/2).*(1+(-1).*t).*theta)+(1/2).*q14.*theta.*cos((1/2).*t.* ...
  theta)).*csc((1/2).*theta).^2.*(q03.*sin((1/2).*(1+(-1).*t).*theta)+ ...
  q13.*sin((1/2).*t.*theta))+((-1/2).*q03.*theta.*cos((1/2).*(1+(-1).*t).* ...
  theta)+(1/2).*q13.*theta.*cos((1/2).*t.*theta)).*csc((1/2).*theta).^2.*( ...
  q04.*sin((1/2).*(1+(-1).*t).*theta)+q14.*sin((1/2).*t.*theta))).*((-1).* ...
  csc((1/2).*theta).^2.*(q01.*sin((1/2).*(1+(-1).*t).*theta)+q11.*sin(( ...
  1/2).*t.*theta)).*(q02.*sin((1/2).*(1+(-1).*t).*theta)+q12.*sin((1/2).* ...
  t.*theta))+csc((1/2).*theta).^2.*(q03.*sin((1/2).*(1+(-1).*t).*theta)+ ...
  q13.*sin((1/2).*t.*theta)).*(q04.*sin((1/2).*(1+(-1).*t).*theta)+q14.* ...
  sin((1/2).*t.*theta)))+(-4).*(2.*((-1/2).*q02.*theta.*cos((1/2).*(1+(-1) ...
  .*t).*theta)+(1/2).*q12.*theta.*cos((1/2).*t.*theta)).*csc((1/2).*theta) ...
  .^2.*(q02.*sin((1/2).*(1+(-1).*t).*theta)+q12.*sin((1/2).*t.*theta))+2.* ...
  ((-1/2).*q03.*theta.*cos((1/2).*(1+(-1).*t).*theta)+(1/2).*q13.*theta.* ...
  cos((1/2).*t.*theta)).*csc((1/2).*theta).^2.*(q03.*sin((1/2).*(1+(-1).* ...
  t).*theta)+q13.*sin((1/2).*t.*theta))).*(1+(-2).*(csc((1/2).*theta).^2.* ...
  (q02.*sin((1/2).*(1+(-1).*t).*theta)+q12.*sin((1/2).*t.*theta)).^2+csc(( ...
  1/2).*theta).^2.*(q03.*sin((1/2).*(1+(-1).*t).*theta)+q13.*sin((1/2).* ...
  t.*theta)).^2))).^2.*(4.*((-1).*csc((1/2).*theta).^2.*(q01.*sin((1/2).*( ...
  1+(-1).*t).*theta)+q11.*sin((1/2).*t.*theta)).*(q02.*sin((1/2).*(1+(-1) ...
  .*t).*theta)+q12.*sin((1/2).*t.*theta))+csc((1/2).*theta).^2.*(q03.*sin( ...
  (1/2).*(1+(-1).*t).*theta)+q13.*sin((1/2).*t.*theta)).*(q04.*sin((1/2).* ...
  (1+(-1).*t).*theta)+q14.*sin((1/2).*t.*theta))).^2+(1+(-2).*(csc((1/2).* ...
  theta).^2.*(q02.*sin((1/2).*(1+(-1).*t).*theta)+q12.*sin((1/2).*t.* ...
  theta)).^2+csc((1/2).*theta).^2.*(q03.*sin((1/2).*(1+(-1).*t).*theta)+ ...
  q13.*sin((1/2).*t.*theta)).^2)).^2).^(-1/2).*(4.*(csc((1/2).*theta).^2.* ...
  (q01.*sin((1/2).*(1+(-1).*t).*theta)+q11.*sin((1/2).*t.*theta)).*(q03.* ...
  sin((1/2).*(1+(-1).*t).*theta)+q13.*sin((1/2).*t.*theta))+csc((1/2).* ...
  theta).^2.*(q02.*sin((1/2).*(1+(-1).*t).*theta)+q12.*sin((1/2).*t.* ...
  theta)).*(q04.*sin((1/2).*(1+(-1).*t).*theta)+q14.*sin((1/2).*t.*theta)) ...
  ).^2+4.*((-1).*csc((1/2).*theta).^2.*(q01.*sin((1/2).*(1+(-1).*t).* ...
  theta)+q11.*sin((1/2).*t.*theta)).*(q02.*sin((1/2).*(1+(-1).*t).*theta)+ ...
  q12.*sin((1/2).*t.*theta))+csc((1/2).*theta).^2.*(q03.*sin((1/2).*(1+( ...
  -1).*t).*theta)+q13.*sin((1/2).*t.*theta)).*(q04.*sin((1/2).*(1+(-1).*t) ...
  .*theta)+q14.*sin((1/2).*t.*theta))).^2+(1+(-2).*(csc((1/2).*theta).^2.* ...
  (q02.*sin((1/2).*(1+(-1).*t).*theta)+q12.*sin((1/2).*t.*theta)).^2+csc(( ...
  1/2).*theta).^2.*(q03.*sin((1/2).*(1+(-1).*t).*theta)+q13.*sin((1/2).* ...
  t.*theta)).^2)).^2).^(-3/2)+(csc((1/2).*theta).^2.*(q02.*sin((1/2).*(1+( ...
  -1).*t).*theta)+q12.*sin((1/2).*t.*theta)).*(q03.*sin((1/2).*(1+(-1).*t) ...
  .*theta)+q13.*sin((1/2).*t.*theta))+(-1).*csc((1/2).*theta).^2.*(q01.* ...
  sin((1/2).*(1+(-1).*t).*theta)+q11.*sin((1/2).*t.*theta)).*(q04.*sin(( ...
  1/2).*(1+(-1).*t).*theta)+q14.*sin((1/2).*t.*theta))).*(8.*((-1).*(( ...
  -1/2).*q02.*theta.*cos((1/2).*(1+(-1).*t).*theta)+(1/2).*q12.*theta.* ...
  cos((1/2).*t.*theta)).*csc((1/2).*theta).^2.*(q01.*sin((1/2).*(1+(-1).* ...
  t).*theta)+q11.*sin((1/2).*t.*theta))+(-1).*((-1/2).*q01.*theta.*cos(( ...
  1/2).*(1+(-1).*t).*theta)+(1/2).*q11.*theta.*cos((1/2).*t.*theta)).*csc( ...
  (1/2).*theta).^2.*(q02.*sin((1/2).*(1+(-1).*t).*theta)+q12.*sin((1/2).* ...
  t.*theta))+((-1/2).*q04.*theta.*cos((1/2).*(1+(-1).*t).*theta)+(1/2).* ...
  q14.*theta.*cos((1/2).*t.*theta)).*csc((1/2).*theta).^2.*(q03.*sin((1/2) ...
  .*(1+(-1).*t).*theta)+q13.*sin((1/2).*t.*theta))+((-1/2).*q03.*theta.* ...
  cos((1/2).*(1+(-1).*t).*theta)+(1/2).*q13.*theta.*cos((1/2).*t.*theta)) ...
  .*csc((1/2).*theta).^2.*(q04.*sin((1/2).*(1+(-1).*t).*theta)+q14.*sin(( ...
  1/2).*t.*theta))).*((-1).*csc((1/2).*theta).^2.*(q01.*sin((1/2).*(1+(-1) ...
  .*t).*theta)+q11.*sin((1/2).*t.*theta)).*(q02.*sin((1/2).*(1+(-1).*t).* ...
  theta)+q12.*sin((1/2).*t.*theta))+csc((1/2).*theta).^2.*(q03.*sin((1/2) ...
  .*(1+(-1).*t).*theta)+q13.*sin((1/2).*t.*theta)).*(q04.*sin((1/2).*(1+( ...
  -1).*t).*theta)+q14.*sin((1/2).*t.*theta)))+(-4).*(2.*((-1/2).*q02.* ...
  theta.*cos((1/2).*(1+(-1).*t).*theta)+(1/2).*q12.*theta.*cos((1/2).*t.* ...
  theta)).*csc((1/2).*theta).^2.*(q02.*sin((1/2).*(1+(-1).*t).*theta)+ ...
  q12.*sin((1/2).*t.*theta))+2.*((-1/2).*q03.*theta.*cos((1/2).*(1+(-1).* ...
  t).*theta)+(1/2).*q13.*theta.*cos((1/2).*t.*theta)).*csc((1/2).*theta) ...
  .^2.*(q03.*sin((1/2).*(1+(-1).*t).*theta)+q13.*sin((1/2).*t.*theta))).*( ...
  1+(-2).*(csc((1/2).*theta).^2.*(q02.*sin((1/2).*(1+(-1).*t).*theta)+ ...
  q12.*sin((1/2).*t.*theta)).^2+csc((1/2).*theta).^2.*(q03.*sin((1/2).*(1+ ...
  (-1).*t).*theta)+q13.*sin((1/2).*t.*theta)).^2))).*(8.*(((-1/2).*q03.* ...
  theta.*cos((1/2).*(1+(-1).*t).*theta)+(1/2).*q13.*theta.*cos((1/2).*t.* ...
  theta)).*csc((1/2).*theta).^2.*(q01.*sin((1/2).*(1+(-1).*t).*theta)+ ...
  q11.*sin((1/2).*t.*theta))+((-1/2).*q04.*theta.*cos((1/2).*(1+(-1).*t).* ...
  theta)+(1/2).*q14.*theta.*cos((1/2).*t.*theta)).*csc((1/2).*theta).^2.*( ...
  q02.*sin((1/2).*(1+(-1).*t).*theta)+q12.*sin((1/2).*t.*theta))+((-1/2).* ...
  q01.*theta.*cos((1/2).*(1+(-1).*t).*theta)+(1/2).*q11.*theta.*cos((1/2) ...
  .*t.*theta)).*csc((1/2).*theta).^2.*(q03.*sin((1/2).*(1+(-1).*t).*theta) ...
  +q13.*sin((1/2).*t.*theta))+((-1/2).*q02.*theta.*cos((1/2).*(1+(-1).*t) ...
  .*theta)+(1/2).*q12.*theta.*cos((1/2).*t.*theta)).*csc((1/2).*theta) ...
  .^2.*(q04.*sin((1/2).*(1+(-1).*t).*theta)+q14.*sin((1/2).*t.*theta))).*( ...
  csc((1/2).*theta).^2.*(q01.*sin((1/2).*(1+(-1).*t).*theta)+q11.*sin(( ...
  1/2).*t.*theta)).*(q03.*sin((1/2).*(1+(-1).*t).*theta)+q13.*sin((1/2).* ...
  t.*theta))+csc((1/2).*theta).^2.*(q02.*sin((1/2).*(1+(-1).*t).*theta)+ ...
  q12.*sin((1/2).*t.*theta)).*(q04.*sin((1/2).*(1+(-1).*t).*theta)+q14.* ...
  sin((1/2).*t.*theta)))+8.*((-1).*((-1/2).*q02.*theta.*cos((1/2).*(1+(-1) ...
  .*t).*theta)+(1/2).*q12.*theta.*cos((1/2).*t.*theta)).*csc((1/2).*theta) ...
  .^2.*(q01.*sin((1/2).*(1+(-1).*t).*theta)+q11.*sin((1/2).*t.*theta))+( ...
  -1).*((-1/2).*q01.*theta.*cos((1/2).*(1+(-1).*t).*theta)+(1/2).*q11.* ...
  theta.*cos((1/2).*t.*theta)).*csc((1/2).*theta).^2.*(q02.*sin((1/2).*(1+ ...
  (-1).*t).*theta)+q12.*sin((1/2).*t.*theta))+((-1/2).*q04.*theta.*cos(( ...
  1/2).*(1+(-1).*t).*theta)+(1/2).*q14.*theta.*cos((1/2).*t.*theta)).*csc( ...
  (1/2).*theta).^2.*(q03.*sin((1/2).*(1+(-1).*t).*theta)+q13.*sin((1/2).* ...
  t.*theta))+((-1/2).*q03.*theta.*cos((1/2).*(1+(-1).*t).*theta)+(1/2).* ...
  q13.*theta.*cos((1/2).*t.*theta)).*csc((1/2).*theta).^2.*(q04.*sin((1/2) ...
  .*(1+(-1).*t).*theta)+q14.*sin((1/2).*t.*theta))).*((-1).*csc((1/2).* ...
  theta).^2.*(q01.*sin((1/2).*(1+(-1).*t).*theta)+q11.*sin((1/2).*t.* ...
  theta)).*(q02.*sin((1/2).*(1+(-1).*t).*theta)+q12.*sin((1/2).*t.*theta)) ...
  +csc((1/2).*theta).^2.*(q03.*sin((1/2).*(1+(-1).*t).*theta)+q13.*sin(( ...
  1/2).*t.*theta)).*(q04.*sin((1/2).*(1+(-1).*t).*theta)+q14.*sin((1/2).* ...
  t.*theta)))+(-4).*(2.*((-1/2).*q02.*theta.*cos((1/2).*(1+(-1).*t).* ...
  theta)+(1/2).*q12.*theta.*cos((1/2).*t.*theta)).*csc((1/2).*theta).^2.*( ...
  q02.*sin((1/2).*(1+(-1).*t).*theta)+q12.*sin((1/2).*t.*theta))+2.*(( ...
  -1/2).*q03.*theta.*cos((1/2).*(1+(-1).*t).*theta)+(1/2).*q13.*theta.* ...
  cos((1/2).*t.*theta)).*csc((1/2).*theta).^2.*(q03.*sin((1/2).*(1+(-1).* ...
  t).*theta)+q13.*sin((1/2).*t.*theta))).*(1+(-2).*(csc((1/2).*theta).^2.* ...
  (q02.*sin((1/2).*(1+(-1).*t).*theta)+q12.*sin((1/2).*t.*theta)).^2+csc(( ...
  1/2).*theta).^2.*(q03.*sin((1/2).*(1+(-1).*t).*theta)+q13.*sin((1/2).* ...
  t.*theta)).^2))).*(4.*((-1).*csc((1/2).*theta).^2.*(q01.*sin((1/2).*(1+( ...
  -1).*t).*theta)+q11.*sin((1/2).*t.*theta)).*(q02.*sin((1/2).*(1+(-1).*t) ...
  .*theta)+q12.*sin((1/2).*t.*theta))+csc((1/2).*theta).^2.*(q03.*sin(( ...
  1/2).*(1+(-1).*t).*theta)+q13.*sin((1/2).*t.*theta)).*(q04.*sin((1/2).*( ...
  1+(-1).*t).*theta)+q14.*sin((1/2).*t.*theta))).^2+(1+(-2).*(csc((1/2).* ...
  theta).^2.*(q02.*sin((1/2).*(1+(-1).*t).*theta)+q12.*sin((1/2).*t.* ...
  theta)).^2+csc((1/2).*theta).^2.*(q03.*sin((1/2).*(1+(-1).*t).*theta)+ ...
  q13.*sin((1/2).*t.*theta)).^2)).^2).^(-3/2).*(4.*(csc((1/2).*theta).^2.* ...
  (q01.*sin((1/2).*(1+(-1).*t).*theta)+q11.*sin((1/2).*t.*theta)).*(q03.* ...
  sin((1/2).*(1+(-1).*t).*theta)+q13.*sin((1/2).*t.*theta))+csc((1/2).* ...
  theta).^2.*(q02.*sin((1/2).*(1+(-1).*t).*theta)+q12.*sin((1/2).*t.* ...
  theta)).*(q04.*sin((1/2).*(1+(-1).*t).*theta)+q14.*sin((1/2).*t.*theta)) ...
  ).^2+4.*((-1).*csc((1/2).*theta).^2.*(q01.*sin((1/2).*(1+(-1).*t).* ...
  theta)+q11.*sin((1/2).*t.*theta)).*(q02.*sin((1/2).*(1+(-1).*t).*theta)+ ...
  q12.*sin((1/2).*t.*theta))+csc((1/2).*theta).^2.*(q03.*sin((1/2).*(1+( ...
  -1).*t).*theta)+q13.*sin((1/2).*t.*theta)).*(q04.*sin((1/2).*(1+(-1).*t) ...
  .*theta)+q14.*sin((1/2).*t.*theta))).^2+(1+(-2).*(csc((1/2).*theta).^2.* ...
  (q02.*sin((1/2).*(1+(-1).*t).*theta)+q12.*sin((1/2).*t.*theta)).^2+csc(( ...
  1/2).*theta).^2.*(q03.*sin((1/2).*(1+(-1).*t).*theta)+q13.*sin((1/2).* ...
  t.*theta)).^2)).^2).^(-1/2)+(-2).*((-1).*((-1/2).*q04.*theta.*cos((1/2) ...
  .*(1+(-1).*t).*theta)+(1/2).*q14.*theta.*cos((1/2).*t.*theta)).*csc(( ...
  1/2).*theta).^2.*(q01.*sin((1/2).*(1+(-1).*t).*theta)+q11.*sin((1/2).* ...
  t.*theta))+((-1/2).*q03.*theta.*cos((1/2).*(1+(-1).*t).*theta)+(1/2).* ...
  q13.*theta.*cos((1/2).*t.*theta)).*csc((1/2).*theta).^2.*(q02.*sin((1/2) ...
  .*(1+(-1).*t).*theta)+q12.*sin((1/2).*t.*theta))+((-1/2).*q02.*theta.* ...
  cos((1/2).*(1+(-1).*t).*theta)+(1/2).*q12.*theta.*cos((1/2).*t.*theta)) ...
  .*csc((1/2).*theta).^2.*(q03.*sin((1/2).*(1+(-1).*t).*theta)+q13.*sin(( ...
  1/2).*t.*theta))+(-1).*((-1/2).*q01.*theta.*cos((1/2).*(1+(-1).*t).* ...
  theta)+(1/2).*q11.*theta.*cos((1/2).*t.*theta)).*csc((1/2).*theta).^2.*( ...
  q04.*sin((1/2).*(1+(-1).*t).*theta)+q14.*sin((1/2).*t.*theta))).*(8.*((( ...
  -1/2).*q03.*theta.*cos((1/2).*(1+(-1).*t).*theta)+(1/2).*q13.*theta.* ...
  cos((1/2).*t.*theta)).*csc((1/2).*theta).^2.*(q01.*sin((1/2).*(1+(-1).* ...
  t).*theta)+q11.*sin((1/2).*t.*theta))+((-1/2).*q04.*theta.*cos((1/2).*( ...
  1+(-1).*t).*theta)+(1/2).*q14.*theta.*cos((1/2).*t.*theta)).*csc((1/2).* ...
  theta).^2.*(q02.*sin((1/2).*(1+(-1).*t).*theta)+q12.*sin((1/2).*t.* ...
  theta))+((-1/2).*q01.*theta.*cos((1/2).*(1+(-1).*t).*theta)+(1/2).*q11.* ...
  theta.*cos((1/2).*t.*theta)).*csc((1/2).*theta).^2.*(q03.*sin((1/2).*(1+ ...
  (-1).*t).*theta)+q13.*sin((1/2).*t.*theta))+((-1/2).*q02.*theta.*cos(( ...
  1/2).*(1+(-1).*t).*theta)+(1/2).*q12.*theta.*cos((1/2).*t.*theta)).*csc( ...
  (1/2).*theta).^2.*(q04.*sin((1/2).*(1+(-1).*t).*theta)+q14.*sin((1/2).* ...
  t.*theta))).*(csc((1/2).*theta).^2.*(q01.*sin((1/2).*(1+(-1).*t).*theta) ...
  +q11.*sin((1/2).*t.*theta)).*(q03.*sin((1/2).*(1+(-1).*t).*theta)+q13.* ...
  sin((1/2).*t.*theta))+csc((1/2).*theta).^2.*(q02.*sin((1/2).*(1+(-1).*t) ...
  .*theta)+q12.*sin((1/2).*t.*theta)).*(q04.*sin((1/2).*(1+(-1).*t).* ...
  theta)+q14.*sin((1/2).*t.*theta)))+8.*((-1).*((-1/2).*q02.*theta.*cos(( ...
  1/2).*(1+(-1).*t).*theta)+(1/2).*q12.*theta.*cos((1/2).*t.*theta)).*csc( ...
  (1/2).*theta).^2.*(q01.*sin((1/2).*(1+(-1).*t).*theta)+q11.*sin((1/2).* ...
  t.*theta))+(-1).*((-1/2).*q01.*theta.*cos((1/2).*(1+(-1).*t).*theta)+( ...
  1/2).*q11.*theta.*cos((1/2).*t.*theta)).*csc((1/2).*theta).^2.*(q02.* ...
  sin((1/2).*(1+(-1).*t).*theta)+q12.*sin((1/2).*t.*theta))+((-1/2).*q04.* ...
  theta.*cos((1/2).*(1+(-1).*t).*theta)+(1/2).*q14.*theta.*cos((1/2).*t.* ...
  theta)).*csc((1/2).*theta).^2.*(q03.*sin((1/2).*(1+(-1).*t).*theta)+ ...
  q13.*sin((1/2).*t.*theta))+((-1/2).*q03.*theta.*cos((1/2).*(1+(-1).*t).* ...
  theta)+(1/2).*q13.*theta.*cos((1/2).*t.*theta)).*csc((1/2).*theta).^2.*( ...
  q04.*sin((1/2).*(1+(-1).*t).*theta)+q14.*sin((1/2).*t.*theta))).*((-1).* ...
  csc((1/2).*theta).^2.*(q01.*sin((1/2).*(1+(-1).*t).*theta)+q11.*sin(( ...
  1/2).*t.*theta)).*(q02.*sin((1/2).*(1+(-1).*t).*theta)+q12.*sin((1/2).* ...
  t.*theta))+csc((1/2).*theta).^2.*(q03.*sin((1/2).*(1+(-1).*t).*theta)+ ...
  q13.*sin((1/2).*t.*theta)).*(q04.*sin((1/2).*(1+(-1).*t).*theta)+q14.* ...
  sin((1/2).*t.*theta)))+(-4).*(2.*((-1/2).*q02.*theta.*cos((1/2).*(1+(-1) ...
  .*t).*theta)+(1/2).*q12.*theta.*cos((1/2).*t.*theta)).*csc((1/2).*theta) ...
  .^2.*(q02.*sin((1/2).*(1+(-1).*t).*theta)+q12.*sin((1/2).*t.*theta))+2.* ...
  ((-1/2).*q03.*theta.*cos((1/2).*(1+(-1).*t).*theta)+(1/2).*q13.*theta.* ...
  cos((1/2).*t.*theta)).*csc((1/2).*theta).^2.*(q03.*sin((1/2).*(1+(-1).* ...
  t).*theta)+q13.*sin((1/2).*t.*theta))).*(1+(-2).*(csc((1/2).*theta).^2.* ...
  (q02.*sin((1/2).*(1+(-1).*t).*theta)+q12.*sin((1/2).*t.*theta)).^2+csc(( ...
  1/2).*theta).^2.*(q03.*sin((1/2).*(1+(-1).*t).*theta)+q13.*sin((1/2).* ...
  t.*theta)).^2))).*(4.*((-1).*csc((1/2).*theta).^2.*(q01.*sin((1/2).*(1+( ...
  -1).*t).*theta)+q11.*sin((1/2).*t.*theta)).*(q02.*sin((1/2).*(1+(-1).*t) ...
  .*theta)+q12.*sin((1/2).*t.*theta))+csc((1/2).*theta).^2.*(q03.*sin(( ...
  1/2).*(1+(-1).*t).*theta)+q13.*sin((1/2).*t.*theta)).*(q04.*sin((1/2).*( ...
  1+(-1).*t).*theta)+q14.*sin((1/2).*t.*theta))).^2+(1+(-2).*(csc((1/2).* ...
  theta).^2.*(q02.*sin((1/2).*(1+(-1).*t).*theta)+q12.*sin((1/2).*t.* ...
  theta)).^2+csc((1/2).*theta).^2.*(q03.*sin((1/2).*(1+(-1).*t).*theta)+ ...
  q13.*sin((1/2).*t.*theta)).^2)).^2).^(-1/2).*(4.*(csc((1/2).*theta).^2.* ...
  (q01.*sin((1/2).*(1+(-1).*t).*theta)+q11.*sin((1/2).*t.*theta)).*(q03.* ...
  sin((1/2).*(1+(-1).*t).*theta)+q13.*sin((1/2).*t.*theta))+csc((1/2).* ...
  theta).^2.*(q02.*sin((1/2).*(1+(-1).*t).*theta)+q12.*sin((1/2).*t.* ...
  theta)).*(q04.*sin((1/2).*(1+(-1).*t).*theta)+q14.*sin((1/2).*t.*theta)) ...
  ).^2+4.*((-1).*csc((1/2).*theta).^2.*(q01.*sin((1/2).*(1+(-1).*t).* ...
  theta)+q11.*sin((1/2).*t.*theta)).*(q02.*sin((1/2).*(1+(-1).*t).*theta)+ ...
  q12.*sin((1/2).*t.*theta))+csc((1/2).*theta).^2.*(q03.*sin((1/2).*(1+( ...
  -1).*t).*theta)+q13.*sin((1/2).*t.*theta)).*(q04.*sin((1/2).*(1+(-1).*t) ...
  .*theta)+q14.*sin((1/2).*t.*theta))).^2+(1+(-2).*(csc((1/2).*theta).^2.* ...
  (q02.*sin((1/2).*(1+(-1).*t).*theta)+q12.*sin((1/2).*t.*theta)).^2+csc(( ...
  1/2).*theta).^2.*(q03.*sin((1/2).*(1+(-1).*t).*theta)+q13.*sin((1/2).* ...
  t.*theta)).^2)).^2).^(-1/2)+(-1).*(csc((1/2).*theta).^2.*(q02.*sin((1/2) ...
  .*(1+(-1).*t).*theta)+q12.*sin((1/2).*t.*theta)).*(q03.*sin((1/2).*(1+( ...
  -1).*t).*theta)+q13.*sin((1/2).*t.*theta))+(-1).*csc((1/2).*theta).^2.*( ...
  q01.*sin((1/2).*(1+(-1).*t).*theta)+q11.*sin((1/2).*t.*theta)).*(q04.* ...
  sin((1/2).*(1+(-1).*t).*theta)+q14.*sin((1/2).*t.*theta))).*(8.*(2.*(( ...
  -1/2).*q02.*theta.*cos((1/2).*(1+(-1).*t).*theta)+(1/2).*q12.*theta.* ...
  cos((1/2).*t.*theta)).*csc((1/2).*theta).^2.*(q02.*sin((1/2).*(1+(-1).* ...
  t).*theta)+q12.*sin((1/2).*t.*theta))+2.*((-1/2).*q03.*theta.*cos((1/2) ...
  .*(1+(-1).*t).*theta)+(1/2).*q13.*theta.*cos((1/2).*t.*theta)).*csc(( ...
  1/2).*theta).^2.*(q03.*sin((1/2).*(1+(-1).*t).*theta)+q13.*sin((1/2).* ...
  t.*theta))).^2+8.*(((-1/2).*q03.*theta.*cos((1/2).*(1+(-1).*t).*theta)+( ...
  1/2).*q13.*theta.*cos((1/2).*t.*theta)).*csc((1/2).*theta).^2.*(q01.* ...
  sin((1/2).*(1+(-1).*t).*theta)+q11.*sin((1/2).*t.*theta))+((-1/2).*q04.* ...
  theta.*cos((1/2).*(1+(-1).*t).*theta)+(1/2).*q14.*theta.*cos((1/2).*t.* ...
  theta)).*csc((1/2).*theta).^2.*(q02.*sin((1/2).*(1+(-1).*t).*theta)+ ...
  q12.*sin((1/2).*t.*theta))+((-1/2).*q01.*theta.*cos((1/2).*(1+(-1).*t).* ...
  theta)+(1/2).*q11.*theta.*cos((1/2).*t.*theta)).*csc((1/2).*theta).^2.*( ...
  q03.*sin((1/2).*(1+(-1).*t).*theta)+q13.*sin((1/2).*t.*theta))+((-1/2).* ...
  q02.*theta.*cos((1/2).*(1+(-1).*t).*theta)+(1/2).*q12.*theta.*cos((1/2) ...
  .*t.*theta)).*csc((1/2).*theta).^2.*(q04.*sin((1/2).*(1+(-1).*t).*theta) ...
  +q14.*sin((1/2).*t.*theta))).^2+8.*((-1).*((-1/2).*q02.*theta.*cos((1/2) ...
  .*(1+(-1).*t).*theta)+(1/2).*q12.*theta.*cos((1/2).*t.*theta)).*csc(( ...
  1/2).*theta).^2.*(q01.*sin((1/2).*(1+(-1).*t).*theta)+q11.*sin((1/2).* ...
  t.*theta))+(-1).*((-1/2).*q01.*theta.*cos((1/2).*(1+(-1).*t).*theta)+( ...
  1/2).*q11.*theta.*cos((1/2).*t.*theta)).*csc((1/2).*theta).^2.*(q02.* ...
  sin((1/2).*(1+(-1).*t).*theta)+q12.*sin((1/2).*t.*theta))+((-1/2).*q04.* ...
  theta.*cos((1/2).*(1+(-1).*t).*theta)+(1/2).*q14.*theta.*cos((1/2).*t.* ...
  theta)).*csc((1/2).*theta).^2.*(q03.*sin((1/2).*(1+(-1).*t).*theta)+ ...
  q13.*sin((1/2).*t.*theta))+((-1/2).*q03.*theta.*cos((1/2).*(1+(-1).*t).* ...
  theta)+(1/2).*q13.*theta.*cos((1/2).*t.*theta)).*csc((1/2).*theta).^2.*( ...
  q04.*sin((1/2).*(1+(-1).*t).*theta)+q14.*sin((1/2).*t.*theta))).^2+8.*( ...
  csc((1/2).*theta).^2.*(q01.*sin((1/2).*(1+(-1).*t).*theta)+q11.*sin(( ...
  1/2).*t.*theta)).*(q03.*sin((1/2).*(1+(-1).*t).*theta)+q13.*sin((1/2).* ...
  t.*theta))+csc((1/2).*theta).^2.*(q02.*sin((1/2).*(1+(-1).*t).*theta)+ ...
  q12.*sin((1/2).*t.*theta)).*(q04.*sin((1/2).*(1+(-1).*t).*theta)+q14.* ...
  sin((1/2).*t.*theta))).*(2.*((-1/2).*q01.*theta.*cos((1/2).*(1+(-1).*t) ...
  .*theta)+(1/2).*q11.*theta.*cos((1/2).*t.*theta)).*((-1/2).*q03.*theta.* ...
  cos((1/2).*(1+(-1).*t).*theta)+(1/2).*q13.*theta.*cos((1/2).*t.*theta)) ...
  .*csc((1/2).*theta).^2+2.*((-1/2).*q02.*theta.*cos((1/2).*(1+(-1).*t).* ...
  theta)+(1/2).*q12.*theta.*cos((1/2).*t.*theta)).*((-1/2).*q04.*theta.* ...
  cos((1/2).*(1+(-1).*t).*theta)+(1/2).*q14.*theta.*cos((1/2).*t.*theta)) ...
  .*csc((1/2).*theta).^2+csc((1/2).*theta).^2.*(q03.*sin((1/2).*(1+(-1).* ...
  t).*theta)+q13.*sin((1/2).*t.*theta)).*((-1/4).*q01.*theta.^2.*sin((1/2) ...
  .*(1+(-1).*t).*theta)+(-1/4).*q11.*theta.^2.*sin((1/2).*t.*theta))+csc(( ...
  1/2).*theta).^2.*(q04.*sin((1/2).*(1+(-1).*t).*theta)+q14.*sin((1/2).* ...
  t.*theta)).*((-1/4).*q02.*theta.^2.*sin((1/2).*(1+(-1).*t).*theta)+( ...
  -1/4).*q12.*theta.^2.*sin((1/2).*t.*theta))+csc((1/2).*theta).^2.*(q01.* ...
  sin((1/2).*(1+(-1).*t).*theta)+q11.*sin((1/2).*t.*theta)).*((-1/4).* ...
  q03.*theta.^2.*sin((1/2).*(1+(-1).*t).*theta)+(-1/4).*q13.*theta.^2.* ...
  sin((1/2).*t.*theta))+csc((1/2).*theta).^2.*(q02.*sin((1/2).*(1+(-1).*t) ...
  .*theta)+q12.*sin((1/2).*t.*theta)).*((-1/4).*q04.*theta.^2.*sin((1/2).* ...
  (1+(-1).*t).*theta)+(-1/4).*q14.*theta.^2.*sin((1/2).*t.*theta)))+8.*(( ...
  -1).*csc((1/2).*theta).^2.*(q01.*sin((1/2).*(1+(-1).*t).*theta)+q11.* ...
  sin((1/2).*t.*theta)).*(q02.*sin((1/2).*(1+(-1).*t).*theta)+q12.*sin(( ...
  1/2).*t.*theta))+csc((1/2).*theta).^2.*(q03.*sin((1/2).*(1+(-1).*t).* ...
  theta)+q13.*sin((1/2).*t.*theta)).*(q04.*sin((1/2).*(1+(-1).*t).*theta)+ ...
  q14.*sin((1/2).*t.*theta))).*((-2).*((-1/2).*q01.*theta.*cos((1/2).*(1+( ...
  -1).*t).*theta)+(1/2).*q11.*theta.*cos((1/2).*t.*theta)).*((-1/2).*q02.* ...
  theta.*cos((1/2).*(1+(-1).*t).*theta)+(1/2).*q12.*theta.*cos((1/2).*t.* ...
  theta)).*csc((1/2).*theta).^2+2.*((-1/2).*q03.*theta.*cos((1/2).*(1+(-1) ...
  .*t).*theta)+(1/2).*q13.*theta.*cos((1/2).*t.*theta)).*((-1/2).*q04.* ...
  theta.*cos((1/2).*(1+(-1).*t).*theta)+(1/2).*q14.*theta.*cos((1/2).*t.* ...
  theta)).*csc((1/2).*theta).^2+(-1).*csc((1/2).*theta).^2.*(q02.*sin(( ...
  1/2).*(1+(-1).*t).*theta)+q12.*sin((1/2).*t.*theta)).*((-1/4).*q01.* ...
  theta.^2.*sin((1/2).*(1+(-1).*t).*theta)+(-1/4).*q11.*theta.^2.*sin(( ...
  1/2).*t.*theta))+(-1).*csc((1/2).*theta).^2.*(q01.*sin((1/2).*(1+(-1).* ...
  t).*theta)+q11.*sin((1/2).*t.*theta)).*((-1/4).*q02.*theta.^2.*sin((1/2) ...
  .*(1+(-1).*t).*theta)+(-1/4).*q12.*theta.^2.*sin((1/2).*t.*theta))+csc(( ...
  1/2).*theta).^2.*(q04.*sin((1/2).*(1+(-1).*t).*theta)+q14.*sin((1/2).* ...
  t.*theta)).*((-1/4).*q03.*theta.^2.*sin((1/2).*(1+(-1).*t).*theta)+( ...
  -1/4).*q13.*theta.^2.*sin((1/2).*t.*theta))+csc((1/2).*theta).^2.*(q03.* ...
  sin((1/2).*(1+(-1).*t).*theta)+q13.*sin((1/2).*t.*theta)).*((-1/4).* ...
  q04.*theta.^2.*sin((1/2).*(1+(-1).*t).*theta)+(-1/4).*q14.*theta.^2.* ...
  sin((1/2).*t.*theta)))+(-4).*(2.*((-1/2).*q02.*theta.*cos((1/2).*(1+(-1) ...
  .*t).*theta)+(1/2).*q12.*theta.*cos((1/2).*t.*theta)).^2.*csc((1/2).* ...
  theta).^2+2.*((-1/2).*q03.*theta.*cos((1/2).*(1+(-1).*t).*theta)+(1/2).* ...
  q13.*theta.*cos((1/2).*t.*theta)).^2.*csc((1/2).*theta).^2+2.*csc((1/2) ...
  .*theta).^2.*(q02.*sin((1/2).*(1+(-1).*t).*theta)+q12.*sin((1/2).*t.* ...
  theta)).*((-1/4).*q02.*theta.^2.*sin((1/2).*(1+(-1).*t).*theta)+(-1/4).* ...
  q12.*theta.^2.*sin((1/2).*t.*theta))+2.*csc((1/2).*theta).^2.*(q03.*sin( ...
  (1/2).*(1+(-1).*t).*theta)+q13.*sin((1/2).*t.*theta)).*((-1/4).*q03.* ...
  theta.^2.*sin((1/2).*(1+(-1).*t).*theta)+(-1/4).*q13.*theta.^2.*sin(( ...
  1/2).*t.*theta))).*(1+(-2).*(csc((1/2).*theta).^2.*(q02.*sin((1/2).*(1+( ...
  -1).*t).*theta)+q12.*sin((1/2).*t.*theta)).^2+csc((1/2).*theta).^2.*( ...
  q03.*sin((1/2).*(1+(-1).*t).*theta)+q13.*sin((1/2).*t.*theta)).^2))).*( ...
  4.*((-1).*csc((1/2).*theta).^2.*(q01.*sin((1/2).*(1+(-1).*t).*theta)+ ...
  q11.*sin((1/2).*t.*theta)).*(q02.*sin((1/2).*(1+(-1).*t).*theta)+q12.* ...
  sin((1/2).*t.*theta))+csc((1/2).*theta).^2.*(q03.*sin((1/2).*(1+(-1).*t) ...
  .*theta)+q13.*sin((1/2).*t.*theta)).*(q04.*sin((1/2).*(1+(-1).*t).* ...
  theta)+q14.*sin((1/2).*t.*theta))).^2+(1+(-2).*(csc((1/2).*theta).^2.*( ...
  q02.*sin((1/2).*(1+(-1).*t).*theta)+q12.*sin((1/2).*t.*theta)).^2+csc(( ...
  1/2).*theta).^2.*(q03.*sin((1/2).*(1+(-1).*t).*theta)+q13.*sin((1/2).* ...
  t.*theta)).^2)).^2).^(-1/2).*(4.*(csc((1/2).*theta).^2.*(q01.*sin((1/2) ...
  .*(1+(-1).*t).*theta)+q11.*sin((1/2).*t.*theta)).*(q03.*sin((1/2).*(1+( ...
  -1).*t).*theta)+q13.*sin((1/2).*t.*theta))+csc((1/2).*theta).^2.*(q02.* ...
  sin((1/2).*(1+(-1).*t).*theta)+q12.*sin((1/2).*t.*theta)).*(q04.*sin(( ...
  1/2).*(1+(-1).*t).*theta)+q14.*sin((1/2).*t.*theta))).^2+4.*((-1).*csc(( ...
  1/2).*theta).^2.*(q01.*sin((1/2).*(1+(-1).*t).*theta)+q11.*sin((1/2).* ...
  t.*theta)).*(q02.*sin((1/2).*(1+(-1).*t).*theta)+q12.*sin((1/2).*t.* ...
  theta))+csc((1/2).*theta).^2.*(q03.*sin((1/2).*(1+(-1).*t).*theta)+q13.* ...
  sin((1/2).*t.*theta)).*(q04.*sin((1/2).*(1+(-1).*t).*theta)+q14.*sin(( ...
  1/2).*t.*theta))).^2+(1+(-2).*(csc((1/2).*theta).^2.*(q02.*sin((1/2).*( ...
  1+(-1).*t).*theta)+q12.*sin((1/2).*t.*theta)).^2+csc((1/2).*theta).^2.*( ...
  q03.*sin((1/2).*(1+(-1).*t).*theta)+q13.*sin((1/2).*t.*theta)).^2)).^2) ...
  .^(-1/2)+(-3/2).*(csc((1/2).*theta).^2.*(q02.*sin((1/2).*(1+(-1).*t).* ...
  theta)+q12.*sin((1/2).*t.*theta)).*(q03.*sin((1/2).*(1+(-1).*t).*theta)+ ...
  q13.*sin((1/2).*t.*theta))+(-1).*csc((1/2).*theta).^2.*(q01.*sin((1/2).* ...
  (1+(-1).*t).*theta)+q11.*sin((1/2).*t.*theta)).*(q04.*sin((1/2).*(1+(-1) ...
  .*t).*theta)+q14.*sin((1/2).*t.*theta))).*(8.*((-1).*((-1/2).*q02.* ...
  theta.*cos((1/2).*(1+(-1).*t).*theta)+(1/2).*q12.*theta.*cos((1/2).*t.* ...
  theta)).*csc((1/2).*theta).^2.*(q01.*sin((1/2).*(1+(-1).*t).*theta)+ ...
  q11.*sin((1/2).*t.*theta))+(-1).*((-1/2).*q01.*theta.*cos((1/2).*(1+(-1) ...
  .*t).*theta)+(1/2).*q11.*theta.*cos((1/2).*t.*theta)).*csc((1/2).*theta) ...
  .^2.*(q02.*sin((1/2).*(1+(-1).*t).*theta)+q12.*sin((1/2).*t.*theta))+(( ...
  -1/2).*q04.*theta.*cos((1/2).*(1+(-1).*t).*theta)+(1/2).*q14.*theta.* ...
  cos((1/2).*t.*theta)).*csc((1/2).*theta).^2.*(q03.*sin((1/2).*(1+(-1).* ...
  t).*theta)+q13.*sin((1/2).*t.*theta))+((-1/2).*q03.*theta.*cos((1/2).*( ...
  1+(-1).*t).*theta)+(1/2).*q13.*theta.*cos((1/2).*t.*theta)).*csc((1/2).* ...
  theta).^2.*(q04.*sin((1/2).*(1+(-1).*t).*theta)+q14.*sin((1/2).*t.* ...
  theta))).*((-1).*csc((1/2).*theta).^2.*(q01.*sin((1/2).*(1+(-1).*t).* ...
  theta)+q11.*sin((1/2).*t.*theta)).*(q02.*sin((1/2).*(1+(-1).*t).*theta)+ ...
  q12.*sin((1/2).*t.*theta))+csc((1/2).*theta).^2.*(q03.*sin((1/2).*(1+( ...
  -1).*t).*theta)+q13.*sin((1/2).*t.*theta)).*(q04.*sin((1/2).*(1+(-1).*t) ...
  .*theta)+q14.*sin((1/2).*t.*theta)))+(-4).*(2.*((-1/2).*q02.*theta.*cos( ...
  (1/2).*(1+(-1).*t).*theta)+(1/2).*q12.*theta.*cos((1/2).*t.*theta)).* ...
  csc((1/2).*theta).^2.*(q02.*sin((1/2).*(1+(-1).*t).*theta)+q12.*sin(( ...
  1/2).*t.*theta))+2.*((-1/2).*q03.*theta.*cos((1/2).*(1+(-1).*t).*theta)+ ...
  (1/2).*q13.*theta.*cos((1/2).*t.*theta)).*csc((1/2).*theta).^2.*(q03.* ...
  sin((1/2).*(1+(-1).*t).*theta)+q13.*sin((1/2).*t.*theta))).*(1+(-2).*( ...
  csc((1/2).*theta).^2.*(q02.*sin((1/2).*(1+(-1).*t).*theta)+q12.*sin(( ...
  1/2).*t.*theta)).^2+csc((1/2).*theta).^2.*(q03.*sin((1/2).*(1+(-1).*t).* ...
  theta)+q13.*sin((1/2).*t.*theta)).^2))).^2.*(4.*((-1).*csc((1/2).*theta) ...
  .^2.*(q01.*sin((1/2).*(1+(-1).*t).*theta)+q11.*sin((1/2).*t.*theta)).*( ...
  q02.*sin((1/2).*(1+(-1).*t).*theta)+q12.*sin((1/2).*t.*theta))+csc((1/2) ...
  .*theta).^2.*(q03.*sin((1/2).*(1+(-1).*t).*theta)+q13.*sin((1/2).*t.* ...
  theta)).*(q04.*sin((1/2).*(1+(-1).*t).*theta)+q14.*sin((1/2).*t.*theta)) ...
  ).^2+(1+(-2).*(csc((1/2).*theta).^2.*(q02.*sin((1/2).*(1+(-1).*t).* ...
  theta)+q12.*sin((1/2).*t.*theta)).^2+csc((1/2).*theta).^2.*(q03.*sin(( ...
  1/2).*(1+(-1).*t).*theta)+q13.*sin((1/2).*t.*theta)).^2)).^2).^(-5/2).*( ...
  4.*(csc((1/2).*theta).^2.*(q01.*sin((1/2).*(1+(-1).*t).*theta)+q11.*sin( ...
  (1/2).*t.*theta)).*(q03.*sin((1/2).*(1+(-1).*t).*theta)+q13.*sin((1/2).* ...
  t.*theta))+csc((1/2).*theta).^2.*(q02.*sin((1/2).*(1+(-1).*t).*theta)+ ...
  q12.*sin((1/2).*t.*theta)).*(q04.*sin((1/2).*(1+(-1).*t).*theta)+q14.* ...
  sin((1/2).*t.*theta))).^2+4.*((-1).*csc((1/2).*theta).^2.*(q01.*sin(( ...
  1/2).*(1+(-1).*t).*theta)+q11.*sin((1/2).*t.*theta)).*(q02.*sin((1/2).*( ...
  1+(-1).*t).*theta)+q12.*sin((1/2).*t.*theta))+csc((1/2).*theta).^2.*( ...
  q03.*sin((1/2).*(1+(-1).*t).*theta)+q13.*sin((1/2).*t.*theta)).*(q04.* ...
  sin((1/2).*(1+(-1).*t).*theta)+q14.*sin((1/2).*t.*theta))).^2+(1+(-2).*( ...
  csc((1/2).*theta).^2.*(q02.*sin((1/2).*(1+(-1).*t).*theta)+q12.*sin(( ...
  1/2).*t.*theta)).^2+csc((1/2).*theta).^2.*(q03.*sin((1/2).*(1+(-1).*t).* ...
  theta)+q13.*sin((1/2).*t.*theta)).^2)).^2).^(1/2)+2.*((-1).*((-1/2).* ...
  q04.*theta.*cos((1/2).*(1+(-1).*t).*theta)+(1/2).*q14.*theta.*cos((1/2) ...
  .*t.*theta)).*csc((1/2).*theta).^2.*(q01.*sin((1/2).*(1+(-1).*t).*theta) ...
  +q11.*sin((1/2).*t.*theta))+((-1/2).*q03.*theta.*cos((1/2).*(1+(-1).*t) ...
  .*theta)+(1/2).*q13.*theta.*cos((1/2).*t.*theta)).*csc((1/2).*theta) ...
  .^2.*(q02.*sin((1/2).*(1+(-1).*t).*theta)+q12.*sin((1/2).*t.*theta))+(( ...
  -1/2).*q02.*theta.*cos((1/2).*(1+(-1).*t).*theta)+(1/2).*q12.*theta.* ...
  cos((1/2).*t.*theta)).*csc((1/2).*theta).^2.*(q03.*sin((1/2).*(1+(-1).* ...
  t).*theta)+q13.*sin((1/2).*t.*theta))+(-1).*((-1/2).*q01.*theta.*cos(( ...
  1/2).*(1+(-1).*t).*theta)+(1/2).*q11.*theta.*cos((1/2).*t.*theta)).*csc( ...
  (1/2).*theta).^2.*(q04.*sin((1/2).*(1+(-1).*t).*theta)+q14.*sin((1/2).* ...
  t.*theta))).*(8.*((-1).*((-1/2).*q02.*theta.*cos((1/2).*(1+(-1).*t).* ...
  theta)+(1/2).*q12.*theta.*cos((1/2).*t.*theta)).*csc((1/2).*theta).^2.*( ...
  q01.*sin((1/2).*(1+(-1).*t).*theta)+q11.*sin((1/2).*t.*theta))+(-1).*(( ...
  -1/2).*q01.*theta.*cos((1/2).*(1+(-1).*t).*theta)+(1/2).*q11.*theta.* ...
  cos((1/2).*t.*theta)).*csc((1/2).*theta).^2.*(q02.*sin((1/2).*(1+(-1).* ...
  t).*theta)+q12.*sin((1/2).*t.*theta))+((-1/2).*q04.*theta.*cos((1/2).*( ...
  1+(-1).*t).*theta)+(1/2).*q14.*theta.*cos((1/2).*t.*theta)).*csc((1/2).* ...
  theta).^2.*(q03.*sin((1/2).*(1+(-1).*t).*theta)+q13.*sin((1/2).*t.* ...
  theta))+((-1/2).*q03.*theta.*cos((1/2).*(1+(-1).*t).*theta)+(1/2).*q13.* ...
  theta.*cos((1/2).*t.*theta)).*csc((1/2).*theta).^2.*(q04.*sin((1/2).*(1+ ...
  (-1).*t).*theta)+q14.*sin((1/2).*t.*theta))).*((-1).*csc((1/2).*theta) ...
  .^2.*(q01.*sin((1/2).*(1+(-1).*t).*theta)+q11.*sin((1/2).*t.*theta)).*( ...
  q02.*sin((1/2).*(1+(-1).*t).*theta)+q12.*sin((1/2).*t.*theta))+csc((1/2) ...
  .*theta).^2.*(q03.*sin((1/2).*(1+(-1).*t).*theta)+q13.*sin((1/2).*t.* ...
  theta)).*(q04.*sin((1/2).*(1+(-1).*t).*theta)+q14.*sin((1/2).*t.*theta)) ...
  )+(-4).*(2.*((-1/2).*q02.*theta.*cos((1/2).*(1+(-1).*t).*theta)+(1/2).* ...
  q12.*theta.*cos((1/2).*t.*theta)).*csc((1/2).*theta).^2.*(q02.*sin((1/2) ...
  .*(1+(-1).*t).*theta)+q12.*sin((1/2).*t.*theta))+2.*((-1/2).*q03.* ...
  theta.*cos((1/2).*(1+(-1).*t).*theta)+(1/2).*q13.*theta.*cos((1/2).*t.* ...
  theta)).*csc((1/2).*theta).^2.*(q03.*sin((1/2).*(1+(-1).*t).*theta)+ ...
  q13.*sin((1/2).*t.*theta))).*(1+(-2).*(csc((1/2).*theta).^2.*(q02.*sin(( ...
  1/2).*(1+(-1).*t).*theta)+q12.*sin((1/2).*t.*theta)).^2+csc((1/2).* ...
  theta).^2.*(q03.*sin((1/2).*(1+(-1).*t).*theta)+q13.*sin((1/2).*t.* ...
  theta)).^2))).*(4.*((-1).*csc((1/2).*theta).^2.*(q01.*sin((1/2).*(1+(-1) ...
  .*t).*theta)+q11.*sin((1/2).*t.*theta)).*(q02.*sin((1/2).*(1+(-1).*t).* ...
  theta)+q12.*sin((1/2).*t.*theta))+csc((1/2).*theta).^2.*(q03.*sin((1/2) ...
  .*(1+(-1).*t).*theta)+q13.*sin((1/2).*t.*theta)).*(q04.*sin((1/2).*(1+( ...
  -1).*t).*theta)+q14.*sin((1/2).*t.*theta))).^2+(1+(-2).*(csc((1/2).* ...
  theta).^2.*(q02.*sin((1/2).*(1+(-1).*t).*theta)+q12.*sin((1/2).*t.* ...
  theta)).^2+csc((1/2).*theta).^2.*(q03.*sin((1/2).*(1+(-1).*t).*theta)+ ...
  q13.*sin((1/2).*t.*theta)).^2)).^2).^(-3/2).*(4.*(csc((1/2).*theta).^2.* ...
  (q01.*sin((1/2).*(1+(-1).*t).*theta)+q11.*sin((1/2).*t.*theta)).*(q03.* ...
  sin((1/2).*(1+(-1).*t).*theta)+q13.*sin((1/2).*t.*theta))+csc((1/2).* ...
  theta).^2.*(q02.*sin((1/2).*(1+(-1).*t).*theta)+q12.*sin((1/2).*t.* ...
  theta)).*(q04.*sin((1/2).*(1+(-1).*t).*theta)+q14.*sin((1/2).*t.*theta)) ...
  ).^2+4.*((-1).*csc((1/2).*theta).^2.*(q01.*sin((1/2).*(1+(-1).*t).* ...
  theta)+q11.*sin((1/2).*t.*theta)).*(q02.*sin((1/2).*(1+(-1).*t).*theta)+ ...
  q12.*sin((1/2).*t.*theta))+csc((1/2).*theta).^2.*(q03.*sin((1/2).*(1+( ...
  -1).*t).*theta)+q13.*sin((1/2).*t.*theta)).*(q04.*sin((1/2).*(1+(-1).*t) ...
  .*theta)+q14.*sin((1/2).*t.*theta))).^2+(1+(-2).*(csc((1/2).*theta).^2.* ...
  (q02.*sin((1/2).*(1+(-1).*t).*theta)+q12.*sin((1/2).*t.*theta)).^2+csc(( ...
  1/2).*theta).^2.*(q03.*sin((1/2).*(1+(-1).*t).*theta)+q13.*sin((1/2).* ...
  t.*theta)).^2)).^2).^(1/2)+(csc((1/2).*theta).^2.*(q02.*sin((1/2).*(1+( ...
  -1).*t).*theta)+q12.*sin((1/2).*t.*theta)).*(q03.*sin((1/2).*(1+(-1).*t) ...
  .*theta)+q13.*sin((1/2).*t.*theta))+(-1).*csc((1/2).*theta).^2.*(q01.* ...
  sin((1/2).*(1+(-1).*t).*theta)+q11.*sin((1/2).*t.*theta)).*(q04.*sin(( ...
  1/2).*(1+(-1).*t).*theta)+q14.*sin((1/2).*t.*theta))).*(8.*(2.*((-1/2).* ...
  q02.*theta.*cos((1/2).*(1+(-1).*t).*theta)+(1/2).*q12.*theta.*cos((1/2) ...
  .*t.*theta)).*csc((1/2).*theta).^2.*(q02.*sin((1/2).*(1+(-1).*t).*theta) ...
  +q12.*sin((1/2).*t.*theta))+2.*((-1/2).*q03.*theta.*cos((1/2).*(1+(-1).* ...
  t).*theta)+(1/2).*q13.*theta.*cos((1/2).*t.*theta)).*csc((1/2).*theta) ...
  .^2.*(q03.*sin((1/2).*(1+(-1).*t).*theta)+q13.*sin((1/2).*t.*theta))) ...
  .^2+8.*((-1).*((-1/2).*q02.*theta.*cos((1/2).*(1+(-1).*t).*theta)+(1/2) ...
  .*q12.*theta.*cos((1/2).*t.*theta)).*csc((1/2).*theta).^2.*(q01.*sin(( ...
  1/2).*(1+(-1).*t).*theta)+q11.*sin((1/2).*t.*theta))+(-1).*((-1/2).* ...
  q01.*theta.*cos((1/2).*(1+(-1).*t).*theta)+(1/2).*q11.*theta.*cos((1/2) ...
  .*t.*theta)).*csc((1/2).*theta).^2.*(q02.*sin((1/2).*(1+(-1).*t).*theta) ...
  +q12.*sin((1/2).*t.*theta))+((-1/2).*q04.*theta.*cos((1/2).*(1+(-1).*t) ...
  .*theta)+(1/2).*q14.*theta.*cos((1/2).*t.*theta)).*csc((1/2).*theta) ...
  .^2.*(q03.*sin((1/2).*(1+(-1).*t).*theta)+q13.*sin((1/2).*t.*theta))+(( ...
  -1/2).*q03.*theta.*cos((1/2).*(1+(-1).*t).*theta)+(1/2).*q13.*theta.* ...
  cos((1/2).*t.*theta)).*csc((1/2).*theta).^2.*(q04.*sin((1/2).*(1+(-1).* ...
  t).*theta)+q14.*sin((1/2).*t.*theta))).^2+8.*((-1).*csc((1/2).*theta) ...
  .^2.*(q01.*sin((1/2).*(1+(-1).*t).*theta)+q11.*sin((1/2).*t.*theta)).*( ...
  q02.*sin((1/2).*(1+(-1).*t).*theta)+q12.*sin((1/2).*t.*theta))+csc((1/2) ...
  .*theta).^2.*(q03.*sin((1/2).*(1+(-1).*t).*theta)+q13.*sin((1/2).*t.* ...
  theta)).*(q04.*sin((1/2).*(1+(-1).*t).*theta)+q14.*sin((1/2).*t.*theta)) ...
  ).*((-2).*((-1/2).*q01.*theta.*cos((1/2).*(1+(-1).*t).*theta)+(1/2).* ...
  q11.*theta.*cos((1/2).*t.*theta)).*((-1/2).*q02.*theta.*cos((1/2).*(1+( ...
  -1).*t).*theta)+(1/2).*q12.*theta.*cos((1/2).*t.*theta)).*csc((1/2).* ...
  theta).^2+2.*((-1/2).*q03.*theta.*cos((1/2).*(1+(-1).*t).*theta)+(1/2).* ...
  q13.*theta.*cos((1/2).*t.*theta)).*((-1/2).*q04.*theta.*cos((1/2).*(1+( ...
  -1).*t).*theta)+(1/2).*q14.*theta.*cos((1/2).*t.*theta)).*csc((1/2).* ...
  theta).^2+(-1).*csc((1/2).*theta).^2.*(q02.*sin((1/2).*(1+(-1).*t).* ...
  theta)+q12.*sin((1/2).*t.*theta)).*((-1/4).*q01.*theta.^2.*sin((1/2).*( ...
  1+(-1).*t).*theta)+(-1/4).*q11.*theta.^2.*sin((1/2).*t.*theta))+(-1).* ...
  csc((1/2).*theta).^2.*(q01.*sin((1/2).*(1+(-1).*t).*theta)+q11.*sin(( ...
  1/2).*t.*theta)).*((-1/4).*q02.*theta.^2.*sin((1/2).*(1+(-1).*t).*theta) ...
  +(-1/4).*q12.*theta.^2.*sin((1/2).*t.*theta))+csc((1/2).*theta).^2.*( ...
  q04.*sin((1/2).*(1+(-1).*t).*theta)+q14.*sin((1/2).*t.*theta)).*((-1/4) ...
  .*q03.*theta.^2.*sin((1/2).*(1+(-1).*t).*theta)+(-1/4).*q13.*theta.^2.* ...
  sin((1/2).*t.*theta))+csc((1/2).*theta).^2.*(q03.*sin((1/2).*(1+(-1).*t) ...
  .*theta)+q13.*sin((1/2).*t.*theta)).*((-1/4).*q04.*theta.^2.*sin((1/2).* ...
  (1+(-1).*t).*theta)+(-1/4).*q14.*theta.^2.*sin((1/2).*t.*theta)))+(-4).* ...
  (2.*((-1/2).*q02.*theta.*cos((1/2).*(1+(-1).*t).*theta)+(1/2).*q12.* ...
  theta.*cos((1/2).*t.*theta)).^2.*csc((1/2).*theta).^2+2.*((-1/2).*q03.* ...
  theta.*cos((1/2).*(1+(-1).*t).*theta)+(1/2).*q13.*theta.*cos((1/2).*t.* ...
  theta)).^2.*csc((1/2).*theta).^2+2.*csc((1/2).*theta).^2.*(q02.*sin(( ...
  1/2).*(1+(-1).*t).*theta)+q12.*sin((1/2).*t.*theta)).*((-1/4).*q02.* ...
  theta.^2.*sin((1/2).*(1+(-1).*t).*theta)+(-1/4).*q12.*theta.^2.*sin(( ...
  1/2).*t.*theta))+2.*csc((1/2).*theta).^2.*(q03.*sin((1/2).*(1+(-1).*t).* ...
  theta)+q13.*sin((1/2).*t.*theta)).*((-1/4).*q03.*theta.^2.*sin((1/2).*( ...
  1+(-1).*t).*theta)+(-1/4).*q13.*theta.^2.*sin((1/2).*t.*theta))).*(1+( ...
  -2).*(csc((1/2).*theta).^2.*(q02.*sin((1/2).*(1+(-1).*t).*theta)+q12.* ...
  sin((1/2).*t.*theta)).^2+csc((1/2).*theta).^2.*(q03.*sin((1/2).*(1+(-1) ...
  .*t).*theta)+q13.*sin((1/2).*t.*theta)).^2))).*(4.*((-1).*csc((1/2).* ...
  theta).^2.*(q01.*sin((1/2).*(1+(-1).*t).*theta)+q11.*sin((1/2).*t.* ...
  theta)).*(q02.*sin((1/2).*(1+(-1).*t).*theta)+q12.*sin((1/2).*t.*theta)) ...
  +csc((1/2).*theta).^2.*(q03.*sin((1/2).*(1+(-1).*t).*theta)+q13.*sin(( ...
  1/2).*t.*theta)).*(q04.*sin((1/2).*(1+(-1).*t).*theta)+q14.*sin((1/2).* ...
  t.*theta))).^2+(1+(-2).*(csc((1/2).*theta).^2.*(q02.*sin((1/2).*(1+(-1) ...
  .*t).*theta)+q12.*sin((1/2).*t.*theta)).^2+csc((1/2).*theta).^2.*(q03.* ...
  sin((1/2).*(1+(-1).*t).*theta)+q13.*sin((1/2).*t.*theta)).^2)).^2).^( ...
  -3/2).*(4.*(csc((1/2).*theta).^2.*(q01.*sin((1/2).*(1+(-1).*t).*theta)+ ...
  q11.*sin((1/2).*t.*theta)).*(q03.*sin((1/2).*(1+(-1).*t).*theta)+q13.* ...
  sin((1/2).*t.*theta))+csc((1/2).*theta).^2.*(q02.*sin((1/2).*(1+(-1).*t) ...
  .*theta)+q12.*sin((1/2).*t.*theta)).*(q04.*sin((1/2).*(1+(-1).*t).* ...
  theta)+q14.*sin((1/2).*t.*theta))).^2+4.*((-1).*csc((1/2).*theta).^2.*( ...
  q01.*sin((1/2).*(1+(-1).*t).*theta)+q11.*sin((1/2).*t.*theta)).*(q02.* ...
  sin((1/2).*(1+(-1).*t).*theta)+q12.*sin((1/2).*t.*theta))+csc((1/2).* ...
  theta).^2.*(q03.*sin((1/2).*(1+(-1).*t).*theta)+q13.*sin((1/2).*t.* ...
  theta)).*(q04.*sin((1/2).*(1+(-1).*t).*theta)+q14.*sin((1/2).*t.*theta)) ...
  ).^2+(1+(-2).*(csc((1/2).*theta).^2.*(q02.*sin((1/2).*(1+(-1).*t).* ...
  theta)+q12.*sin((1/2).*t.*theta)).^2+csc((1/2).*theta).^2.*(q03.*sin(( ...
  1/2).*(1+(-1).*t).*theta)+q13.*sin((1/2).*t.*theta)).^2)).^2).^(1/2)+( ...
  -2).*(2.*((-1/2).*q02.*theta.*cos((1/2).*(1+(-1).*t).*theta)+(1/2).* ...
  q12.*theta.*cos((1/2).*t.*theta)).*((-1/2).*q03.*theta.*cos((1/2).*(1+( ...
  -1).*t).*theta)+(1/2).*q13.*theta.*cos((1/2).*t.*theta)).*csc((1/2).* ...
  theta).^2+(-2).*((-1/2).*q01.*theta.*cos((1/2).*(1+(-1).*t).*theta)+( ...
  1/2).*q11.*theta.*cos((1/2).*t.*theta)).*((-1/2).*q04.*theta.*cos((1/2) ...
  .*(1+(-1).*t).*theta)+(1/2).*q14.*theta.*cos((1/2).*t.*theta)).*csc(( ...
  1/2).*theta).^2+(-1).*csc((1/2).*theta).^2.*(q04.*sin((1/2).*(1+(-1).*t) ...
  .*theta)+q14.*sin((1/2).*t.*theta)).*((-1/4).*q01.*theta.^2.*sin((1/2).* ...
  (1+(-1).*t).*theta)+(-1/4).*q11.*theta.^2.*sin((1/2).*t.*theta))+csc(( ...
  1/2).*theta).^2.*(q03.*sin((1/2).*(1+(-1).*t).*theta)+q13.*sin((1/2).* ...
  t.*theta)).*((-1/4).*q02.*theta.^2.*sin((1/2).*(1+(-1).*t).*theta)+( ...
  -1/4).*q12.*theta.^2.*sin((1/2).*t.*theta))+csc((1/2).*theta).^2.*(q02.* ...
  sin((1/2).*(1+(-1).*t).*theta)+q12.*sin((1/2).*t.*theta)).*((-1/4).* ...
  q03.*theta.^2.*sin((1/2).*(1+(-1).*t).*theta)+(-1/4).*q13.*theta.^2.* ...
  sin((1/2).*t.*theta))+(-1).*csc((1/2).*theta).^2.*(q01.*sin((1/2).*(1+( ...
  -1).*t).*theta)+q11.*sin((1/2).*t.*theta)).*((-1/4).*q04.*theta.^2.*sin( ...
  (1/2).*(1+(-1).*t).*theta)+(-1/4).*q14.*theta.^2.*sin((1/2).*t.*theta))) ...
  .*(4.*((-1).*csc((1/2).*theta).^2.*(q01.*sin((1/2).*(1+(-1).*t).*theta)+ ...
  q11.*sin((1/2).*t.*theta)).*(q02.*sin((1/2).*(1+(-1).*t).*theta)+q12.* ...
  sin((1/2).*t.*theta))+csc((1/2).*theta).^2.*(q03.*sin((1/2).*(1+(-1).*t) ...
  .*theta)+q13.*sin((1/2).*t.*theta)).*(q04.*sin((1/2).*(1+(-1).*t).* ...
  theta)+q14.*sin((1/2).*t.*theta))).^2+(1+(-2).*(csc((1/2).*theta).^2.*( ...
  q02.*sin((1/2).*(1+(-1).*t).*theta)+q12.*sin((1/2).*t.*theta)).^2+csc(( ...
  1/2).*theta).^2.*(q03.*sin((1/2).*(1+(-1).*t).*theta)+q13.*sin((1/2).* ...
  t.*theta)).^2)).^2).^(-1/2).*(4.*(csc((1/2).*theta).^2.*(q01.*sin((1/2) ...
  .*(1+(-1).*t).*theta)+q11.*sin((1/2).*t.*theta)).*(q03.*sin((1/2).*(1+( ...
  -1).*t).*theta)+q13.*sin((1/2).*t.*theta))+csc((1/2).*theta).^2.*(q02.* ...
  sin((1/2).*(1+(-1).*t).*theta)+q12.*sin((1/2).*t.*theta)).*(q04.*sin(( ...
  1/2).*(1+(-1).*t).*theta)+q14.*sin((1/2).*t.*theta))).^2+4.*((-1).*csc(( ...
  1/2).*theta).^2.*(q01.*sin((1/2).*(1+(-1).*t).*theta)+q11.*sin((1/2).* ...
  t.*theta)).*(q02.*sin((1/2).*(1+(-1).*t).*theta)+q12.*sin((1/2).*t.* ...
  theta))+csc((1/2).*theta).^2.*(q03.*sin((1/2).*(1+(-1).*t).*theta)+q13.* ...
  sin((1/2).*t.*theta)).*(q04.*sin((1/2).*(1+(-1).*t).*theta)+q14.*sin(( ...
  1/2).*t.*theta))).^2+(1+(-2).*(csc((1/2).*theta).^2.*(q02.*sin((1/2).*( ...
  1+(-1).*t).*theta)+q12.*sin((1/2).*t.*theta)).^2+csc((1/2).*theta).^2.*( ...
  q03.*sin((1/2).*(1+(-1).*t).*theta)+q13.*sin((1/2).*t.*theta)).^2)).^2) ...
  .^(1/2)).*(4.*(csc((1/2).*theta).^2.*(q02.*sin((1/2).*(1+(-1).*t).* ...
  theta)+q12.*sin((1/2).*t.*theta)).*(q03.*sin((1/2).*(1+(-1).*t).*theta)+ ...
  q13.*sin((1/2).*t.*theta))+(-1).*csc((1/2).*theta).^2.*(q01.*sin((1/2).* ...
  (1+(-1).*t).*theta)+q11.*sin((1/2).*t.*theta)).*(q04.*sin((1/2).*(1+(-1) ...
  .*t).*theta)+q14.*sin((1/2).*t.*theta))).^2.*(4.*((-1).*csc((1/2).* ...
  theta).^2.*(q01.*sin((1/2).*(1+(-1).*t).*theta)+q11.*sin((1/2).*t.* ...
  theta)).*(q02.*sin((1/2).*(1+(-1).*t).*theta)+q12.*sin((1/2).*t.*theta)) ...
  +csc((1/2).*theta).^2.*(q03.*sin((1/2).*(1+(-1).*t).*theta)+q13.*sin(( ...
  1/2).*t.*theta)).*(q04.*sin((1/2).*(1+(-1).*t).*theta)+q14.*sin((1/2).* ...
  t.*theta))).^2+(1+(-2).*(csc((1/2).*theta).^2.*(q02.*sin((1/2).*(1+(-1) ...
  .*t).*theta)+q12.*sin((1/2).*t.*theta)).^2+csc((1/2).*theta).^2.*(q03.* ...
  sin((1/2).*(1+(-1).*t).*theta)+q13.*sin((1/2).*t.*theta)).^2)).^2).^(-1) ...
  .*(4.*(csc((1/2).*theta).^2.*(q01.*sin((1/2).*(1+(-1).*t).*theta)+q11.* ...
  sin((1/2).*t.*theta)).*(q03.*sin((1/2).*(1+(-1).*t).*theta)+q13.*sin(( ...
